simulink model "tracking_model"  (R2017a)
(part 4 of 14)

8076211353316)-(x_9.^2.*cos(x_4).*sin(x_3).^4.*sin(x_4).^3.*2.19560928610309e-18)./(cos(x_3).^4.*9.05902758e-4+sin(x_3).^4.*9.05902758e-4+cos(x_3).^2.*sin(x_3).^2.*1.811805516e-3)-(x_9.^2.*cos(x_5).*sin(x_3).^4.*sin(x_5).^3.*2.19560928610309e-18)./(cos(x_3).^4.*9.05902758e-4+sin(x_3).^4.*9.05902758e-4+cos(x_3).^2.*sin(x_3).^2.*1.811805516e-3)+(x_9.^2.*cos(x_6).*sin(x_3).^4.*sin(x_6).^3.*4.39121857220618e-18)./(cos(x_3).^4.*9.05902758e-4+sin(x_3).^4.*9.05902758e-4+cos(x_3).^2.*sin(x_3).^2.*1.811805516e-3)+(x_7.*x_9.*cos(x_4).*sin(x_3).^3.*sin(x_4).*4.361535375749998e-7)./(cos(x_3).^2.*6.49519052838329e-1+sin(x_3).^2.*6.49519052838329e-1)-(x_7.*x_9.*cos(x_5).*sin(x_3).^3.*sin(x_5).*2.180767687874999e-7)./(cos(x_3).^2.*6.49519052838329e-1+sin(x_3).^2.*6.49519052838329e-1)+(x_8.*x_9.*cos(x_5).*sin(x_3).^3.*sin(x_5).*3.777200434904005e-7)./(cos(x_3).^2.*6.49519052838329e-1+sin(x_3).^2.*6.49519052838329e-1)-(x_7.*x_9.*cos(x_6).*sin(x_3).^3.*sin(x_6).*2.180767687874999e-7)./(cos(x_3).^2.*6.49519052838329e-1+sin(x_3).^2.*6.49519052838329e-1)-(x_8.*x_9.*cos(x_6).*sin(x_3).^3.*sin(x_6).*3.777200434904005e-7)./(cos(x_3).^2.*6.49519052838329e-1+sin(x_3).^2.*6.49519052838329e-1)-(x_9.^2.*sin(x_4.*2.0).*cos(x_3).^2.*sin(x_3).^2.*sin(x_4).^2.*1.837631161344131e-20)./(cos(x_3).^4.*3.79080679921875e-6+sin(x_3).^4.*3.79080679921875e-6+cos(x_3).^4.*cos(x_4).^2.*6.757062187003037e-11+cos(x_3).^4.*cos(x_5).^2.*6.757062187003037e-11+cos(x_3).^4.*cos(x_6).^2.*6.757062187003037e-11+cos(x_3).^2.*sin(x_3).^2.*7.5816135984375e-6+cos(x_4).^2.*sin(x_3).^4.*6.757062187003037e-11+cos(x_5).^2.*sin(x_3).^4.*6.757062187003037e-11+cos(x_6).^2.*sin(x_3).^4.*6.757062187003037e-11+cos(x_3).^2.*cos(x_4).^2.*sin(x_3).^2.*1.351412437400607e-10+cos(x_3).^2.*cos(x_5).^2.*sin(x_3).^2.*1.351412437400607e-10+cos(x_3).^2.*cos(x_6).^2.*sin(x_3).^2.*1.351412437400607e-10)-(x_9.^2.*sin(x_4.*2.0).*cos(x_3).^2.*sin(x_3).^2.*sin(x_5).^2.*1.837631161344131e-20)./(cos(x_3).^4.*3.79080679921875e-6+sin(x_3).^4.*3.79080679921875e-6+cos(x_3).^4.*cos(x_4).^2.*6.757062187003037e-11+cos(x_3).^4.*cos(x_5).^2.*6.757062187003037e-11+cos(x_3).^4.*cos(x_6).^2.*6.757062187003037e-11+cos(x_3).^2.*sin(x_3).^2.*7.5816135984375e-6+cos(x_4).^2.*sin(x_3).^4.*6.757062187003037e-11+cos(x_5).^2.*sin(x_3).^4.*6.757062187003037e-11+cos(x_6).^2.*sin(x_3).^4.*6.757062187003037e-11+cos(x_3).^2.*cos(x_4).^2.*sin(x_3).^2.*1.351412437400607e-10+cos(x_3).^2.*cos(x_5).^2.*sin(x_3).^2.*1.351412437400607e-10+cos(x_3).^2.*cos(x_6).^2.*sin(x_3).^2.*1.351412437400607e-10)-(x_9.^2.*sin(x_5.*2.0).*cos(x_3).^2.*sin(x_3).^2.*sin(x_4).^2.*1.837631161344131e-20)./(cos(x_3).^4.*3.79080679921875e-6+sin(x_3).^4.*3.79080679921875e-6+cos(x_3).^4.*cos(x_4).^2.*6.757062187003037e-11+cos(x_3).^4.*cos(x_5).^2.*6.757062187003037e-11+cos(x_3).^4.*cos(x_6).^2.*6.757062187003037e-11+cos(x_3).^2.*sin(x_3).^2.*7.5816135984375e-6+cos(x_4).^2.*sin(x_3).^4.*6.757062187003037e-11+cos(x_5).^2.*sin(x_3).^4.*6.757062187003037e-11+cos(x_6).^2.*sin(x_3).^4.*6.757062187003037e-11+cos(x_3).^2.*cos(x_4).^2.*sin(x_3).^2.*1.351412437400607e-10+cos(x_3).^2.*cos(x_5).^2.*sin(x_3).^2.*1.351412437400607e-10+cos(x_3).^2.*cos(x_6).^2.*sin(x_3).^2.*1.351412437400607e-10)+(x_9.^2.*sin(x_4.*2.0).*cos(x_3).^2.*sin(x_3).^2.*sin(x_4).^4.*1.637688852754318e-25)./(cos(x_3).^4.*3.79080679921875e-6+sin(x_3).^4.*3.79080679921875e-6+cos(x_3).^4.*cos(x_4).^2.*6.757062187003037e-11+cos(x_3).^4.*cos(x_5).^2.*6.757062187003037e-11+cos(x_3).^4.*cos(x_6).^2.*6.757062187003037e-11+cos(x_3).^2.*sin(x_3).^2.*7.5816135984375e-6+cos(x_4).^2.*sin(x_3).^4.*6.757062187003037e-11+cos(x_5).^2.*sin(x_3).^4.*6.757062187003037e-11+cos(x_6).^2.*sin(x_3).^4.*6.757062187003037e-11+cos(x_3).^2.*cos(x_4).^2.*sin(x_3).^2.*1.351412437400607e-10+cos(x_3).^2.*cos(x_5).^2.*sin(x_3).^2.*1.351412437400607e-10+cos(x_3).^2.*cos(x_6).^2.*sin(x_3).^2.*1.351412437400607e-10)-(x_9.^2.*sin(x_4.*2.0).*cos(x_3).^2.*sin(x_3).^2.*sin(x_6).^2.*1.837631161344131e-20)./(cos(x_3).^4.*3.79080679921875e-6+sin(x_3).^4.*3.79080679921875e-6+cos(x_3).^4.*cos(x_4).^2.*6.757062187003037e-11+cos(x_3).^4.*cos(x_5).^2.*6.757062187003037e-11+cos(x_3).^4.*cos(x_6).^2.*6.757062187003037e-11+cos(x_3).^2.*sin(x_3).^2.*7.5816135984375e-6+cos(x_4).^2.*sin(x_3).^4.*6.757062187003037e-11+cos(x_5).^2.*sin(x_3).^4.*6.757062187003037e-11+cos(x_6).^2.*sin(x_3).^4.*6.757062187003037e-11+cos(x_3).^2.*cos(x_4).^2.*sin(x_3).^2.*1.351412437400607e-10+cos(x_3).^2.*cos(x_5).^2.*sin(x_3).^2.*1.351412437400607e-10+cos(x_3).^2.*cos(x_6).^2.*sin(x_3).^2.*1.351412437400607e-10)-(x_9.^2.*sin(x_5.*2.0).*cos(x_3).^2.*sin(x_3).^2.*sin(x_5).^2.*1.837631161344131e-20)./(cos(x_3).^4.*3.79080679921875e-6+sin(x_3).^4.*3.79080679921875e-6+cos(x_3).^4.*cos(x_4).^2.*6.757062187003037e-11+cos(x_3).^4.*cos(x_5).^2.*6.757062187003037e-11+cos(x_3).^4.*cos(x_6).^2.*6.757062187003037e-11+cos(x_3).^2.*sin(x_3).^2.*7.5816135984375e-6+cos(x_4).^2.*sin(x_3).^4.*6.757062187003037e-11+cos(x_5).^2.*sin(x_3).^4.*6.757062187003037e-11+cos(x_6).^2.*sin(x_3).^4.*6.757062187003037e-11+cos(x_3).^2.*cos(x_4).^2.*sin(x_3).^2.*1.351412437400607e-10+cos(x_3).^2.*cos(x_5).^2.*sin(x_3).^2.*1.351412437400607e-10+cos(x_3).^2.*cos(x_6).^2.*sin(x_3).^2.*1.351412437400607e-10)-(x_9.^2.*sin(x_6.*2.0).*cos(x_3).^2.*sin(x_3).^2.*sin(x_4).^2.*1.837631161344131e-20)./(cos(x_3).^4.*3.79080679921875e-6+sin(x_3).^4.*3.79080679921875e-6+cos(x_3).^4.*cos(x_4).^2.*6.757062187003037e-11+cos(x_3).^4.*cos(x_5).^2.*6.757062187003037e-11+cos(x_3).^4.*cos(x_6).^2.*6.757062187003037e-11+cos(x_3).^2.*sin(x_3).^2.*7.5816135984375e-6+cos(x_4).^2.*sin(x_3).^4.*6.757062187003037e-11+cos(x_5).^2.*sin(x_3).^4.*6.757062187003037e-11+cos(x_6).^2.*sin(x_3).^4.*6.757062187003037e-11+cos(x_3).^2.*cos(x_4).^2.*sin(x_3).^2.*1.351412437400607e-10+cos(x_3).^2.*cos(x_5).^2.*sin(x_3).^2.*1.351412437400607e-10+cos(x_3).^2.*cos(x_6).^2.*sin(x_3).^2.*1.351412437400607e-10)+(x_9.^2.*sin(x_4.*2.0).*cos(x_3).^2.*sin(x_3).^2.*sin(x_5).^4.*1.637688852754318e-25)./(cos(x_3).^4.*3.79080679921875e-6+sin(x_3).^4.*3.79080679921875e-6+cos(x_3).^4.*cos(x_4).^2.*6.757062187003037e-11+cos(x_3).^4.*cos(x_5).^2.*6.757062187003037e-11+cos(x_3).^4.*cos(x_6).^2.*6.757062187003037e-11+cos(x_3).^2.*sin(x_3).^2.*7.5816135984375e-6+cos(x_4).^2.*sin(x_3).^4.*6.757062187003037e-11+cos(x_5).^2.*sin(x_3).^4.*6.757062187003037e-11+cos(x_6).^2.*sin(x_3).^4.*6.757062187003037e-11+cos(x_3).^2.*cos(x_4).^2.*sin(x_3).^2.*1.351412437400607e-10+cos(x_3).^2.*cos(x_5).^2.*sin(x_3).^2.*1.351412437400607e-10+cos(x_3).^2.*cos(x_6).^2.*sin(x_3).^2.*1.351412437400607e-10)+(x_9.^2.*sin(x_5.*2.0).*cos(x_3).^2.*sin(x_3).^2.*sin(x_4).^4.*1.637688852754318e-25)./(cos(x_3).^4.*3.79080679921875e-6+sin(x_3).^4.*3.79080679921875e-6+cos(x_3).^4.*cos(x_4).^2.*6.757062187003037e-11+cos(x_3).^4.*cos(x_5).^2.*6.757062187003037e-11+cos(x_3).^4.*cos(x_6).^2.*6.757062187003037e-11+cos(x_3).^2.*sin(x_3).^2.*7.5816135984375e-6+cos(x_4).^2.*sin(x_3).^4.*6.757062187003037e-11+cos(x_5).^2.*sin(x_3).^4.*6.757062187003037e-11+cos(x_6).^2.*sin(x_3).^4.*6.757062187003037e-11+cos(x_3).^2.*cos(x_4).^2.*sin(x_3).^2.*1.351412437400607e-10+cos(x_3).^2.*cos(x_5).^2.*sin(x_3).^2.*1.351412437400607e-10+cos(x_3).^2.*cos(x_6).^2.*sin(x_3).^2.*1.351412437400607e-10)-(x_9.^2.*sin(x_5.*2.0).*cos(x_3).^2.*sin(x_3).^2.*sin(x_6).^2.*1.837631161344131e-20)./(cos(x_3).^4.*3.79080679921875e-6+sin(x_3).^4.*3.79080679921875e-6+cos(x_3).^4.*cos(x_4).^2.*6.757062187003037e-11+cos(x_3).^4.*cos(x_5).^2.*6.757062187003037e-11+cos(x_3).^4.*cos(x_6).^2.*6.757062187003037e-11+cos(x_3).^2.*sin(x_3).^2.*7.5816135984375e-6+cos(x_4).^2.*sin(x_3).^4.*6.757062187003037e-11+cos(x_5).^2.*sin(x_3).^4.*6.757062187003037e-11+cos(x_6).^2.*sin(x_3).^4.*6.757062187003037e-11+cos(x_3).^2.*cos(x_4).^2.*sin(x_3).^2.*1.351412437400607e-10+cos(x_3).^2.*cos(x_5).^2.*sin(x_3).^2.*1.351412437400607e-10+cos(x_3).^2.*cos(x_6).^2.*sin(x_3).^2.*1.351412437400607e-10)-(x_9.^2.*sin(x_6.*2.0).*cos(x_3).^2.*sin(x_3).^2.*sin(x_5).^2.*1.837631161344131e-20)./(cos(x_3).^4.*3.79080679921875e-6+sin(x_3).^4.*3.79080679921875e-6+cos(x_3).^4.*cos(x_4).^2.*6.757062187003037e-11+cos(x_3).^4.*cos(x_5).^2.*6.757062187003037e-11+cos(x_3).^4.*cos(x_6).^2.*6.757062187003037e-11+cos(x_3).^2.*sin(x_3).^2.*7.5816135984375e-6+cos(x_4).^2.*sin(x_3).^4.*6.757062187003037e-11+cos(x_5).^2.*sin(x_3).^4.*6.757062187003037e-11+cos(x_6).^2.*sin(x_3).^4.*6.757062187003037e-11+cos(x_3).^2.*cos(x_4).^2.*sin(x_3).^2.*1.351412437400607e-10+cos(x_3).^2.*cos(x_5).^2.*sin(x_3).^2.*1.351412437400607e-10+cos(x_3).^2.*cos(x_6).^2.*sin(x_3).^2.*1.351412437400607e-10)+(x_9.^2.*sin(x_4.*2.0).*cos(x_3).^2.*sin(x_3).^2.*sin(x_6).^4.*1.637688852754318e-25)./(cos(x_3).^4.*3.79080679921875e-6+sin(x_3).^4.*3.79080679921875e-6+cos(x_3).^4.*cos(x_4).^2.*6.757062187003037e-11+cos(x_3).^4.*cos(x_5).^2.*6.757062187003037e-11+cos(x_3).^4.*cos(x_6).^2.*6.757062187003037e-11+cos(x_3).^2.*sin(x_3).^2.*7.5816135984375e-6+cos(x_4).^2.*sin(x_3).^4.*6.757062187003037e-11+cos(x_5).^2.*sin(x_3).^4.*6.757062187003037e-11+cos(x_6).^2.*sin(x_3).^4.*6.757062187003037e-11+cos(x_3).^2.*cos(x_4).^2.*sin(x_3).^2.*1.351412437400607e-10+cos(x_3).^2.*cos(x_5).^2.*sin(x_3).^2.*1.351412437400607e-10+cos(x_3).^2.*cos(x_6).^2.*sin(x_3).^2.*1.351412437400607e-10)+(x_9.^2.*sin(x_4.*2.0).*cos(x_3).^4.*sin(x_4).^2.*sin(x_5).^2.*1.637688852754318e-25)./(cos(x_3).^4.*3.79080679921875e-6+sin(x_3).^4.*3.79080679921875e-6+cos(x_3).^4.*cos(x_4).^2.*6.757062187003037e-11+cos(x_3).^4.*cos(x_5).^2.*6.757062187003037e-11+cos(x_3).^4.*cos(x_6).^2.*6.757062187003037e-11+cos(x_3).^2.*sin(x_3).^2.*7.5816135984375e-6+cos(x_4).^2.*sin(x_3).^4.*6.757062187003037e-11+cos(x_5).^2.*sin(x_3).^4.*6.757062187003037e-11+cos(x_6).^2.*sin(x_3).^4.*6.757062187003037e-11+cos(x_3).^2.*cos(x_4).^2.*sin(x_3).^2.*1.351412437400607e-10+cos(x_3).^2.*cos(x_5).^2.*sin(x_3).^2.*1.351412437400607e-10+cos(x_3).^2.*cos(x_6).^2.*sin(x_3).^2.*1.351412437400607e-10)+(x_9.^2.*sin(x_5.*2.0).*cos(x_3).^2.*sin(x_3).^2.*sin(x_5).^4.*1.637688852754318e-25)./(cos(x_3).^4.*3.79080679921875e-6+sin(x_3).^4.*3.79080679921875e-6+cos(x_3).^4.*cos(x_4).^2.*6.757062187003037e-11+cos(x_3).^4.*cos(x_5).^2.*6.757062187003037e-11+cos(x_3).^4.*cos(x_6).^2.*6.757062187003037e-11+cos(x_3).^2.*sin(x_3).^2.*7.5816135984375e-6+cos(x_4).^2.*sin(x_3).^4.*6.757062187003037e-11+cos(x_5).^2.*sin(x_3).^4.*6.757062187003037e-11+cos(x_6).^2.*sin(x_3).^4.*6.757062187003037e-11+cos(x_3).^2.*cos(x_4).^2.*sin(x_3).^2.*1.351412437400607e-10+cos(x_3).^2.*cos(x_5).^2.*sin(x_3).^2.*1.351412437400607e-10+cos(x_3).^2.*cos(x_6).^2.*sin(x_3).^2.*1.351412437400607e-10)+(x_9.^2.*sin(x_6.*2.0).*cos(x_3).^2.*sin(x_3).^2.*sin(x_4).^4.*1.637688852754318e-25)./(cos(x_3).^4.*3.79080679921875e-6+sin(x_3).^4.*3.79080679921875e-6+cos(x_3).^4.*cos(x_4).^2.*6.757062187003037e-11+cos(x_3).^4.*cos(x_5).^2.*6.757062187003037e-11+cos(x_3).^4.*cos(x_6).^2.*6.757062187003037e-11+cos(x_3).^2.*sin(x_3).^2.*7.5816135984375e-6+cos(x_4).^2.*sin(x_3).^4.*6.757062187003037e-11+cos(x_5).^2.*sin(x_3).^4.*6.757062187003037e-11+cos(x_6).^2.*sin(x_3).^4.*6.757062187003037e-11+cos(x_3).^2.*cos(x_4).^2.*sin(x_3).^2.*1.351412437400607e-10+cos(x_3).^2.*cos(x_5).^2.*sin(x_3).^2.*1.351412437400607e-10+cos(x_3).^2.*cos(x_6).^2.*sin(x_3).^2.*1.351412437400607e-10)-(x_9.^2.*sin(x_6.*2.0).*cos(x_3).^2.*sin(x_3).^2.*sin(x_6).^2.*1.837631161344131e-20)./(cos(x_3).^4.*3.79080679921875e-6+sin(x_3).^4.*3.79080679921875e-6+cos(x_3).^4.*cos(x_4).^2.*6.757062187003037e-11+cos(x_3).^4.*cos(x_5).^2.*6.757062187003037e-11+cos(x_3).^4.*cos(x_6).^2.*6.757062187003037e-11+cos(x_3).^2.*sin(x_3).^2.*7.5816135984375e-6+cos(x_4).^2.*sin(x_3).^4.*6.757062187003037e-11+cos(x_5).^2.*sin(x_3).^4.*6.757062187003037e-11+cos(x_6).^2.*sin(x_3).^4.*6.757062187003037e-11+cos(x_3).^2.*cos(x_4).^2.*sin(x_3).^2.*1.351412437400607e-10+cos(x_3).^2.*cos(x_5).^2.*sin(x_3).^2.*1.351412437400607e-10+cos(x_3).^2.*cos(x_6).^2.*sin(x_3).^2.*1.351412437400607e-10)+(x_9.^2.*sin(x_4.*2.0).*cos(x_3).^4.*sin(x_4).^2.*sin(x_6).^2.*1.637688852754318e-25)./(cos(x_3).^4.*3.79080679921875e-6+sin(x_3).^4.*3.79080679921875e-6+cos(x_3).^4.*cos(x_4).^2.*6.757062187003037e-11+cos(x_3).^4.*cos(x_5).^2.*6.757062187003037e-11+cos(x_3).^4.*cos(x_6).^2.*6.757062187003037e-11+cos(x_3).^2.*sin(x_3).^2.*7.5816135984375e-6+cos(x_4).^2.*sin(x_3).^4.*6.757062187003037e-11+cos(x_5).^2.*sin(x_3).^4.*6.757062187003037e-11+cos(x_6).^2.*sin(x_3).^4.*6.757062187003037e-11+cos(x_3).^2.*cos(x_4).^2.*sin(x_3).^2.*1.351412437400607e-10+cos(x_3).^2.*cos(x_5).^2.*sin(x_3).^2.*1.351412437400607e-10+cos(x_3).^2.*cos(x_6).^2.*sin(x_3).^2.*1.351412437400607e-10)+(x_9.^2.*sin(x_5.*2.0).*cos(x_3).^2.*sin(x_3).^2.*sin(x_6).^4.*1.637688852754318e-25)./(cos(x_3).^4.*3.79080679921875e-6+sin(x_3).^4.*3.79080679921875e-6+cos(x_3).^4.*cos(x_4).^2.*6.757062187003037e-11+cos(x_3).^4.*cos(x_5).^2.*6.757062187003037e-11+cos(x_3).^4.*cos(x_6).^2.*6.757062187003037e-11+cos(x_3).^2.*sin(x_3).^2.*7.5816135984375e-6+cos(x_4).^2.*sin(x_3).^4.*6.757062187003037e-11+cos(x_5).^2.*sin(x_3).^4.*6.757062187003037e-11+cos(x_6).^2.*sin(x_3).^4.*6.757062187003037e-11+cos(x_3).^2.*cos(x_4).^2.*sin(x_3).^2.*1.351412437400607e-10+cos(x_3).^2.*cos(x_5).^2.*sin(x_3).^2.*1.351412437400607e-10+cos(x_3).^2.*cos(x_6).^2.*sin(x_3).^2.*1.351412437400607e-10)+(x_9.^2.*sin(x_5.*2.0).*cos(x_3).^4.*sin(x_4).^2.*sin(x_5).^2.*1.637688852754318e-25)./(cos(x_3).^4.*3.79080679921875e-6+sin(x_3).^4.*3.79080679921875e-6+cos(x_3).^4.*cos(x_4).^2.*6.757062187003037e-11+cos(x_3).^4.*cos(x_5).^2.*6.757062187003037e-11+cos(x_3).^4.*cos(x_6).^2.*6.757062187003037e-11+cos(x_3).^2.*sin(x_3).^2.*7.5816135984375e-6+cos(x_4).^2.*sin(x_3).^4.*6.757062187003037e-11+cos(x_5).^2.*sin(x_3).^4.*6.757062187003037e-11+cos(x_6).^2.*sin(x_3).^4.*6.757062187003037e-11+cos(x_3).^2.*cos(x_4).^2.*sin(x_3).^2.*1.351412437400607e-10+cos(x_3).^2.*cos(x_5).^2.*sin(x_3).^2.*1.351412437400607e-10+cos(x_3).^2.*cos(x_6).^2.*sin(x_3).^2.*1.351412437400607e-10)+(x_9.^2.*sin(x_6.*2.0).*cos(x_3).^2.*sin(x_3).^2.*sin(x_5).^4.*1.637688852754318e-25)./(cos(x_3).^4.*3.79080679921875e-6+sin(x_3).^4.*3.79080679921875e-6+cos(x_3).^4.*cos(x_4).^2.*6.757062187003037e-11+cos(x_3).^4.*cos(x_5).^2.*6.757062187003037e-11+cos(x_3).^4.*cos(x_6).^2.*6.757062187003037e-11+cos(x_3).^2.*sin(x_3).^2.*7.5816135984375e-6+cos(x_4).^2.*sin(x_3).^4.*6.757062187003037e-11+cos(x_5).^2.*sin(x_3).^4.*6.757062187003037e-11+cos(x_6).^2.*sin(x_3).^4.*6.757062187003037e-11+cos(x_3).^2.*cos(x_4).^2.*sin(x_3).^2.*1.351412437400607e-10+cos(x_3).^2.*cos(x_5).^2.*sin(x_3).^2.*1.351412437400607e-10+cos(x_3).^2.*cos(x_6).^2.*sin(x_3).^2.*1.351412437400607e-10)+(x_9.^2.*sin(x_4.*2.0).*cos(x_3).^4.*sin(x_5).^2.*sin(x_6).^2.*1.637688852754318e-25)./(cos(x_3).^4.*3.79080679921875e-6+sin(x_3).^4.*3.79080679921875e-6+cos(x_3).^4.*cos(x_4).^2.*6.757062187003037e-11+cos(x_3).^4.*cos(x_5).^2.*6.757062187003037e-11+cos(x_3).^4.*cos(x_6).^2.*6.757062187003037e-11+cos(x_3).^2.*sin(x_3).^2.*7.5816135984375e-6+cos(x_4).^2.*sin(x_3).^4.*6.757062187003037e-11+cos(x_5).^2.*sin(x_3).^4.*6.757062187003037e-11+cos(x_6).^2.*sin(x_3).^4.*6.757062187003037e-11+cos(x_3).^2.*cos(x_4).^2.*sin(x_3).^2.*1.351412437400607e-10+cos(x_3).^2.*cos(x_5).^2.*sin(x_3).^2.*1.351412437400607e-10+cos(x_3).^2.*cos(x_6).^2.*sin(x_3).^2.*1.351412437400607e-10)+(x_9.^2.*sin(x_5.*2.0).*cos(x_3).^4.*sin(x_4).^2.*sin(x_6).^2.*1.637688852754318e-25)./(cos(x_3).^4.*3.79080679921875e-6+sin(x_3).^4.*3.79080679921875e-6+cos(x_3).^4.*cos(x_4).^2.*6.757062187003037e-11+cos(x_3).^4.*cos(x_5).^2.*6.757062187003037e-11+cos(x_3).^4.*cos(x_6).^2.*6.757062187003037e-11+cos(x_3).^2.*sin(x_3).^2.*7.5816135984375e-6+cos(x_4).^2.*sin(x_3).^4.*6.757062187003037e-11+cos(x_5).^2.*sin(x_3).^4.*6.757062187003037e-11+cos(x_6).^2.*sin(x_3).^4.*6.757062187003037e-11+cos(x_3).^2.*cos(x_4).^2.*sin(x_3).^2.*1.351412437400607e-10+cos(x_3).^2.*cos(x_5).^2.*sin(x_3).^2.*1.351412437400607e-10+cos(x_3).^2.*cos(x_6).^2.*sin(x_3).^2.*1.351412437400607e-10)+(x_9.^2.*sin(x_6.*2.0).*cos(x_3).^2.*sin(x_3).^2.*sin(x_6).^4.*1.637688852754318e-25)./(cos(x_3).^4.*3.79080679921875e-6+sin(x_3).^4.*3.79080679921875e-6+cos(x_3).^4.*cos(x_4).^2.*6.757062187003037e-11+cos(x_3).^4.*cos(x_5).^2.*6.757062187003037e-11+cos(x_3).^4.*cos(x_6).^2.*6.757062187003037e-11+cos(x_3).^2.*sin(x_3).^2.*7.5816135984375e-6+cos(x_4).^2.*sin(x_3).^4.*6.757062187003037e-11+cos(x_5).^2.*sin(x_3).^4.*6.757062187003037e-11+cos(x_6).^2.*sin(x_3).^4.*6.757062187003037e-11+cos(x_3).^2.*cos(x_4).^2.*sin(x_3).^2.*1.351412437400607e-10+cos(x_3).^2.*cos(x_5).^2.*sin(x_3).^2.*1.351412437400607e-10+cos(x_3).^2.*cos(x_6).^2.*sin(x_3).^2.*1.351412437400607e-10)+(x_9.^2.*sin(x_6.*2.0).*cos(x_3).^4.*sin(x_4).^2.*sin(x_5).^2.*1.637688852754318e-25)./(cos(x_3).^4.*3.79080679921875e-6+sin(x_3).^4.*3.79080679921875e-6+cos(x_3).^4.*cos(x_4).^2.*6.757062187003037e-11+cos(x_3).^4.*cos(x_5).^2.*6.757062187003037e-11+cos(x_3).^4.*cos(x_6).^2.*6.757062187003037e-11+cos(x_3).^2.*sin(x_3).^2.*7.5816135984375e-6+cos(x_4).^2.*sin(x_3).^4.*6.757062187003037e-11+cos(x_5).^2.*sin(x_3).^4.*6.757062187003037e-11+cos(x_6).^2.*sin(x_3).^4.*6.757062187003037e-11+cos(x_3).^2.*cos(x_4).^2.*sin(x_3).^2.*1.351412437400607e-10+cos(x_3).^2.*cos(x_5).^2.*sin(x_3).^2.*1.351412437400607e-10+cos(x_3).^2.*cos(x_6).^2.*sin(x_3).^2.*1.351412437400607e-10)+(x_9.^2.*sin(x_5.*2.0).*cos(x_3).^4.*sin(x_5).^2.*sin(x_6).^2.*1.637688852754318e-25)./(cos(x_3).^4.*3.79080679921875e-6+sin(x_3).^4.*3.79080679921875e-6+cos(x_3).^4.*cos(x_4).^2.*6.757062187003037e-11+cos(x_3).^4.*cos(x_5).^2.*6.757062187003037e-11+cos(x_3).^4.*cos(x_6).^2.*6.757062187003037e-11+cos(x_3).^2.*sin(x_3).^2.*7.5816135984375e-6+cos(x_4).^2.*sin(x_3).^4.*6.757062187003037e-11+cos(x_5).^2.*sin(x_3).^4.*6.757062187003037e-11+cos(x_6).^2.*sin(x_3).^4.*6.757062187003037e-11+cos(x_3).^2.*cos(x_4).^2.*sin(x_3).^2.*1.351412437400607e-10+cos(x_3).^2.*cos(x_5).^2.*sin(x_3).^2.*1.351412437400607e-10+cos(x_3).^2.*cos(x_6).^2.*sin(x_3).^2.*1.351412437400607e-10)+(x_9.^2.*sin(x_6.*2.0).*cos(x_3).^4.*sin(x_4).^2.*sin(x_6).^2.*1.637688852754318e-25)./(cos(x_3).^4.*3.79080679921875e-6+sin(x_3).^4.*3.79080679921875e-6+cos(x_3).^4.*cos(x_4).^2.*6.757062187003037e-11+cos(x_3).^4.*cos(x_5).^2.*6.757062187003037e-11+cos(x_3).^4.*cos(x_6).^2.*6.757062187003037e-11+cos(x_3).^2.*sin(x_3).^2.*7.5816135984375e-6+cos(x_4).^2.*sin(x_3).^4.*6.757062187003037e-11+cos(x_5).^2.*sin(x_3).^4.*6.757062187003037e-11+cos(x_6).^2.*sin(x_3).^4.*6.757062187003037e-11+cos(x_3).^2.*cos(x_4).^2.*sin(x_3).^2.*1.351412437400607e-10+cos(x_3).^2.*cos(x_5).^2.*sin(x_3).^2.*1.351412437400607e-10+cos(x_3).^2.*cos(x_6).^2.*sin(x_3).^2.*1.351412437400607e-10)+(x_9.^2.*sin(x_6.*2.0).*cos(x_3).^4.*sin(x_5).^2.*sin(x_6).^2.*1.637688852754318e-25)./(cos(x_3).^4.*3.79080679921875e-6+sin(x_3).^4.*3.79080679921875e-6+cos(x_3).^4.*cos(x_4).^2.*6.757062187003037e-11+cos(x_3).^4.*cos(x_5).^2.*6.757062187003037e-11+cos(x_3).^4.*cos(x_6).^2.*6.757062187003037e-11+cos(x_3).^2.*sin(x_3).^2.*7.5816135984375e-6+cos(x_4).^2.*sin(x_3).^4.*6.757062187003037e-11+cos(x_5).^2.*sin(x_3).^4.*6.757062187003037e-11+cos(x_6).^2.*sin(x_3).^4.*6.757062187003037e-11+cos(x_3).^2.*cos(x_4).^2.*sin(x_3).^2.*1.351412437400607e-10+cos(x_3).^2.*cos(x_5).^2.*sin(x_3).^2.*1.351412437400607e-10+cos(x_3).^2.*cos(x_6).^2.*sin(x_3).^2.*1.351412437400607e-10)-(x_9.^2.*cos(x_3).^2.*cos(x_4).*sin(x_3).^2.*sin(x_4).^3.*4.39121857220618e-18)./(cos(x_3).^4.*9.05902758e-4+sin(x_3).^4.*9.05902758e-4+cos(x_3).^2.*sin(x_3).^2.*1.811805516e-3)-(x_9.^2.*cos(x_3).^2.*cos(x_5).*sin(x_3).^2.*sin(x_5).^3.*4.39121857220618e-18)./(cos(x_3).^4.*9.05902758e-4+sin(x_3).^4.*9.05902758e-4+cos(x_3).^2.*sin(x_3).^2.*1.811805516e-3)+(x_9.^2.*cos(x_3).^2.*cos(x_6).*sin(x_3).^2.*sin(x_6).^3.*8.782437144412361e-18)./(cos(x_3).^4.*9.05902758e-4+sin(x_3).^4.*9.05902758e-4+cos(x_3).^2.*sin(x_3).^2.*1.811805516e-3)+(x_9.^2.*sin(x_4.*2.0).*sin(x_3).^4.*sin(x_4).^2.*sin(x_5).^2.*1.637688852754318e-25)./(cos(x_3).^4.*3.79080679921875e-6+sin(x_3).^4.*3.79080679921875e-6+cos(x_3).^4.*cos(x_4).^2.*6.757062187003037e-11+cos(x_3).^4.*cos(x_5).^2.*6.757062187003037e-11+cos(x_3).^4.*cos(x_6).^2.*6.757062187003037e-11+cos(x_3).^2.*sin(x_3).^2.*7.5816135984375e-6+cos(x_4).^2.*sin(x_3).^4.*6.757062187003037e-11+cos(x_5).^2.*sin(x_3).^4.*6.757062187003037e-11+cos(x_6).^2.*sin(x_3).^4.*6.757062187003037e-11+cos(x_3).^2.*cos(x_4).^2.*sin(x_3).^2.*1.351412437400607e-10+cos(x_3).^2.*cos(x_5).^2.*sin(x_3).^2.*1.351412437400607e-10+cos(x_3).^2.*cos(x_6).^2.*sin(x_3).^2.*1.351412437400607e-10)+(x_9.^2.*sin(x_4.*2.0).*sin(x_3).^4.*sin(x_4).^2.*sin(x_6).^2.*1.637688852754318e-25)./(cos(x_3).^4.*3.79080679921875e-6+sin(x_3).^4.*3.79080679921875e-6+cos(x_3).^4.*cos(x_4).^2.*6.757062187003037e-11+cos(x_3).^4.*cos(x_5).^2.*6.757062187003037e-11+cos(x_3).^4.*cos(x_6).^2.*6.757062187003037e-11+cos(x_3).^2.*sin(x_3).^2.*7.5816135984375e-6+cos(x_4).^2.*sin(x_3).^4.*6.757062187003037e-11+cos(x_5).^2.*sin(x_3).^4.*6.757062187003037e-11+cos(x_6).^2.*sin(x_3).^4.*6.757062187003037e-11+cos(x_3).^2.*cos(x_4).^2.*sin(x_3).^2.*1.351412437400607e-10+cos(x_3).^2.*cos(x_5).^2.*sin(x_3).^2.*1.351412437400607e-10+cos(x_3).^2.*cos(x_6).^2.*sin(x_3).^2.*1.351412437400607e-10)+(x_9.^2.*sin(x_5.*2.0).*sin(x_3).^4.*sin(x_4).^2.*sin(x_5).^2.*1.637688852754318e-25)./(cos(x_3).^4.*3.79080679921875e-6+sin(x_3).^4.*3.79080679921875e-6+cos(x_3).^4.*cos(x_4).^2.*6.757062187003037e-11+cos(x_3).^4.*cos(x_5).^2.*6.757062187003037e-11+cos(x_3).^4.*cos(x_6).^2.*6.757062187003037e-11+cos(x_3).^2.*sin(x_3).^2.*7.5816135984375e-6+cos(x_4).^2.*sin(x_3).^4.*6.757062187003037e-11+cos(x_5).^2.*sin(x_3).^4.*6.757062187003037e-11+cos(x_6).^2.*sin(x_3).^4.*6.757062187003037e-11+cos(x_3).^2.*cos(x_4).^2.*sin(x_3).^2.*1.351412437400607e-10+cos(x_3).^2.*cos(x_5).^2.*sin(x_3).^2.*1.351412437400607e-10+cos(x_3).^2.*cos(x_6).^2.*sin(x_3).^2.*1.351412437400607e-10)+(x_9.^2.*sin(x_4.*2.0).*sin(x_3).^4.*sin(x_5).^2.*sin(x_6).^2.*1.637688852754318e-25)./(cos(x_3).^4.*3.79080679921875e-6+sin(x_3).^4.*3.79080679921875e-6+cos(x_3).^4.*cos(x_4).^2.*6.757062187003037e-11+cos(x_3).^4.*cos(x_5).^2.*6.757062187003037e-11+cos(x_3).^4.*cos(x_6).^2.*6.757062187003037e-11+cos(x_3).^2.*sin(x_3).^2.*7.5816135984375e-6+cos(x_4).^2.*sin(x_3).^4.*6.757062187003037e-11+cos(x_5).^2.*sin(x_3).^4.*6.757062187003037e-11+cos(x_6).^2.*sin(x_3).^4.*6.757062187003037e-11+cos(x_3).^2.*cos(x_4).^2.*sin(x_3).^2.*1.351412437400607e-10+cos(x_3).^2.*cos(x_5).^2.*sin(x_3).^2.*1.351412437400607e-10+cos(x_3).^2.*cos(x_6).^2.*sin(x_3).^2.*1.351412437400607e-10)+(x_9.^2.*sin(x_5.*2.0).*sin(x_3).^4.*sin(x_4).^2.*sin(x_6).^2.*1.637688852754318e-25)./(cos(x_3).^4.*3.79080679921875e-6+sin(x_3).^4.*3.79080679921875e-6+cos(x_3).^4.*cos(x_4).^2.*6.757062187003037e-11+cos(x_3).^4.*cos(x_5).^2.*6.757062187003037e-11+cos(x_3).^4.*cos(x_6).^2.*6.757062187003037e-11+cos(x_3).^2.*sin(x_3).^2.*7.5816135984375e-6+cos(x_4).^2.*sin(x_3).^4.*6.757062187003037e-11+cos(x_5).^2.*sin(x_3).^4.*6.757062187003037e-11+cos(x_6).^2.*sin(x_3).^4.*6.757062187003037e-11+cos(x_3).^2.*cos(x_4).^2.*sin(x_3).^2.*1.351412437400607e-10+cos(x_3).^2.*cos(x_5).^2.*sin(x_3).^2.*1.351412437400607e-10+cos(x_3).^2.*cos(x_6).^2.*sin(x_3).^2.*1.351412437400607e-10)+(x_9.^2.*sin(x_6.*2.0).*sin(x_3).^4.*sin(x_4).^2.*sin(x_5).^2.*1.637688852754318e-25)./(cos(x_3).^4.*3.79080679921875e-6+sin(x_3).^4.*3.79080679921875e-6+cos(x_3).^4.*cos(x_4).^2.*6.757062187003037e-11+cos(x_3).^4.*cos(x_5).^2.*6.757062187003037e-11+cos(x_3).^4.*cos(x_6).^2.*6.757062187003037e-11+cos(x_3).^2.*sin(x_3).^2.*7.5816135984375e-6+cos(x_4).^2.*sin(x_3).^4.*6.757062187003037e-11+cos(x_5).^2.*sin(x_3).^4.*6.757062187003037e-11+cos(x_6).^2.*sin(x_3).^4.*6.757062187003037e-11+cos(x_3).^2.*cos(x_4).^2.*sin(x_3).^2.*1.351412437400607e-10+cos(x_3).^2.*cos(x_5).^2.*sin(x_3).^2.*1.351412437400607e-10+cos(x_3).^2.*cos(x_6).^2.*sin(x_3).^2.*1.351412437400607e-10)+(x_9.^2.*sin(x_5.*2.0).*sin(x_3).^4.*sin(x_5).^2.*sin(x_6).^2.*1.637688852754318e-25)./(cos(x_3).^4.*3.79080679921875e-6+sin(x_3).^4.*3.79080679921875e-6+cos(x_3).^4.*cos(x_4).^2.*6.757062187003037e-11+cos(x_3).^4.*cos(x_5).^2.*6.757062187003037e-11+cos(x_3).^4.*cos(x_6).^2.*6.757062187003037e-11+cos(x_3).^2.*sin(x_3).^2.*7.5816135984375e-6+cos(x_4).^2.*sin(x_3).^4.*6.757062187003037e-11+cos(x_5).^2.*sin(x_3).^4.*6.757062187003037e-11+cos(x_6).^2.*sin(x_3).^4.*6.757062187003037e-11+cos(x_3).^2.*cos(x_4).^2.*sin(x_3).^2.*1.351412437400607e-10+cos(x_3).^2.*cos(x_5).^2.*sin(x_3).^2.*1.351412437400607e-10+cos(x_3).^2.*cos(x_6).^2.*sin(x_3).^2.*1.351412437400607e-10)+(x_9.^2.*sin(x_6.*2.0).*sin(x_3).^4.*sin(x_4).^2.*sin(x_6).^2.*1.637688852754318e-25)./(cos(x_3).^4.*3.79080679921875e-6+sin(x_3).^4.*3.79080679921875e-6+cos(x_3).^4.*cos(x_4).^2.*6.757062187003037e-11+cos(x_3).^4.*cos(x_5).^2.*6.757062187003037e-11+cos(x_3).^4.*cos(x_6).^2.*6.757062187003037e-11+cos(x_3).^2.*sin(x_3).^2.*7.5816135984375e-6+cos(x_4).^2.*sin(x_3).^4.*6.757062187003037e-11+cos(x_5).^2.*sin(x_3).^4.*6.757062187003037e-11+cos(x_6).^2.*sin(x_3).^4.*6.757062187003037e-11+cos(x_3).^2.*cos(x_4).^2.*sin(x_3).^2.*1.351412437400607e-10+cos(x_3).^2.*cos(x_5).^2.*sin(x_3).^2.*1.351412437400607e-10+cos(x_3).^2.*cos(x_6).^2.*sin(x_3).^2.*1.351412437400607e-10)+(x_9.^2.*sin(x_6.*2.0).*sin(x_3).^4.*sin(x_5).^2.*sin(x_6).^2.*1.637688852754318e-25)./(cos(x_3).^4.*3.79080679921875e-6+sin(x_3).^4.*3.79080679921875e-6+cos(x_3).^4.*cos(x_4).^2.*6.757062187003037e-11+cos(x_3).^4.*cos(x_5).^2.*6.757062187003037e-11+cos(x_3).^4.*cos(x_6).^2.*6.757062187003037e-11+cos(x_3).^2.*sin(x_3).^2.*7.5816135984375e-6+cos(x_4).^2.*sin(x_3).^4.*6.757062187003037e-11+cos(x_5).^2.*sin(x_3).^4.*6.757062187003037e-11+cos(x_6).^2.*sin(x_3).^4.*6.757062187003037e-11+cos(x_3).^2.*cos(x_4).^2.*sin(x_3).^2.*1.351412437400607e-10+cos(x_3).^2.*cos(x_5).^2.*sin(x_3).^2.*1.351412437400607e-10+cos(x_3).^2.*cos(x_6).^2.*sin(x_3).^2.*1.351412437400607e-10)-(x_8.*x_9.*cos(x_3).^5.*cos(x_4).*sin(x_4).^3.*1.470104929075305e-19)./(cos(x_3).^4.*3.79080679921875e-6+sin(x_3).^4.*3.79080679921875e-6+cos(x_3).^4.*cos(x_4).^2.*6.757062187003037e-11+cos(x_3).^4.*cos(x_5).^2.*6.757062187003037e-11+cos(x_3).^4.*cos(x_6).^2.*6.757062187003037e-11+cos(x_3).^2.*sin(x_3).^2.*7.5816135984375e-6+cos(x_4).^2.*sin(x_3).^4.*6.757062187003037e-11+cos(x_5).^2.*sin(x_3).^4.*6.757062187003037e-11+cos(x_6).^2.*sin(x_3).^4.*6.757062187003037e-11+cos(x_3).^2.*cos(x_4).^2.*sin(x_3).^2.*1.351412437400607e-10+cos(x_3).^2.*cos(x_5).^2.*sin(x_3).^2.*1.351412437400607e-10+cos(x_3).^2.*cos(x_6).^2.*sin(x_3).^2.*1.351412437400607e-10)+(x_7.*x_9.*cos(x_3).^5.*cos(x_5).*sin(x_5).^3.*1.273148214807934e-19)./(cos(x_3).^4.*3.79080679921875e-6+sin(x_3).^4.*3.79080679921875e-6+cos(x_3).^4.*cos(x_4).^2.*6.757062187003037e-11+cos(x_3).^4.*cos(x_5).^2.*6.757062187003037e-11+cos(x_3).^4.*cos(x_6).^2.*6.757062187003037e-11+cos(x_3).^2.*sin(x_3).^2.*7.5816135984375e-6+cos(x_4).^2.*sin(x_3).^4.*6.757062187003037e-11+cos(x_5).^2.*sin(x_3).^4.*6.757062187003037e-11+cos(x_6).^2.*sin(x_3).^4.*6.757062187003037e-11+cos(x_3).^2.*cos(x_4).^2.*sin(x_3).^2.*1.351412437400607e-10+cos(x_3).^2.*cos(x_5).^2.*sin(x_3).^2.*1.351412437400607e-10+cos(x_3).^2.*cos(x_6).^2.*sin(x_3).^2.*1.351412437400607e-10)+(x_8.*x_9.*cos(x_3).^5.*cos(x_4).*sin(x_4).^5.*1.310151082203454e-24)./(cos(x_3).^4.*3.79080679921875e-6+sin(x_3).^4.*3.79080679921875e-6+cos(x_3).^4.*cos(x_4).^2.*6.757062187003037e-11+cos(x_3).^4.*cos(x_5).^2.*6.757062187003037e-11+cos(x_3).^4.*cos(x_6).^2.*6.757062187003037e-11+cos(x_3).^2.*sin(x_3).^2.*7.5816135984375e-6+cos(x_4).^2.*sin(x_3).^4.*6.757062187003037e-11+cos(x_5).^2.*sin(x_3).^4.*6.757062187003037e-11+cos(x_6).^2.*sin(x_3).^4.*6.757062187003037e-11+cos(x_3).^2.*cos(x_4).^2.*sin(x_3).^2.*1.351412437400607e-10+cos(x_3).^2.*cos(x_5).^2.*sin(x_3).^2.*1.351412437400607e-10+cos(x_3).^2.*cos(x_6).^2.*sin(x_3).^2.*1.351412437400607e-10)+(x_8.*x_9.*cos(x_3).^5.*cos(x_5).*sin(x_5).^3.*7.350524645376524e-20)./(cos(x_3).^4.*3.79080679921875e-6+sin(x_3).^4.*3.79080679921875e-6+cos(x_3).^4.*cos(x_4).^2.*6.757062187003037e-11+cos(x_3).^4.*cos(x_5).^2.*6.757062187003037e-11+cos(x_3).^4.*cos(x_6).^2.*6.757062187003037e-11+cos(x_3).^2.*sin(x_3).^2.*7.5816135984375e-6+cos(x_4).^2.*sin(x_3).^4.*6.757062187003037e-11+cos(x_5).^2.*sin(x_3).^4.*6.757062187003037e-11+cos(x_6).^2.*sin(x_3).^4.*6.757062187003037e-11+cos(x_3).^2.*cos(x_4).^2.*sin(x_3).^2.*1.351412437400607e-10+cos(x_3).^2.*cos(x_5).^2.*sin(x_3).^2.*1.351412437400607e-10+cos(x_3).^2.*cos(x_6).^2.*sin(x_3).^2.*1.351412437400607e-10)-(x_7.*x_9.*cos(x_3).^5.*cos(x_5).*sin(x_5).^5.*1.134624119983866e-24)./(cos(x_3).^4.*3.79080679921875e-6+sin(x_3).^4.*3.79080679921875e-6+cos(x_3).^4.*cos(x_4).^2.*6.757062187003037e-11+cos(x_3).^4.*cos(x_5).^2.*6.757062187003037e-11+cos(x_3).^4.*cos(x_6).^2.*6.757062187003037e-11+cos(x_3).^2.*sin(x_3).^2.*7.5816135984375e-6+cos(x_4).^2.*sin(x_3).^4.*6.757062187003037e-11+cos(x_5).^2.*sin(x_3).^4.*6.757062187003037e-11+cos(x_6).^2.*sin(x_3).^4.*6.757062187003037e-11+cos(x_3).^2.*cos(x_4).^2.*sin(x_3).^2.*1.351412437400607e-10+cos(x_3).^2.*cos(x_5).^2.*sin(x_3).^2.*1.351412437400607e-10+cos(x_3).^2.*cos(x_6).^2.*sin(x_3).^2.*1.351412437400607e-10)-(x_7.*x_9.*cos(x_3).^5.*cos(x_6).*sin(x_6).^3.*1.273148214807934e-19)./(cos(x_3).^4.*3.79080679921875e-6+sin(x_3).^4.*3.79080679921875e-6+cos(x_3).^4.*cos(x_4).^2.*6.757062187003037e-11+cos(x_3).^4.*cos(x_5).^2.*6.757062187003037e-11+cos(x_3).^4.*cos(x_6).^2.*6.757062187003037e-11+cos(x_3).^2.*sin(x_3).^2.*7.5816135984375e-6+cos(x_4).^2.*sin(x_3).^4.*6.757062187003037e-11+cos(x_5).^2.*sin(x_3).^4.*6.757062187003037e-11+cos(x_6).^2.*sin(x_3).^4.*6.757062187003037e-11+cos(x_3).^2.*cos(x_4).^2.*sin(x_3).^2.*1.351412437400607e-10+cos(x_3).^2.*cos(x_5).^2.*sin(x_3).^2.*1.351412437400607e-10+cos(x_3).^2.*cos(x_6).^2.*sin(x_3).^2.*1.351412437400607e-10)-(x_8.*x_9.*cos(x_3).^5.*cos(x_5).*sin(x_5).^5.*6.550755411017271e-25)./(cos(x_3).^4.*3.79080679921875e-6+sin(x_3).^4.*3.79080679921875e-6+cos(x_3).^4.*cos(x_4).^2.*6.757062187003037e-11+cos(x_3).^4.*cos(x_5).^2.*6.757062187003037e-11+cos(x_3).^4.*cos(x_6).^2.*6.757062187003037e-11+cos(x_3).^2.*sin(x_3).^2.*7.5816135984375e-6+cos(x_4).^2.*sin(x_3).^4.*6.757062187003037e-11+cos(x_5).^2.*sin(x_3).^4.*6.757062187003037e-11+cos(x_6).^2.*sin(x_3).^4.*6.757062187003037e-11+cos(x_3).^2.*cos(x_4).^2.*sin(x_3).^2.*1.351412437400607e-10+cos(x_3).^2.*cos(x_5).^2.*sin(x_3).^2.*1.351412437400607e-10+cos(x_3).^2.*cos(x_6).^2.*sin(x_3).^2.*1.351412437400607e-10)+(x_8.*x_9.*cos(x_3).^5.*cos(x_6).*sin(x_6).^3.*7.350524645376524e-20)./(cos(x_3).^4.*3.79080679921875e-6+sin(x_3).^4.*3.79080679921875e-6+cos(x_3).^4.*cos(x_4).^2.*6.757062187003037e-11+cos(x_3).^4.*cos(x_5).^2.*6.757062187003037e-11+cos(x_3).^4.*cos(x_6).^2.*6.757062187003037e-11+cos(x_3).^2.*sin(x_3).^2.*7.5816135984375e-6+cos(x_4).^2.*sin(x_3).^4.*6.757062187003037e-11+cos(x_5).^2.*sin(x_3).^4.*6.757062187003037e-11+cos(x_6).^2.*sin(x_3).^4.*6.757062187003037e-11+cos(x_3).^2.*cos(x_4).^2.*sin(x_3).^2.*1.351412437400607e-10+cos(x_3).^2.*cos(x_5).^2.*sin(x_3).^2.*1.351412437400607e-10+cos(x_3).^2.*cos(x_6).^2.*sin(x_3).^2.*1.351412437400607e-10)+(x_7.*x_9.*cos(x_3).^5.*cos(x_6).*sin(x_6).^5.*1.134624119983866e-24)./(cos(x_3).^4.*3.79080679921875e-6+sin(x_3).^4.*3.79080679921875e-6+cos(x_3).^4.*cos(x_4).^2.*6.757062187003037e-11+cos(x_3).^4.*cos(x_5).^2.*6.757062187003037e-11+cos(x_3).^4.*cos(x_6).^2.*6.757062187003037e-11+cos(x_3).^2.*sin(x_3).^2.*7.5816135984375e-6+cos(x_4).^2.*sin(x_3).^4.*6.757062187003037e-11+cos(x_5).^2.*sin(x_3).^4.*6.757062187003037e-11+cos(x_6).^2.*sin(x_3).^4.*6.757062187003037e-11+cos(x_3).^2.*cos(x_4).^2.*sin(x_3).^2.*1.351412437400607e-10+cos(x_3).^2.*cos(x_5).^2.*sin(x_3).^2.*1.351412437400607e-10+cos(x_3).^2.*cos(x_6).^2.*sin(x_3).^2.*1.351412437400607e-10)-(x_8.*x_9.*cos(x_3).^5.*cos(x_6).*sin(x_6).^5.*6.550755411017271e-25)./(cos(x_3).^4.*3.79080679921875e-6+sin(x_3).^4.*3.79080679921875e-6+cos(x_3).^4.*cos(x_4).^2.*6.757062187003037e-11+cos(x_3).^4.*cos(x_5).^2.*6.757062187003037e-11+cos(x_3).^4.*cos(x_6).^2.*6.757062187003037e-11+cos(x_3).^2.*sin(x_3).^2.*7.5816135984375e-6+cos(x_4).^2.*sin(x_3).^4.*6.757062187003037e-11+cos(x_5).^2.*sin(x_3).^4.*6.757062187003037e-11+cos(x_6).^2.*sin(x_3).^4.*6.757062187003037e-11+cos(x_3).^2.*cos(x_4).^2.*sin(x_3).^2.*1.351412437400607e-10+cos(x_3).^2.*cos(x_5).^2.*sin(x_3).^2.*1.351412437400607e-10+cos(x_3).^2.*cos(x_6).^2.*sin(x_3).^2.*1.351412437400607e-10)-(x_8.*x_9.*cos(x_3).^4.*cos(x_4).*sin(x_4).^3.*4.39121857220618e-18)./(cos(x_3).^4.*1.5163227196875e-5+sin(x_3).^4.*1.5163227196875e-5+cos(x_3).^4.*cos(x_4).^2.*2.702824874801215e-10+cos(x_3).^4.*cos(x_5).^2.*2.702824874801215e-10+cos(x_3).^4.*cos(x_6).^2.*2.702824874801215e-10+cos(x_3).^2.*sin(x_3).^2.*3.032645439375e-5+cos(x_4).^2.*sin(x_3).^4.*2.702824874801215e-10+cos(x_5).^2.*sin(x_3).^4.*2.702824874801215e-10+cos(x_6).^2.*sin(x_3).^4.*2.702824874801215e-10+cos(x_3).^2.*cos(x_4).^2.*sin(x_3).^2.*5.40564974960243e-10+cos(x_3).^2.*cos(x_5).^2.*sin(x_3).^2.*5.40564974960243e-10+cos(x_3).^2.*cos(x_6).^2.*sin(x_3).^2.*5.40564974960243e-10)+(x_7.*x_9.*cos(x_3).^4.*cos(x_5).*sin(x_5).^3.*3.802906837100583e-18)./(cos(x_3).^4.*1.5163227196875e-5+sin(x_3).^4.*1.5163227196875e-5+cos(x_3).^4.*cos(x_4).^2.*2.702824874801215e-10+cos(x_3).^4.*cos(x_5).^2.*2.702824874801215e-10+cos(x_3).^4.*cos(x_6).^2.*2.702824874801215e-10+cos(x_3).^2.*sin(x_3).^2.*3.032645439375e-5+cos(x_4).^2.*sin(x_3).^4.*2.702824874801215e-10+cos(x_5).^2.*sin(x_3).^4.*2.702824874801215e-10+cos(x_6).^2.*sin(x_3).^4.*2.702824874801215e-10+cos(x_3).^2.*cos(x_4).^2.*sin(x_3).^2.*5.40564974960243e-10+cos(x_3).^2.*cos(x_5).^2.*sin(x_3).^2.*5.40564974960243e-10+cos(x_3).^2.*cos(x_6).^2.*sin(x_3).^2.*5.40564974960243e-10)+(x_8.*x_9.*cos(x_3).^4.*cos(x_5).*sin(x_5).^3.*2.19560928610309e-18)./(cos(x_3).^4.*1.5163227196875e-5+sin(x_3).^4.*1.5163227196875e-5+cos(x_3).^4.*cos(x_4).^2.*2.702824874801215e-10+cos(x_3).^4.*cos(x_5).^2.*2.702824874801215e-10+cos(x_3).^4.*cos(x_6).^2.*2.702824874801215e-10+cos(x_3).^2.*sin(x_3).^2.*3.032645439375e-5+cos(x_4).^2.*sin(x_3).^4.*2.702824874801215e-10+cos(x_5).^2.*sin(x_3).^4.*2.702824874801215e-10+cos(x_6).^2.*sin(x_3).^4.*2.702824874801215e-10+cos(x_3).^2.*cos(x_4).^2.*sin(x_3).^2.*5.40564974960243e-10+cos(x_3).^2.*cos(x_5).^2.*sin(x_3).^2.*5.40564974960243e-10+cos(x_3).^2.*cos(x_6).^2.*sin(x_3).^2.*5.40564974960243e-10)-(x_7.*x_9.*cos(x_3).^4.*cos(x_6).*sin(x_6).^3.*3.802906837100583e-18)./(cos(x_3).^4.*1.5163227196875e-5+sin(x_3).^4.*1.5163227196875e-5+cos(x_3).^4.*cos(x_4).^2.*2.702824874801215e-10+cos(x_3).^4.*cos(x_5).^2.*2.702824874801215e-10+cos(x_3).^4.*cos(x_6).^2.*2.702824874801215e-10+cos(x_3).^2.*sin(x_3).^2.*3.032645439375e-5+cos(x_4).^2.*sin(x_3).^4.*2.702824874801215e-10+cos(x_5).^2.*sin(x_3).^4.*2.702824874801215e-10+cos(x_6).^2.*sin(x_3).^4.*2.702824874801215e-10+cos(x_3).^2.*cos(x_4).^2.*sin(x_3).^2.*5.40564974960243e-10+cos(x_3).^2.*cos(x_5).^2.*sin(x_3).^2.*5.40564974960243e-10+cos(x_3).^2.*cos(x_6).^2.*sin(x_3).^2.*5.40564974960243e-10)+(x_8.*x_9.*cos(x_3).^4.*cos(x_6).*sin(x_6).^3.*2.19560928610309e-18)./(cos(x_3).^4.*1.5163227196875e-5+sin(x_3).^4.*1.5163227196875e-5+cos(x_3).^4.*cos(x_4).^2.*2.702824874801215e-10+cos(x_3).^4.*cos(x_5).^2.*2.702824874801215e-10+cos(x_3).^4.*cos(x_6).^2.*2.702824874801215e-10+cos(x_3).^2.*sin(x_3).^2.*3.032645439375e-5+cos(x_4).^2.*sin(x_3).^4.*2.702824874801215e-10+cos(x_5).^2.*sin(x_3).^4.*2.702824874801215e-10+cos(x_6).^2.*sin(x_3).^4.*2.702824874801215e-10+cos(x_3).^2.*cos(x_4).^2.*sin(x_3).^2.*5.40564974960243e-10+cos(x_3).^2.*cos(x_5).^2.*sin(x_3).^2.*5.40564974960243e-10+cos(x_3).^2.*cos(x_6).^2.*sin(x_3).^2.*5.40564974960243e-10)+(x_7.*x_9.*cos(x_4).*sin(x_3).^5.*sin(x_4).^3.*1.470104929075305e-19)./(cos(x_3).^4.*3.79080679921875e-6+sin(x_3).^4.*3.79080679921875e-6+cos(x_3).^4.*cos(x_4).^2.*6.757062187003037e-11+cos(x_3).^4.*cos(x_5).^2.*6.757062187003037e-11+cos(x_3).^4.*cos(x_6).^2.*6.757062187003037e-11+cos(x_3).^2.*sin(x_3).^2.*7.5816135984375e-6+cos(x_4).^2.*sin(x_3).^4.*6.757062187003037e-11+cos(x_5).^2.*sin(x_3).^4.*6.757062187003037e-11+cos(x_6).^2.*sin(x_3).^4.*6.757062187003037e-11+cos(x_3).^2.*cos(x_4).^2.*sin(x_3).^2.*1.351412437400607e-10+cos(x_3).^2.*cos(x_5).^2.*sin(x_3).^2.*1.351412437400607e-10+cos(x_3).^2.*cos(x_6).^2.*sin(x_3).^2.*1.351412437400607e-10)-(x_7.*x_9.*cos(x_4).*sin(x_3).^5.*sin(x_4).^5.*1.310151082203454e-24)./(cos(x_3).^4.*3.79080679921875e-6+sin(x_3).^4.*3.79080679921875e-6+cos(x_3).^4.*cos(x_4).^2.*6.757062187003037e-11+cos(x_3).^4.*cos(x_5).^2.*6.757062187003037e-11+cos(x_3).^4.*cos(x_6).^2.*6.757062187003037e-11+cos(x_3).^2.*sin(x_3).^2.*7.5816135984375e-6+cos(x_4).^2.*sin(x_3).^4.*6.757062187003037e-11+cos(x_5).^2.*sin(x_3).^4.*6.757062187003037e-11+cos(x_6).^2.*sin(x_3).^4.*6.757062187003037e-11+cos(x_3).^2.*cos(x_4).^2.*sin(x_3).^2.*1.351412437400607e-10+cos(x_3).^2.*cos(x_5).^2.*sin(x_3).^2.*1.351412437400607e-10+cos(x_3).^2.*cos(x_6).^2.*sin(x_3).^2.*1.351412437400607e-10)-(x_7.*x_9.*cos(x_5).*sin(x_3).^5.*sin(x_5).^3.*7.350524645376524e-20)./(cos(x_3).^4.*3.79080679921875e-6+sin(x_3).^4.*3.79080679921875e-6+cos(x_3).^4.*cos(x_4).^2.*6.757062187003037e-11+cos(x_3).^4.*cos(x_5).^2.*6.757062187003037e-11+cos(x_3).^4.*cos(x_6).^2.*6.757062187003037e-11+cos(x_3).^2.*sin(x_3).^2.*7.5816135984375e-6+cos(x_4).^2.*sin(x_3).^4.*6.757062187003037e-11+cos(x_5).^2.*sin(x_3).^4.*6.757062187003037e-11+cos(x_6).^2.*sin(x_3).^4.*6.757062187003037e-11+cos(x_3).^2.*cos(x_4).^2.*sin(x_3).^2.*1.351412437400607e-10+cos(x_3).^2.*cos(x_5).^2.*sin(x_3).^2.*1.351412437400607e-10+cos(x_3).^2.*cos(x_6).^2.*sin(x_3).^2.*1.351412437400607e-10)+(x_8.*x_9.*cos(x_5).*sin(x_3).^5.*sin(x_5).^3.*1.273148214807934e-19)./(cos(x_3).^4.*3.79080679921875e-6+sin(x_3).^4.*3.79080679921875e-6+cos(x_3).^4.*cos(x_4).^2.*6.757062187003037e-11+cos(x_3).^4.*cos(x_5).^2.*6.757062187003037e-11+cos(x_3).^4.*cos(x_6).^2.*6.757062187003037e-11+cos(x_3).^2.*sin(x_3).^2.*7.5816135984375e-6+cos(x_4).^2.*sin(x_3).^4.*6.757062187003037e-11+cos(x_5).^2.*sin(x_3).^4.*6.757062187003037e-11+cos(x_6).^2.*sin(x_3).^4.*6.757062187003037e-11+cos(x_3).^2.*cos(x_4).^2.*sin(x_3).^2.*1.351412437400607e-10+cos(x_3).^2.*cos(x_5).^2.*sin(x_3).^2.*1.351412437400607e-10+cos(x_3).^2.*cos(x_6).^2.*sin(x_3).^2.*1.351412437400607e-10)+(x_7.*x_9.*cos(x_5).*sin(x_3).^5.*sin(x_5).^5.*6.550755411017271e-25)./(cos(x_3).^4.*3.79080679921875e-6+sin(x_3).^4.*3.79080679921875e-6+cos(x_3).^4.*cos(x_4).^2.*6.757062187003037e-11+cos(x_3).^4.*cos(x_5).^2.*6.757062187003037e-11+cos(x_3).^4.*cos(x_6).^2.*6.757062187003037e-11+cos(x_3).^2.*sin(x_3).^2.*7.5816135984375e-6+cos(x_4).^2.*sin(x_3).^4.*6.757062187003037e-11+cos(x_5).^2.*sin(x_3).^4.*6.757062187003037e-11+cos(x_6).^2.*sin(x_3).^4.*6.757062187003037e-11+cos(x_3).^2.*cos(x_4).^2.*sin(x_3).^2.*1.351412437400607e-10+cos(x_3).^2.*cos(x_5).^2.*sin(x_3).^2.*1.351412437400607e-10+cos(x_3).^2.*cos(x_6).^2.*sin(x_3).^2.*1.351412437400607e-10)-(x_7.*x_9.*cos(x_6).*sin(x_3).^5.*sin(x_6).^3.*7.350524645376524e-20)./(cos(x_3).^4.*3.79080679921875e-6+sin(x_3).^4.*3.79080679921875e-6+cos(x_3).^4.*cos(x_4).^2.*6.757062187003037e-11+cos(x_3).^4.*cos(x_5).^2.*6.757062187003037e-11+cos(x_3).^4.*cos(x_6).^2.*6.757062187003037e-11+cos(x_3).^2.*sin(x_3).^2.*7.5816135984375e-6+cos(x_4).^2.*sin(x_3).^4.*6.757062187003037e-11+cos(x_5).^2.*sin(x_3).^4.*6.757062187003037e-11+cos(x_6).^2.*sin(x_3).^4.*6.757062187003037e-11+cos(x_3).^2.*cos(x_4).^2.*sin(x_3).^2.*1.351412437400607e-10+cos(x_3).^2.*cos(x_5).^2.*sin(x_3).^2.*1.351412437400607e-10+cos(x_3).^2.*cos(x_6).^2.*sin(x_3).^2.*1.351412437400607e-10)-(x_8.*x_9.*cos(x_5).*sin(x_3).^5.*sin(x_5).^5.*1.134624119983866e-24)./(cos(x_3).^4.*3.79080679921875e-6+sin(x_3).^4.*3.79080679921875e-6+cos(x_3).^4.*cos(x_4).^2.*6.757062187003037e-11+cos(x_3).^4.*cos(x_5).^2.*6.757062187003037e-11+cos(x_3).^4.*cos(x_6).^2.*6.757062187003037e-11+cos(x_3).^2.*sin(x_3).^2.*7.5816135984375e-6+cos(x_4).^2.*sin(x_3).^4.*6.757062187003037e-11+cos(x_5).^2.*sin(x_3).^4.*6.757062187003037e-11+cos(x_6).^2.*sin(x_3).^4.*6.757062187003037e-11+cos(x_3).^2.*cos(x_4).^2.*sin(x_3).^2.*1.351412437400607e-10+cos(x_3).^2.*cos(x_5).^2.*sin(x_3).^2.*1.351412437400607e-10+cos(x_3).^2.*cos(x_6).^2.*sin(x_3).^2.*1.351412437400607e-10)-(x_8.*x_9.*cos(x_6).*sin(x_3).^5.*sin(x_6).^3.*1.273148214807934e-19)./(cos(x_3).^4.*3.79080679921875e-6+sin(x_3).^4.*3.79080679921875e-6+cos(x_3).^4.*cos(x_4).^2.*6.757062187003037e-11+cos(x_3).^4.*cos(x_5).^2.*6.757062187003037e-11+cos(x_3).^4.*cos(x_6).^2.*6.757062187003037e-11+cos(x_3).^2.*sin(x_3).^2.*7.5816135984375e-6+cos(x_4).^2.*sin(x_3).^4.*6.757062187003037e-11+cos(x_5).^2.*sin(x_3).^4.*6.757062187003037e-11+cos(x_6).^2.*sin(x_3).^4.*6.757062187003037e-11+cos(x_3).^2.*cos(x_4).^2.*sin(x_3).^2.*1.351412437400607e-10+cos(x_3).^2.*cos(x_5).^2.*sin(x_3).^2.*1.351412437400607e-10+cos(x_3).^2.*cos(x_6).^2.*sin(x_3).^2.*1.351412437400607e-10)+(x_7.*x_9.*cos(x_6).*sin(x_3).^5.*sin(x_6).^5.*6.550755411017271e-25)./(cos(x_3).^4.*3.79080679921875e-6+sin(x_3).^4.*3.79080679921875e-6+cos(x_3).^4.*cos(x_4).^2.*6.757062187003037e-11+cos(x_3).^4.*cos(x_5).^2.*6.757062187003037e-11+cos(x_3).^4.*cos(x_6).^2.*6.757062187003037e-11+cos(x_3).^2.*sin(x_3).^2.*7.5816135984375e-6+cos(x_4).^2.*sin(x_3).^4.*6.757062187003037e-11+cos(x_5).^2.*sin(x_3).^4.*6.757062187003037e-11+cos(x_6).^2.*sin(x_3).^4.*6.757062187003037e-11+cos(x_3).^2.*cos(x_4).^2.*sin(x_3).^2.*1.351412437400607e-10+cos(x_3).^2.*cos(x_5).^2.*sin(x_3).^2.*1.351412437400607e-10+cos(x_3).^2.*cos(x_6).^2.*sin(x_3).^2.*1.351412437400607e-10)+(x_8.*x_9.*cos(x_6).*sin(x_3).^5.*sin(x_6).^5.*1.134624119983866e-24)./(cos(x_3).^4.*3.79080679921875e-6+sin(x_3).^4.*3.79080679921875e-6+cos(x_3).^4.*cos(x_4).^2.*6.757062187003037e-11+cos(x_3).^4.*cos(x_5).^2.*6.757062187003037e-11+cos(x_3).^4.*cos(x_6).^2.*6.757062187003037e-11+cos(x_3).^2.*sin(x_3).^2.*7.5816135984375e-6+cos(x_4).^2.*sin(x_3).^4.*6.757062187003037e-11+cos(x_5).^2.*sin(x_3).^4.*6.757062187003037e-11+cos(x_6).^2.*sin(x_3).^4.*6.757062187003037e-11+cos(x_3).^2.*cos(x_4).^2.*sin(x_3).^2.*1.351412437400607e-10+cos(x_3).^2.*cos(x_5).^2.*sin(x_3).^2.*1.351412437400607e-10+cos(x_3).^2.*cos(x_6).^2.*sin(x_3).^2.*1.351412437400607e-10)-(x_7.*x_9.*cos(x_4).*sin(x_3).^4.*sin(x_4).^3.*4.39121857220618e-18)./(cos(x_3).^4.*1.5163227196875e-5+sin(x_3).^4.*1.5163227196875e-5+cos(x_3).^4.*cos(x_4).^2.*2.702824874801215e-10+cos(x_3).^4.*cos(x_5).^2.*2.702824874801215e-10+cos(x_3).^4.*cos(x_6).^2.*2.702824874801215e-10+cos(x_3).^2.*sin(x_3).^2.*3.032645439375e-5+cos(x_4).^2.*sin(x_3).^4.*2.702824874801215e-10+cos(x_5).^2.*sin(x_3).^4.*2.702824874801215e-10+cos(x_6).^2.*sin(x_3).^4.*2.702824874801215e-10+cos(x_3).^2.*cos(x_4).^2.*sin(x_3).^2.*5.40564974960243e-10+cos(x_3).^2.*cos(x_5).^2.*sin(x_3).^2.*5.40564974960243e-10+cos(x_3).^2.*cos(x_6).^2.*sin(x_3).^2.*5.40564974960243e-10)+(x_7.*x_9.*cos(x_5).*sin(x_3).^4.*sin(x_5).^3.*2.19560928610309e-18)./(cos(x_3).^4.*1.5163227196875e-5+sin(x_3).^4.*1.5163227196875e-5+cos(x_3).^4.*cos(x_4).^2.*2.702824874801215e-10+cos(x_3).^4.*cos(x_5).^2.*2.702824874801215e-10+cos(x_3).^4.*cos(x_6).^2.*2.702824874801215e-10+cos(x_3).^2.*sin(x_3).^2.*3.032645439375e-5+cos(x_4).^2.*sin(x_3).^4.*2.702824874801215e-10+cos(x_5).^2.*sin(x_3).^4.*2.702824874801215e-10+cos(x_6).^2.*sin(x_3).^4.*2.702824874801215e-10+cos(x_3).^2.*cos(x_4).^2.*sin(x_3).^2.*5.40564974960243e-10+cos(x_3).^2.*cos(x_5).^2.*sin(x_3).^2.*5.40564974960243e-10+cos(x_3).^2.*cos(x_6).^2.*sin(x_3).^2.*5.40564974960243e-10)-(x_8.*x_9.*cos(x_5).*sin(x_3).^4.*sin(x_5).^3.*3.802906837100583e-18)./(cos(x_3).^4.*1.5163227196875e-5+sin(x_3).^4.*1.5163227196875e-5+cos(x_3).^4.*cos(x_4).^2.*2.702824874801215e-10+cos(x_3).^4.*cos(x_5).^2.*2.702824874801215e-10+cos(x_3).^4.*cos(x_6).^2.*2.702824874801215e-10+cos(x_3).^2.*sin(x_3).^2.*3.032645439375e-5+cos(x_4).^2.*sin(x_3).^4.*2.702824874801215e-10+cos(x_5).^2.*sin(x_3).^4.*2.702824874801215e-10+cos(x_6).^2.*sin(x_3).^4.*2.702824874801215e-10+cos(x_3).^2.*cos(x_4).^2.*sin(x_3).^2.*5.40564974960243e-10+cos(x_3).^2.*cos(x_5).^2.*sin(x_3).^2.*5.40564974960243e-10+cos(x_3).^2.*cos(x_6).^2.*sin(x_3).^2.*5.40564974960243e-10)+(x_7.*x_9.*cos(x_6).*sin(x_3).^4.*sin(x_6).^3.*2.19560928610309e-18)./(cos(x_3).^4.*1.5163227196875e-5+sin(x_3).^4.*1.5163227196875e-5+cos(x_3).^4.*cos(x_4).^2.*2.702824874801215e-10+cos(x_3).^4.*cos(x_5).^2.*2.702824874801215e-10+cos(x_3).^4.*cos(x_6).^2.*2.702824874801215e-10+cos(x_3).^2.*sin(x_3).^2.*3.032645439375e-5+cos(x_4).^2.*sin(x_3).^4.*2.702824874801215e-10+cos(x_5).^2.*sin(x_3).^4.*2.702824874801215e-10+cos(x_6).^2.*sin(x_3).^4.*2.702824874801215e-10+cos(x_3).^2.*cos(x_4).^2.*sin(x_3).^2.*5.40564974960243e-10+cos(x_3).^2.*cos(x_5).^2.*sin(x_3).^2.*5.40564974960243e-10+cos(x_3).^2.*cos(x_6).^2.*sin(x_3).^2.*5.40564974960243e-10)+(x_8.*x_9.*cos(x_6).*sin(x_3).^4.*sin(x_6).^3.*3.802906837100583e-18)./(cos(x_3).^4.*1.5163227196875e-5+sin(x_3).^4.*1.5163227196875e-5+cos(x_3).^4.*cos(x_4).^2.*2.702824874801215e-10+cos(x_3).^4.*cos(x_5).^2.*2.702824874801215e-10+cos(x_3).^4.*cos(x_6).^2.*2.702824874801215e-10+cos(x_3).^2.*sin(x_3).^2.*3.032645439375e-5+cos(x_4).^2.*sin(x_3).^4.*2.702824874801215e-10+cos(x_5).^2.*sin(x_3).^4.*2.702824874801215e-10+cos(x_6).^2.*sin(x_3).^4.*2.702824874801215e-10+cos(x_3).^2.*cos(x_4).^2.*sin(x_3).^2.*5.40564974960243e-10+cos(x_3).^2.*cos(x_5).^2.*sin(x_3).^2.*5.40564974960243e-10+cos(x_3).^2.*cos(x_6).^2.*sin(x_3).^2.*5.40564974960243e-10)+(x_9.^2.*cos(x_3).*cos(x_4).*sin(x_3).^2.*sin(x_4).*7.358998824951566e-12)./(cos(x_3).^4.*3.623611032e-3+sin(x_3).^4.*3.623611032e-3+cos(x_3).^2.*sin(x_3).^2.*7.247222064e-3)+(x_9.^2.*cos(x_3).^2.*cos(x_4).*sin(x_3).*sin(x_4).*1.471799764990313e-11)./(cos(x_3).^4.*3.623611032e-3+sin(x_3).^4.*3.623611032e-3+cos(x_3).^2.*sin(x_3).^2.*7.247222064e-3)-(x_9.^2.*cos(x_3).*cos(x_5).*sin(x_3).^2.*sin(x_5).*1.471799764990313e-11)./(cos(x_3).^4.*3.623611032e-3+sin(x_3).^4.*3.623611032e-3+cos(x_3).^2.*sin(x_3).^2.*7.247222064e-3)-(x_9.^2.*cos(x_3).^2.*cos(x_5).*sin(x_3).*sin(x_5).*7.358998824951566e-12)./(cos(x_3).^4.*3.623611032e-3+sin(x_3).^4.*3.623611032e-3+cos(x_3).^2.*sin(x_3).^2.*7.247222064e-3)+(x_9.^2.*cos(x_3).*cos(x_6).*sin(x_3).^2.*sin(x_6).*7.358998824951566e-12)./(cos(x_3).^4.*3.623611032e-3+sin(x_3).^4.*3.623611032e-3+cos(x_3).^2.*sin(x_3).^2.*7.247222064e-3)-(x_9.^2.*cos(x_3).^2.*cos(x_6).*sin(x_3).*sin(x_6).*7.358998824951566e-12)./(cos(x_3).^4.*3.623611032e-3+sin(x_3).^4.*3.623611032e-3+cos(x_3).^2.*sin(x_3).^2.*7.247222064e-3)+(th_ref.*cos(x_3).^2.*sin(x_3).^2.*sin(x_4).^2.*sin(x_5).^2.*4.839874983143591e-16)./(cos(x_3).^4.*3.628125e-2+sin(x_3).^4.*3.628125e-2+cos(x_3).^2.*sin(x_3).^2.*7.25625e-2)+(th_ref.*cos(x_3).^2.*sin(x_3).^2.*sin(x_4).^2.*sin(x_6).^2.*4.839874983143591e-16)./(cos(x_3).^4.*3.628125e-2+sin(x_3).^4.*3.628125e-2+cos(x_3).^2.*sin(x_3).^2.*7.25625e-2)+(th_ref.*cos(x_3).^2.*sin(x_3).^2.*sin(x_5).^2.*sin(x_6).^2.*4.839874983143591e-16)./(cos(x_3).^4.*3.628125e-2+sin(x_3).^4.*3.628125e-2+cos(x_3).^2.*sin(x_3).^2.*7.25625e-2)+(thp_ref.*cos(x_3).^2.*sin(x_3).^2.*sin(x_4).^2.*sin(x_5).^2.*4.839874983143591e-16)./(cos(x_3).^4.*3.628125e-2+sin(x_3).^4.*3.628125e-2+cos(x_3).^2.*sin(x_3).^2.*7.25625e-2)+(thp_ref.*cos(x_3).^2.*sin(x_3).^2.*sin(x_4).^2.*sin(x_6).^2.*4.839874983143591e-16)./(cos(x_3).^4.*3.628125e-2+sin(x_3).^4.*3.628125e-2+cos(x_3).^2.*sin(x_3).^2.*7.25625e-2)+(thp_ref.*cos(x_3).^2.*sin(x_3).^2.*sin(x_5).^2.*sin(x_6).^2.*4.839874983143591e-16)./(cos(x_3).^4.*3.628125e-2+sin(x_3).^4.*3.628125e-2+cos(x_3).^2.*sin(x_3).^2.*7.25625e-2)+(thpp_ref.*cos(x_3).^2.*sin(x_3).^2.*sin(x_4).^2.*sin(x_5).^2.*1.209968745785898e-16)./(cos(x_3).^4.*3.628125e-2+sin(x_3).^4.*3.628125e-2+cos(x_3).^2.*sin(x_3).^2.*7.25625e-2)+(thpp_ref.*cos(x_3).^2.*sin(x_3).^2.*sin(x_4).^2.*sin(x_6).^2.*1.209968745785898e-16)./(cos(x_3).^4.*3.628125e-2+sin(x_3).^4.*3.628125e-2+cos(x_3).^2.*sin(x_3).^2.*7.25625e-2)+(thpp_ref.*cos(x_3).^2.*sin(x_3).^2.*sin(x_5).^2.*sin(x_6).^2.*1.209968745785898e-16)./(cos(x_3).^4.*3.628125e-2+sin(x_3).^4.*3.628125e-2+cos(x_3).^2.*sin(x_3).^2.*7.25625e-2)-(x_3.*cos(x_3).^2.*sin(x_3).^2.*sin(x_4).^2.*sin(x_5).^2.*4.839874983143591e-16)./(cos(x_3).^4.*3.628125e-2+sin(x_3).^4.*3.628125e-2+cos(x_3).^2.*sin(x_3).^2.*7.25625e-2)-(x_3.*cos(x_3).^2.*sin(x_3).^2.*sin(x_4).^2.*sin(x_6).^2.*4.839874983143591e-16)./(cos(x_3).^4.*3.628125e-2+sin(x_3).^4.*3.628125e-2+cos(x_3).^2.*sin(x_3).^2.*7.25625e-2)-(x_3.*cos(x_3).^2.*sin(x_3).^2.*sin(x_5).^2.*sin(x_6).^2.*4.839874983143591e-16)./(cos(x_3).^4.*3.628125e-2+sin(x_3).^4.*3.628125e-2+cos(x_3).^2.*sin(x_3).^2.*7.25625e-2)-(x_9.*cos(x_3).^2.*sin(x_3).^2.*sin(x_4).^2.*sin(x_5).^2.*4.839874983143591e-16)./(cos(x_3).^4.*3.628125e-2+sin(x_3).^4.*3.628125e-2+cos(x_3).^2.*sin(x_3).^2.*7.25625e-2)-(x_9.*cos(x_3).^2.*sin(x_3).^2.*sin(x_4).^2.*sin(x_6).^2.*4.839874983143591e-16)./(cos(x_3).^4.*3.628125e-2+sin(x_3).^4.*3.628125e-2+cos(x_3).^2.*sin(x_3).^2.*7.25625e-2)-(x_9.*cos(x_3).^2.*sin(x_3).^2.*sin(x_5).^2.*sin(x_6).^2.*4.839874983143591e-16)./(cos(x_3).^4.*3.628125e-2+sin(x_3).^4.*3.628125e-2+cos(x_3).^2.*sin(x_3).^2.*7.25625e-2)-(x_9.^2.*sin(x_4.*2.0).*cos(x_3).*sin(x_3).^2.*sin(x_4).^2.*2.744511607628863e-19)./(cos(x_3).^4.*1.5163227196875e-5+sin(x_3).^4.*1.5163227196875e-5+cos(x_3).^4.*cos(x_4).^2.*2.702824874801215e-10+cos(x_3).^4.*cos(x_5).^2.*2.702824874801215e-10+cos(x_3).^4.*cos(x_6).^2.*2.702824874801215e-10+cos(x_3).^2.*sin(x_3).^2.*3.032645439375e-5+cos(x_4).^2.*sin(x_3).^4.*2.702824874801215e-10+cos(x_5).^2.*sin(x_3).^4.*2.702824874801215e-10+cos(x_6).^2.*sin(x_3).^4.*2.702824874801215e-10+cos(x_3).^2.*cos(x_4).^2.*sin(x_3).^2.*5.40564974960243e-10+cos(x_3).^2.*cos(x_5).^2.*sin(x_3).^2.*5.40564974960243e-10+cos(x_3).^2.*cos(x_6).^2.*sin(x_3).^2.*5.40564974960243e-10)+(x_9.^2.*sin(x_4.*2.0).*cos(x_3).^2.*sin(x_3).*sin(x_4).^2.*2.744511607628863e-19)./(cos(x_3).^4.*1.5163227196875e-5+sin(x_3).^4.*1.5163227196875e-5+cos(x_3).^4.*cos(x_4).^2.*2.702824874801215e-10+cos(x_3).^4.*cos(x_5).^2.*2.702824874801215e-10+cos(x_3).^4.*cos(x_6).^2.*2.702824874801215e-10+cos(x_3).^2.*sin(x_3).^2.*3.032645439375e-5+cos(x_4).^2.*sin(x_3).^4.*2.702824874801215e-10+cos(x_5).^2.*sin(x_3).^4.*2.702824874801215e-10+cos(x_6).^2.*sin(x_3).^4.*2.702824874801215e-10+cos(x_3).^2.*cos(x_4).^2.*sin(x_3).^2.*5.40564974960243e-10+cos(x_3).^2.*cos(x_5).^2.*sin(x_3).^2.*5.40564974960243e-10+cos(x_3).^2.*cos(x_6).^2.*sin(x_3).^2.*5.40564974960243e-10)-(x_9.^2.*sin(x_4.*2.0).*cos(x_3).*sin(x_3).^2.*sin(x_5).^2.*2.744511607628863e-19)./(cos(x_3).^4.*1.5163227196875e-5+sin(x_3).^4.*1.5163227196875e-5+cos(x_3).^4.*cos(x_4).^2.*2.702824874801215e-10+cos(x_3).^4.*cos(x_5).^2.*2.702824874801215e-10+cos(x_3).^4.*cos(x_6).^2.*2.702824874801215e-10+cos(x_3).^2.*sin(x_3).^2.*3.032645439375e-5+cos(x_4).^2.*sin(x_3).^4.*2.702824874801215e-10+cos(x_5).^2.*sin(x_3).^4.*2.702824874801215e-10+cos(x_6).^2.*sin(x_3).^4.*2.702824874801215e-10+cos(x_3).^2.*cos(x_4).^2.*sin(x_3).^2.*5.40564974960243e-10+cos(x_3).^2.*cos(x_5).^2.*sin(x_3).^2.*5.40564974960243e-10+cos(x_3).^2.*cos(x_6).^2.*sin(x_3).^2.*5.40564974960243e-10)+(x_9.^2.*sin(x_4.*2.0).*cos(x_3).^2.*sin(x_3).*sin(x_5).^2.*2.744511607628863e-19)./(cos(x_3).^4.*1.5163227196875e-5+sin(x_3).^4.*1.5163227196875e-5+cos(x_3).^4.*cos(x_4).^2.*2.702824874801215e-10+cos(x_3).^4.*cos(x_5).^2.*2.702824874801215e-10+cos(x_3).^4.*cos(x_6).^2.*2.702824874801215e-10+cos(x_3).^2.*sin(x_3).^2.*3.032645439375e-5+cos(x_4).^2.*sin(x_3).^4.*2.702824874801215e-10+cos(x_5).^2.*sin(x_3).^4.*2.702824874801215e-10+cos(x_6).^2.*sin(x_3).^4.*2.702824874801215e-10+cos(x_3).^2.*cos(x_4).^2.*sin(x_3).^2.*5.40564974960243e-10+cos(x_3).^2.*cos(x_5).^2.*sin(x_3).^2.*5.40564974960243e-10+cos(x_3).^2.*cos(x_6).^2.*sin(x_3).^2.*5.40564974960243e-10)-(x_9.^2.*sin(x_5.*2.0).*cos(x_3).*sin(x_3).^2.*sin(x_4).^2.*2.744511607628863e-19)./(cos(x_3).^4.*1.5163227196875e-5+sin(x_3).^4.*1.5163227196875e-5+cos(x_3).^4.*cos(x_4).^2.*2.702824874801215e-10+cos(x_3).^4.*cos(x_5).^2.*2.702824874801215e-10+cos(x_3).^4.*cos(x_6).^2.*2.702824874801215e-10+cos(x_3).^2.*sin(x_3).^2.*3.032645439375e-5+cos(x_4).^2.*sin(x_3).^4.*2.702824874801215e-10+cos(x_5).^2.*sin(x_3).^4.*2.702824874801215e-10+cos(x_6).^2.*sin(x_3).^4.*2.702824874801215e-10+cos(x_3).^2.*cos(x_4).^2.*sin(x_3).^2.*5.40564974960243e-10+cos(x_3).^2.*cos(x_5).^2.*sin(x_3).^2.*5.40564974960243e-10+cos(x_3).^2.*cos(x_6).^2.*sin(x_3).^2.*5.40564974960243e-10)+(x_9.^2.*sin(x_5.*2.0).*cos(x_3).^2.*sin(x_3).*sin(x_4).^2.*2.744511607628863e-19)./(cos(x_3).^4.*1.5163227196875e-5+sin(x_3).^4.*1.5163227196875e-5+cos(x_3).^4.*cos(x_4).^2.*2.702824874801215e-10+cos(x_3).^4.*cos(x_5).^2.*2.702824874801215e-10+cos(x_3).^4.*cos(x_6).^2.*2.702824874801215e-10+cos(x_3).^2.*sin(x_3).^2.*3.032645439375e-5+cos(x_4).^2.*sin(x_3).^4.*2.702824874801215e-10+cos(x_5).^2.*sin(x_3).^4.*2.702824874801215e-10+cos(x_6).^2.*sin(x_3).^4.*2.702824874801215e-10+cos(x_3).^2.*cos(x_4).^2.*sin(x_3).^2.*5.40564974960243e-10+cos(x_3).^2.*cos(x_5).^2.*sin(x_3).^2.*5.40564974960243e-10+cos(x_3).^2.*cos(x_6).^2.*sin(x_3).^2.*5.40564974960243e-10)-(x_9.^2.*sin(x_4.*2.0).*cos(x_3).*sin(x_3).^2.*sin(x_6).^2.*2.744511607628863e-19)./(cos(x_3).^4.*1.5163227196875e-5+sin(x_3).^4.*1.5163227196875e-5+cos(x_3).^4.*cos(x_4).^2.*2.702824874801215e-10+cos(x_3).^4.*cos(x_5).^2.*2.702824874801215e-10+cos(x_3).^4.*cos(x_6).^2.*2.702824874801215e-10+cos(x_3).^2.*sin(x_3).^2.*3.032645439375e-5+cos(x_4).^2.*sin(x_3).^4.*2.702824874801215e-10+cos(x_5).^2.*sin(x_3).^4.*2.702824874801215e-10+cos(x_6).^2.*sin(x_3).^4.*2.702824874801215e-10+cos(x_3).^2.*cos(x_4).^2.*sin(x_3).^2.*5.40564974960243e-10+cos(x_3).^2.*cos(x_5).^2.*sin(x_3).^2.*5.40564974960243e-10+cos(x_3).^2.*cos(x_6).^2.*sin(x_3).^2.*5.40564974960243e-10)+(x_9.^2.*sin(x_4.*2.0).*cos(x_3).^2.*sin(x_3).*sin(x_6).^2.*2.744511607628863e-19)./(cos(x_3).^4.*1.5163227196875e-5+sin(x_3).^4.*1.5163227196875e-5+cos(x_3).^4.*cos(x_4).^2.*2.702824874801215e-10+cos(x_3).^4.*cos(x_5).^2.*2.702824874801215e-10+cos(x_3).^4.*cos(x_6).^2.*2.702824874801215e-10+cos(x_3).^2.*sin(x_3).^2.*3.032645439375e-5+cos(x_4).^2.*sin(x_3).^4.*2.702824874801215e-10+cos(x_5).^2.*sin(x_3).^4.*2.702824874801215e-10+cos(x_6).^2.*sin(x_3).^4.*2.702824874801215e-10+cos(x_3).^2.*cos(x_4).^2.*sin(x_3).^2.*5.40564974960243e-10+cos(x_3).^2.*cos(x_5).^2.*sin(x_3).^2.*5.40564974960243e-10+cos(x_3).^2.*cos(x_6).^2.*sin(x_3).^2.*5.40564974960243e-10)-(x_9.^2.*sin(x_5.*2.0).*cos(x_3).*sin(x_3).^2.*sin(x_5).^2.*2.744511607628863e-19)./(cos(x_3).^4.*1.5163227196875e-5+sin(x_3).^4.*1.5163227196875e-5+cos(x_3).^4.*cos(x_4).^2.*2.702824874801215e-10+cos(x_3).^4.*cos(x_5).^2.*2.702824874801215e-10+cos(x_3).^4.*cos(x_6).^2.*2.702824874801215e-10+cos(x_3).^2.*sin(x_3).^2.*3.032645439375e-5+cos(x_4).^2.*sin(x_3).^4.*2.702824874801215e-10+cos(x_5).^2.*sin(x_3).^4.*2.702824874801215e-10+cos(x_6).^2.*sin(x_3).^4.*2.702824874801215e-10+cos(x_3).^2.*cos(x_4).^2.*sin(x_3).^2.*5.40564974960243e-10+cos(x_3).^2.*cos(x_5).^2.*sin(x_3).^2.*5.40564974960243e-10+cos(x_3).^2.*cos(x_6).^2.*sin(x_3).^2.*5.40564974960243e-10)+(x_9.^2.*sin(x_5.*2.0).*cos(x_3).^2.*sin(x_3).*sin(x_5).^2.*2.744511607628863e-19)./(cos(x_3).^4.*1.5163227196875e-5+sin(x_3).^4.*1.5163227196875e-5+cos(x_3).^4.*cos(x_4).^2.*2.702824874801215e-10+cos(x_3).^4.*cos(x_5).^2.*2.702824874801215e-10+cos(x_3).^4.*cos(x_6).^2.*2.702824874801215e-10+cos(x_3).^2.*sin(x_3).^2.*3.032645439375e-5+cos(x_4).^2.*sin(x_3).^4.*2.702824874801215e-10+cos(x_5).^2.*sin(x_3).^4.*2.702824874801215e-10+cos(x_6).^2.*sin(x_3).^4.*2.702824874801215e-10+cos(x_3).^2.*cos(x_4).^2.*sin(x_3).^2.*5.40564974960243e-10+cos(x_3).^2.*cos(x_5).^2.*sin(x_3).^2.*5.40564974960243e-10+cos(x_3).^2.*cos(x_6).^2.*sin(x_3).^2.*5.40564974960243e-10)-(x_9.^2.*sin(x_6.*2.0).*cos(x_3).*sin(x_3).^2.*sin(x_4).^2.*2.744511607628863e-19)./(cos(x_3).^4.*1.5163227196875e-5+sin(x_3).^4.*1.5163227196875e-5+cos(x_3).^4.*cos(x_4).^2.*2.702824874801215e-10+cos(x_3).^4.*cos(x_5).^2.*2.702824874801215e-10+cos(x_3).^4.*cos(x_6).^2.*2.702824874801215e-10+cos(x_3).^2.*sin(x_3).^2.*3.032645439375e-5+cos(x_4).^2.*sin(x_3).^4.*2.702824874801215e-10+cos(x_5).^2.*sin(x_3).^4.*2.702824874801215e-10+cos(x_6).^2.*sin(x_3).^4.*2.702824874801215e-10+cos(x_3).^2.*cos(x_4).^2.*sin(x_3).^2.*5.40564974960243e-10+cos(x_3).^2.*cos(x_5).^2.*sin(x_3).^2.*5.40564974960243e-10+cos(x_3).^2.*cos(x_6).^2.*sin(x_3).^2.*5.40564974960243e-10)+(x_9.^2.*sin(x_6.*2.0).*cos(x_3).^2.*sin(x_3).*sin(x_4).^2.*2.744511607628863e-19)./(cos(x_3).^4.*1.5163227196875e-5+sin(x_3).^4.*1.5163227196875e-5+cos(x_3).^4.*cos(x_4).^2.*2.702824874801215e-10+cos(x_3).^4.*cos(x_5).^2.*2.702824874801215e-10+cos(x_3).^4.*cos(x_6).^2.*2.702824874801215e-10+cos(x_3).^2.*sin(x_3).^2.*3.032645439375e-5+cos(x_4).^2.*sin(x_3).^4.*2.702824874801215e-10+cos(x_5).^2.*sin(x_3).^4.*2.702824874801215e-10+cos(x_6).^2.*sin(x_3).^4.*2.702824874801215e-10+cos(x_3).^2.*cos(x_4).^2.*sin(x_3).^2.*5.40564974960243e-10+cos(x_3).^2.*cos(x_5).^2.*sin(x_3).^2.*5.40564974960243e-10+cos(x_3).^2.*cos(x_6).^2.*sin(x_3).^2.*5.40564974960243e-10)-(x_9.^2.*sin(x_5.*2.0).*cos(x_3).*sin(x_3).^2.*sin(x_6).^2.*2.744511607628863e-19)./(cos(x_3).^4.*1.5163227196875e-5+sin(x_3).^4.*1.5163227196875e-5+cos(x_3).^4.*cos(x_4).^2.*2.702824874801215e-10+cos(x_3).^4.*cos(x_5).^2.*2.702824874801215e-10+cos(x_3).^4.*cos(x_6).^2.*2.702824874801215e-10+cos(x_3).^2.*sin(x_3).^2.*3.032645439375e-5+cos(x_4).^2.*sin(x_3).^4.*2.702824874801215e-10+cos(x_5).^2.*sin(x_3).^4.*2.702824874801215e-10+cos(x_6).^2.*sin(x_3).^4.*2.702824874801215e-10+cos(x_3).^2.*cos(x_4).^2.*sin(x_3).^2.*5.40564974960243e-10+cos(x_3).^2.*cos(x_5).^2.*sin(x_3).^2.*5.40564974960243e-10+cos(x_3).^2.*cos(x_6).^2.*sin(x_3).^2.*5.40564974960243e-10)+(x_9.^2.*sin(x_5.*2.0).*cos(x_3).^2.*sin(x_3).*sin(x_6).^2.*2.744511607628863e-19)./(cos(x_3).^4.*1.5163227196875e-5+sin(x_3).^4.*1.5163227196875e-5+cos(x_3).^4.*cos(x_4).^2.*2.702824874801215e-10+cos(x_3).^4.*cos(x_5).^2.*2.702824874801215e-10+cos(x_3).^4.*cos(x_6).^2.*2.702824874801215e-10+cos(x_3).^2.*sin(x_3).^2.*3.032645439375e-5+cos(x_4).^2.*sin(x_3).^4.*2.702824874801215e-10+cos(x_5).^2.*sin(x_3).^4.*2.702824874801215e-10+cos(x_6).^2.*sin(x_3).^4.*2.702824874801215e-10+cos(x_3).^2.*cos(x_4).^2.*sin(x_3).^2.*5.40564974960243e-10+cos(x_3).^2.*cos(x_5).^2.*sin(x_3).^2.*5.40564974960243e-10+cos(x_3).^2.*cos(x_6).^2.*sin(x_3).^2.*5.40564974960243e-10)-(x_9.^2.*sin(x_6.*2.0).*cos(x_3).*sin(x_3).^2.*sin(x_5).^2.*2.744511607628863e-19)./(cos(x_3).^4.*1.5163227196875e-5+sin(x_3).^4.*1.5163227196875e-5+cos(x_3).^4.*cos(x_4).^2.*2.702824874801215e-10+cos(x_3).^4.*cos(x_5).^2.*2.702824874801215e-10+cos(x_3).^4.*cos(x_6).^2.*2.702824874801215e-10+cos(x_3).^2.*sin(x_3).^2.*3.032645439375e-5+cos(x_4).^2.*sin(x_3).^4.*2.702824874801215e-10+cos(x_5).^2.*sin(x_3).^4.*2.702824874801215e-10+cos(x_6).^2.*sin(x_3).^4.*2.702824874801215e-10+cos(x_3).^2.*cos(x_4).^2.*sin(x_3).^2.*5.40564974960243e-10+cos(x_3).^2.*cos(x_5).^2.*sin(x_3).^2.*5.40564974960243e-10+cos(x_3).^2.*cos(x_6).^2.*sin(x_3).^2.*5.40564974960243e-10)+(x_9.^2.*sin(x_6.*2.0).*cos(x_3).^2.*sin(x_3).*sin(x_5).^2.*2.744511607628863e-19)./(cos(x_3).^4.*1.5163227196875e-5+sin(x_3).^4.*1.5163227196875e-5+cos(x_3).^4.*cos(x_4).^2.*2.702824874801215e-10+cos(x_3).^4.*cos(x_5).^2.*2.702824874801215e-10+cos(x_3).^4.*cos(x_6).^2.*2.702824874801215e-10+cos(x_3).^2.*sin(x_3).^2.*3.032645439375e-5+cos(x_4).^2.*sin(x_3).^4.*2.702824874801215e-10+cos(x_5).^2.*sin(x_3).^4.*2.702824874801215e-10+cos(x_6).^2.*sin(x_3).^4.*2.702824874801215e-10+cos(x_3).^2.*cos(x_4).^2.*sin(x_3).^2.*5.40564974960243e-10+cos(x_3).^2.*cos(x_5).^2.*sin(x_3).^2.*5.40564974960243e-10+cos(x_3).^2.*cos(x_6).^2.*sin(x_3).^2.*5.40564974960243e-10)-(x_9.^2.*sin(x_6.*2.0).*cos(x_3).*sin(x_3).^2.*sin(x_6).^2.*2.744511607628863e-19)./(cos(x_3).^4.*1.5163227196875e-5+sin(x_3).^4.*1.5163227196875e-5+cos(x_3).^4.*cos(x_4).^2.*2.702824874801215e-10+cos(x_3).^4.*cos(x_5).^2.*2.702824874801215e-10+cos(x_3).^4.*cos(x_6).^2.*2.702824874801215e-10+cos(x_3).^2.*sin(x_3).^2.*3.032645439375e-5+cos(x_4).^2.*sin(x_3).^4.*2.702824874801215e-10+cos(x_5).^2.*sin(x_3).^4.*2.702824874801215e-10+cos(x_6).^2.*sin(x_3).^4.*2.702824874801215e-10+cos(x_3).^2.*cos(x_4).^2.*sin(x_3).^2.*5.40564974960243e-10+cos(x_3).^2.*cos(x_5).^2.*sin(x_3).^2.*5.40564974960243e-10+cos(x_3).^2.*cos(x_6).^2.*sin(x_3).^2.*5.40564974960243e-10)+(x_9.^2.*sin(x_6.*2.0).*cos(x_3).^2.*sin(x_3).*sin(x_6).^2.*2.744511607628863e-19)./(cos(x_3).^4.*1.5163227196875e-5+sin(x_3).^4.*1.5163227196875e-5+cos(x_3).^4.*cos(x_4).^2.*2.702824874801215e-10+cos(x_3).^4.*cos(x_5).^2.*2.702824874801215e-10+cos(x_3).^4.*cos(x_6).^2.*2.702824874801215e-10+cos(x_3).^2.*sin(x_3).^2.*3.032645439375e-5+cos(x_4).^2.*sin(x_3).^4.*2.702824874801215e-10+cos(x_5).^2.*sin(x_3).^4.*2.702824874801215e-10+cos(x_6).^2.*sin(x_3).^4.*2.702824874801215e-10+cos(x_3).^2.*cos(x_4).^2.*sin(x_3).^2.*5.40564974960243e-10+cos(x_3).^2.*cos(x_5).^2.*sin(x_3).^2.*5.40564974960243e-10+cos(x_3).^2.*cos(x_6).^2.*sin(x_3).^2.*5.40564974960243e-10)+(x_9.^2.*cos(x_3).^2.*cos(x_4).*sin(x_3).^2.*sin(x_4).*2.46366703632003e-13)./(cos(x_3).^4.*9.05902758e-4+sin(x_3).^4.*9.05902758e-4+cos(x_3).^2.*sin(x_3).^2.*1.811805516e-3)+(x_9.^2.*cos(x_3).^2.*cos(x_5).*sin(x_3).^2.*sin(x_5).*2.46366703632003e-13)./(cos(x_3).^4.*9.05902758e-4+sin(x_3).^4.*9.05902758e-4+cos(x_3).^2.*sin(x_3).^2.*1.811805516e-3)-(x_9.^2.*cos(x_3).^2.*cos(x_6).*sin(x_3).^2.*sin(x_6).*4.92733407264006e-13)./(cos(x_3).^4.*9.05902758e-4+sin(x_3).^4.*9.05902758e-4+cos(x_3).^2.*sin(x_3).^2.*1.811805516e-3)-(x_9.^2.*cos(x_3).^4.*cos(x_4).*sin(x_4).*sin(x_5).^2.*2.19560928610309e-18)./(cos(x_3).^4.*9.05902758e-4+sin(x_3).^4.*9.05902758e-4+cos(x_3).^2.*sin(x_3).^2.*1.811805516e-3)-(x_9.^2.*cos(x_3).^4.*cos(x_4).*sin(x_4).*sin(x_6).^2.*2.19560928610309e-18)./(cos(x_3).^4.*9.05902758e-4+sin(x_3).^4.*9.05902758e-4+cos(x_3).^2.*sin(x_3).^2.*1.811805516e-3)-(x_9.^2.*cos(x_3).^4.*cos(x_5).*sin(x_4).^2.*sin(x_5).*2.19560928610309e-18)./(cos(x_3).^4.*9.05902758e-4+sin(x_3).^4.*9.05902758e-4+cos(x_3).^2.*sin(x_3).^2.*1.811805516e-3)-(x_9.^2.*cos(x_3).^4.*cos(x_5).*sin(x_5).*sin(x_6).^2.*2.19560928610309e-18)./(cos(x_3).^4.*9.05902758e-4+sin(x_3).^4.*9.05902758e-4+cos(x_3).^2.*sin(x_3).^2.*1.811805516e-3)+(x_9.^2.*cos(x_3).^4.*cos(x_6).*sin(x_4).^2.*sin(x_6).*4.39121857220618e-18)./(cos(x_3).^4.*9.05902758e-4+sin(x_3).^4.*9.05902758e-4+cos(x_3).^2.*sin(x_3).^2.*1.811805516e-3)+(x_9.^2.*cos(x_3).^4.*cos(x_6).*sin(x_5).^2.*sin(x_6).*4.39121857220618e-18)./(cos(x_3).^4.*9.05902758e-4+sin(x_3).^4.*9.05902758e-4+cos(x_3).^2.*sin(x_3).^2.*1.811805516e-3)-(x_9.^2.*cos(x_4).*sin(x_3).^4.*sin(x_4).*sin(x_5).^2.*2.19560928610309e-18)./(cos(x_3).^4.*9.05902758e-4+sin(x_3).^4.*9.05902758e-4+cos(x_3).^2.*sin(x_3).^2.*1.811805516e-3)-(x_9.^2.*cos(x_4).*sin(x_3).^4.*sin(x_4).*sin(x_6).^2.*2.19560928610309e-18)./(cos(x_3).^4.*9.05902758e-4+sin(x_3).^4.*9.05902758e-4+cos(x_3).^2.*sin(x_3).^2.*1.811805516e-3)-(x_9.^2.*cos(x_5).*sin(x_3).^4.*sin(x_4).^2.*sin(x_5).*2.19560928610309e-18)./(cos(x_3).^4.*9.05902758e-4+sin(x_3).^4.*9.05902758e-4+cos(x_3).^2.*sin(x_3).^2.*1.811805516e-3)-(x_9.^2.*cos(x_5).*sin(x_3).^4.*sin(x_5).*sin(x_6).^2.*2.19560928610309e-18)./(cos(x_3).^4.*9.05902758e-4+sin(x_3).^4.*9.05902758e-4+cos(x_3).^2.*sin(x_3).^2.*1.811805516e-3)+(x_9.^2.*cos(x_6).*sin(x_3).^4.*sin(x_4).^2.*sin(x_6).*4.39121857220618e-18)./(cos(x_3).^4.*9.05902758e-4+sin(x_3).^4.*9.05902758e-4+cos(x_3).^2.*sin(x_3).^2.*1.811805516e-3)+(x_9.^2.*cos(x_6).*sin(x_3).^4.*sin(x_5).^2.*sin(x_6).*4.39121857220618e-18)./(cos(x_3).^4.*9.05902758e-4+sin(x_3).^4.*9.05902758e-4+cos(x_3).^2.*sin(x_3).^2.*1.811805516e-3)+(x_8.*x_9.*cos(x_3).^5.*cos(x_4).*sin(x_4).*4.123968090108961e-15)./(cos(x_3).^4.*3.79080679921875e-6+sin(x_3).^4.*3.79080679921875e-6+cos(x_3).^4.*cos(x_4).^2.*6.757062187003037e-11+cos(x_3).^4.*cos(x_5).^2.*6.757062187003037e-11+cos(x_3).^4.*cos(x_6).^2.*6.757062187003037e-11+cos(x_3).^2.*sin(x_3).^2.*7.5816135984375e-6+cos(x_4).^2.*sin(x_3).^4.*6.757062187003037e-11+cos(x_5).^2.*sin(x_3).^4.*6.757062187003037e-11+cos(x_6).^2.*sin(x_3).^4.*6.757062187003037e-11+cos(x_3).^2.*cos(x_4).^2.*sin(x_3).^2.*1.351412437400607e-10+cos(x_3).^2.*cos(x_5).^2.*sin(x_3).^2.*1.351412437400607e-10+cos(x_3).^2.*cos(x_6).^2.*sin(x_3).^2.*1.351412437400607e-10)-(x_7.*x_9.*cos(x_3).^5.*cos(x_5).*sin(x_5).*3.571461130430754e-15)./(cos(x_3).^4.*3.79080679921875e-6+sin(x_3).^4.*3.79080679921875e-6+cos(x_3).^4.*cos(x_4).^2.*6.757062187003037e-11+cos(x_3).^4.*cos(x_5).^2.*6.757062187003037e-11+cos(x_3).^4.*cos(x_6).^2.*6.757062187003037e-11+cos(x_3).^2.*sin(x_3).^2.*7.5816135984375e-6+cos(x_4).^2.*sin(x_3).^4.*6.757062187003037e-11+cos(x_5).^2.*sin(x_3).^4.*6.757062187003037e-11+cos(x_6).^2.*sin(x_3).^4.*6.757062187003037e-11+cos(x_3).^2.*cos(x_4).^2.*sin(x_3).^2.*1.351412437400607e-10+cos(x_3).^2.*cos(x_5).^2.*sin(x_3).^2.*1.351412437400607e-10+cos(x_3).^2.*cos(x_6).^2.*sin(x_3).^2.*1.351412437400607e-10)-(x_8.*x_9.*cos(x_3).^5.*cos(x_5).*sin(x_5).*2.061984045054481e-15)./(cos(x_3).^4.*3.79080679921875e-6+sin(x_3).^4.*3.79080679921875e-6+cos(x_3).^4.*cos(x_4).^2.*6.757062187003037e-11+cos(x_3).^4.*cos(x_5).^2.*6.757062187003037e-11+cos(x_3).^4.*cos(x_6).^2.*6.757062187003037e-11+cos(x_3).^2.*sin(x_3).^2.*7.5816135984375e-6+cos(x_4).^2.*sin(x_3).^4.*6.757062187003037e-11+cos(x_5).^2.*sin(x_3).^4.*6.757062187003037e-11+cos(x_6).^2.*sin(x_3).^4.*6.757062187003037e-11+cos(x_3).^2.*cos(x_4).^2.*sin(x_3).^2.*1.351412437400607e-10+cos(x_3).^2.*cos(x_5).^2.*sin(x_3).^2.*1.351412437400607e-10+cos(x_3).^2.*cos(x_6).^2.*sin(x_3).^2.*1.351412437400607e-10)+(x_7.*x_9.*cos(x_3).^5.*cos(x_6).*sin(x_6).*3.571461130430754e-15)./(cos(x_3).^4.*3.79080679921875e-6+sin(x_3).^4.*3.79080679921875e-6+cos(x_3).^4.*cos(x_4).^2.*6.757062187003037e-11+cos(x_3).^4.*cos(x_5).^2.*6.757062187003037e-11+cos(x_3).^4.*cos(x_6).^2.*6.757062187003037e-11+cos(x_3).^2.*sin(x_3).^2.*7.5816135984375e-6+cos(x_4).^2.*sin(x_3).^4.*6.757062187003037e-11+cos(x_5).^2.*sin(x_3).^4.*6.757062187003037e-11+cos(x_6).^2.*sin(x_3).^4.*6.757062187003037e-11+cos(x_3).^2.*cos(x_4).^2.*sin(x_3).^2.*1.351412437400607e-10+cos(x_3).^2.*cos(x_5).^2.*sin(x_3).^2.*1.351412437400607e-10+cos(x_3).^2.*cos(x_6).^2.*sin(x_3).^2.*1.351412437400607e-10)-(x_8.*x_9.*cos(x_3).^5.*cos(x_6).*sin(x_6).*2.061984045054481e-15)./(cos(x_3).^4.*3.79080679921875e-6+sin(x_3).^4.*3.79080679921875e-6+cos(x_3).^4.*cos(x_4).^2.*6.757062187003037e-11+cos(x_3).^4.*cos(x_5).^2.*6.757062187003037e-11+cos(x_3).^4.*cos(x_6).^2.*6.757062187003037e-11+cos(x_3).^2.*sin(x_3).^2.*7.5816135984375e-6+cos(x_4).^2.*sin(x_3).^4.*6.757062187003037e-11+cos(x_5).^2.*sin(x_3).^4.*6.757062187003037e-11+cos(x_6).^2.*sin(x_3).^4.*6.757062187003037e-11+cos(x_3).^2.*cos(x_4).^2.*sin(x_3).^2.*1.351412437400607e-10+cos(x_3).^2.*cos(x_5).^2.*sin(x_3).^2.*1.351412437400607e-10+cos(x_3).^2.*cos(x_6).^2.*sin(x_3).^2.*1.351412437400607e-10)+(x_8.*x_9.*cos(x_3).^4.*cos(x_4).*sin(x_4).*2.46366703632003e-13)./(cos(x_3).^4.*1.5163227196875e-5+sin(x_3).^4.*1.5163227196875e-5+cos(x_3).^4.*cos(x_4).^2.*2.702824874801215e-10+cos(x_3).^4.*cos(x_5).^2.*2.702824874801215e-10+cos(x_3).^4.*cos(x_6).^2.*2.702824874801215e-10+cos(x_3).^2.*sin(x_3).^2.*3.032645439375e-5+cos(x_4).^2.*sin(x_3).^4.*2.702824874801215e-10+cos(x_5).^2.*sin(x_3).^4.*2.702824874801215e-10+cos(x_6).^2.*sin(x_3).^4.*2.702824874801215e-10+cos(x_3).^2.*cos(x_4).^2.*sin(x_3).^2.*5.40564974960243e-10+cos(x_3).^2.*cos(x_5).^2.*sin(x_3).^2.*5.40564974960243e-10+cos(x_3).^2.*cos(x_6).^2.*sin(x_3).^2.*5.40564974960243e-10)-(x_7.*x_9.*cos(x_3).^4.*cos(x_5).*sin(x_5).*2.133598239919465e-13)./(cos(x_3).^4.*1.5163227196875e-5+sin(x_3).^4.*1.5163227196875e-5+cos(x_3).^4.*cos(x_4).^2.*2.702824874801215e-10+cos(x_3).^4.*cos(x_5).^2.*2.702824874801215e-10+cos(x_3).^4.*cos(x_6).^2.*2.702824874801215e-10+cos(x_3).^2.*sin(x_3).^2.*3.032645439375e-5+cos(x_4).^2.*sin(x_3).^4.*2.702824874801215e-10+cos(x_5).^2.*sin(x_3).^4.*2.702824874801215e-10+cos(x_6).^2.*sin(x_3).^4.*2.702824874801215e-10+cos(x_3).^2.*cos(x_4).^2.*sin(x_3).^2.*5.40564974960243e-10+cos(x_3).^2.*cos(x_5).^2.*sin(x_3).^2.*5.40564974960243e-10+cos(x_3).^2.*cos(x_6).^2.*sin(x_3).^2.*5.40564974960243e-10)-(x_8.*x_9.*cos(x_3).^4.*cos(x_5).*sin(x_5).*1.231833518160015e-13)./(cos(x_3).^4.*1.5163227196875e-5+sin(x_3).^4.*1.5163227196875e-5+cos(x_3).^4.*cos(x_4).^2.*2.702824874801215e-10+cos(x_3).^4.*cos(x_5).^2.*2.702824874801215e-10+cos(x_3).^4.*cos(x_6).^2.*2.702824874801215e-10+cos(x_3).^2.*sin(x_3).^2.*3.032645439375e-5+cos(x_4).^2.*sin(x_3).^4.*2.702824874801215e-10+cos(x_5).^2.*sin(x_3).^4.*2.702824874801215e-10+cos(x_6).^2.*sin(x_3).^4.*2.702824874801215e-10+cos(x_3).^2.*cos(x_4).^2.*sin(x_3).^2.*5.40564974960243e-10+cos(x_3).^2.*cos(x_5).^2.*sin(x_3).^2.*5.40564974960243e-10+cos(x_3).^2.*cos(x_6).^2.*sin(x_3).^2.*5.40564974960243e-10)+(x_7.*x_9.*cos(x_3).^4.*cos(x_6).*sin(x_6).*2.133598239919465e-13)./(cos(x_3).^4.*1.5163227196875e-5+sin(x_3).^4.*1.5163227196875e-5+cos(x_3).^4.*cos(x_4).^2.*2.702824874801215e-10+cos(x_3).^4.*cos(x_5).^2.*2.702824874801215e-10+cos(x_3).^4.*cos(x_6).^2.*2.702824874801215e-10+cos(x_3).^2.*sin(x_3).^2.*3.032645439375e-5+cos(x_4).^2.*sin(x_3).^4.*2.702824874801215e-10+cos(x_5).^2.*sin(x_3).^4.*2.702824874801215e-10+cos(x_6).^2.*sin(x_3).^4.*2.702824874801215e-10+cos(x_3).^2.*cos(x_4).^2.*sin(x_3).^2.*5.40564974960243e-10+cos(x_3).^2.*cos(x_5).^2.*sin(x_3).^2.*5.40564974960243e-10+cos(x_3).^2.*cos(x_6).^2.*sin(x_3).^2.*5.40564974960243e-10)-(x_8.*x_9.*cos(x_3).^4.*cos(x_6).*sin(x_6).*1.231833518160015e-13)./(cos(x_3).^4.*1.5163227196875e-5+sin(x_3).^4.*1.5163227196875e-5+cos(x_3).^4.*cos(x_4).^2.*2.702824874801215e-10+cos(x_3).^4.*cos(x_5).^2.*2.702824874801215e-10+cos(x_3).^4.*cos(x_6).^2.*2.702824874801215e-10+cos(x_3).^2.*sin(x_3).^2.*3.032645439375e-5+cos(x_4).^2.*sin(x_3).^4.*2.702824874801215e-10+cos(x_5).^2.*sin(x_3).^4.*2.702824874801215e-10+cos(x_6).^2.*sin(x_3).^4.*2.702824874801215e-10+cos(x_3).^2.*cos(x_4).^2.*sin(x_3).^2.*5.40564974960243e-10+cos(x_3).^2.*cos(x_5).^2.*sin(x_3).^2.*5.40564974960243e-10+cos(x_3).^2.*cos(x_6).^2.*sin(x_3).^2.*5.40564974960243e-10)+(x_9.^2.*cos(x_3).^2.*sin(x_3).^2.*sin(x_4).^2.*sin(x_5).^2.*7.601921214217226e-61)./(cos(x_3).^4.*3.79080679921875e-6+sin(x_3).^4.*3.79080679921875e-6+cos(x_3).^4.*cos(x_4).^2.*6.757062187003037e-11+cos(x_3).^4.*cos(x_5).^2.*6.757062187003037e-11+cos(x_3).^4.*cos(x_6).^2.*6.757062187003037e-11+cos(x_3).^2.*sin(x_3).^2.*7.5816135984375e-6+cos(x_4).^2.*sin(x_3).^4.*6.757062187003037e-11+cos(x_5).^2.*sin(x_3).^4.*6.757062187003037e-11+cos(x_6).^2.*sin(x_3).^4.*6.757062187003037e-11+cos(x_3).^2.*cos(x_4).^2.*sin(x_3).^2.*1.351412437400607e-10+cos(x_3).^2.*cos(x_5).^2.*sin(x_3).^2.*1.351412437400607e-10+cos(x_3).^2.*cos(x_6).^2.*sin(x_3).^2.*1.351412437400607e-10)+(x_9.^2.*cos(x_3).^2.*sin(x_3).^2.*sin(x_4).^2.*sin(x_6).^2.*7.601921214217226e-61)./(cos(x_3).^4.*3.79080679921875e-6+sin(x_3).^4.*3.79080679921875e-6+cos(x_3).^4.*cos(x_4).^2.*6.757062187003037e-11+cos(x_3).^4.*cos(x_5).^2.*6.757062187003037e-11+cos(x_3).^4.*cos(x_6).^2.*6.757062187003037e-11+cos(x_3).^2.*sin(x_3).^2.*7.5816135984375e-6+cos(x_4).^2.*sin(x_3).^4.*6.757062187003037e-11+cos(x_5).^2.*sin(x_3).^4.*6.757062187003037e-11+cos(x_6).^2.*sin(x_3).^4.*6.757062187003037e-11+cos(x_3).^2.*cos(x_4).^2.*sin(x_3).^2.*1.351412437400607e-10+cos(x_3).^2.*cos(x_5).^2.*sin(x_3).^2.*1.351412437400607e-10+cos(x_3).^2.*cos(x_6).^2.*sin(x_3).^2.*1.351412437400607e-10)+(x_9.^2.*cos(x_3).^2.*sin(x_3).^2.*sin(x_5).^2.*sin(x_6).^2.*7.601921214217226e-61)./(cos(x_3).^4.*3.79080679921875e-6+sin(x_3).^4.*3.79080679921875e-6+cos(x_3).^4.*cos(x_4).^2.*6.757062187003037e-11+cos(x_3).^4.*cos(x_5).^2.*6.757062187003037e-11+cos(x_3).^4.*cos(x_6).^2.*6.757062187003037e-11+cos(x_3).^2.*sin(x_3).^2.*7.5816135984375e-6+cos(x_4).^2.*sin(x_3).^4.*6.757062187003037e-11+cos(x_5).^2.*sin(x_3).^4.*6.757062187003037e-11+cos(x_6).^2.*sin(x_3).^4.*6.757062187003037e-11+cos(x_3).^2.*cos(x_4).^2.*sin(x_3).^2.*1.351412437400607e-10+cos(x_3).^2.*cos(x_5).^2.*sin(x_3).^2.*1.351412437400607e-10+cos(x_3).^2.*cos(x_6).^2.*sin(x_3).^2.*1.351412437400607e-10)-(x_8.*x_9.*cos(x_3).^3.*cos(x_4).*sin(x_4).*4.361535375749998e-7)./(cos(x_3).^2.*6.49519052838329e-1+sin(x_3).^2.*6.49519052838329e-1)+(x_7.*x_9.*cos(x_3).^3.*cos(x_5).*sin(x_5).*3.777200434904005e-7)./(cos(x_3).^2.*6.49519052838329e-1+sin(x_3).^2.*6.49519052838329e-1)+(x_8.*x_9.*cos(x_3).^3.*cos(x_5).*sin(x_5).*2.180767687874999e-7)./(cos(x_3).^2.*6.49519052838329e-1+sin(x_3).^2.*6.49519052838329e-1)-(x_7.*x_9.*cos(x_3).^3.*cos(x_6).*sin(x_6).*3.777200434904005e-7)./(cos(x_3).^2.*6.49519052838329e-1+sin(x_3).^2.*6.49519052838329e-1)+(x_8.*x_9.*cos(x_3).^3.*cos(x_6).*sin(x_6).*2.180767687874999e-7)./(cos(x_3).^2.*6.49519052838329e-1+sin(x_3).^2.*6.49519052838329e-1)-(x_7.*x_9.*cos(x_4).*sin(x_3).^5.*sin(x_4).*4.123968090108961e-15)./(cos(x_3).^4.*3.79080679921875e-6+sin(x_3).^4.*3.79080679921875e-6+cos(x_3).^4.*cos(x_4).^2.*6.757062187003037e-11+cos(x_3).^4.*cos(x_5).^2.*6.757062187003037e-11+cos(x_3).^4.*cos(x_6).^2.*6.757062187003037e-11+cos(x_3).^2.*sin(x_3).^2.*7.5816135984375e-6+cos(x_4).^2.*sin(x_3).^4.*6.757062187003037e-11+cos(x_5).^2.*sin(x_3).^4.*6.757062187003037e-11+cos(x_6).^2.*sin(x_3).^4.*6.757062187003037e-11+cos(x_3).^2.*cos(x_4).^2.*sin(x_3).^2.*1.351412437400607e-10+cos(x_3).^2.*cos(x_5).^2.*sin(x_3).^2.*1.351412437400607e-10+cos(x_3).^2.*cos(x_6).^2.*sin(x_3).^2.*1.351412437400607e-10)+(x_7.*x_9.*cos(x_5).*sin(x_3).^5.*sin(x_5).*2.061984045054481e-15)./(cos(x_3).^4.*3.79080679921875e-6+sin(x_3).^4.*3.79080679921875e-6+cos(x_3).^4.*cos(x_4).^2.*6.757062187003037e-11+cos(x_3).^4.*cos(x_5).^2.*6.757062187003037e-11+cos(x_3).^4.*cos(x_6).^2.*6.757062187003037e-11+cos(x_3).^2.*sin(x_3).^2.*7.5816135984375e-6+cos(x_4).^2.*sin(x_3).^4.*6.757062187003037e-11+cos(x_5).^2.*sin(x_3).^4.*6.757062187003037e-11+cos(x_6).^2.*sin(x_3).^4.*6.757062187003037e-11+cos(x_3).^2.*cos(x_4).^2.*sin(x_3).^2.*1.351412437400607e-10+cos(x_3).^2.*cos(x_5).^2.*sin(x_3).^2.*1.351412437400607e-10+cos(x_3).^2.*cos(x_6).^2.*sin(x_3).^2.*1.351412437400607e-10)-(x_8.*x_9.*cos(x_5).*sin(x_3).^5.*sin(x_5).*3.571461130430754e-15)./(cos(x_3).^4.*3.79080679921875e-6+sin(x_3).^4.*3.79080679921875e-6+cos(x_3).^4.*cos(x_4).^2.*6.757062187003037e-11+cos(x_3).^4.*cos(x_5).^2.*6.757062187003037e-11+cos(x_3).^4.*cos(x_6).^2.*6.757062187003037e-11+cos(x_3).^2.*sin(x_3).^2.*7.5816135984375e-6+cos(x_4).^2.*sin(x_3).^4.*6.757062187003037e-11+cos(x_5).^2.*sin(x_3).^4.*6.757062187003037e-11+cos(x_6).^2.*sin(x_3).^4.*6.757062187003037e-11+cos(x_3).^2.*cos(x_4).^2.*sin(x_3).^2.*1.351412437400607e-10+cos(x_3).^2.*cos(x_5).^2.*sin(x_3).^2.*1.351412437400607e-10+cos(x_3).^2.*cos(x_6).^2.*sin(x_3).^2.*1.351412437400607e-10)+(x_7.*x_9.*cos(x_6).*sin(x_3).^5.*sin(x_6).*2.061984045054481e-15)./(cos(x_3).^4.*3.79080679921875e-6+sin(x_3).^4.*3.79080679921875e-6+cos(x_3).^4.*cos(x_4).^2.*6.757062187003037e-11+cos(x_3).^4.*cos(x_5).^2.*6.757062187003037e-11+cos(x_3).^4.*cos(x_6).^2.*6.757062187003037e-11+cos(x_3).^2.*sin(x_3).^2.*7.5816135984375e-6+cos(x_4).^2.*sin(x_3).^4.*6.757062187003037e-11+cos(x_5).^2.*sin(x_3).^4.*6.757062187003037e-11+cos(x_6).^2.*sin(x_3).^4.*6.757062187003037e-11+cos(x_3).^2.*cos(x_4).^2.*sin(x_3).^2.*1.351412437400607e-10+cos(x_3).^2.*cos(x_5).^2.*sin(x_3).^2.*1.351412437400607e-10+cos(x_3).^2.*cos(x_6).^2.*sin(x_3).^2.*1.351412437400607e-10)+(x_8.*x_9.*cos(x_6).*sin(x_3).^5.*sin(x_6).*3.571461130430754e-15)./(cos(x_3).^4.*3.79080679921875e-6+sin(x_3).^4.*3.79080679921875e-6+cos(x_3).^4.*cos(x_4).^2.*6.757062187003037e-11+cos(x_3).^4.*cos(x_5).^2.*6.757062187003037e-11+cos(x_3).^4.*cos(x_6).^2.*6.757062187003037e-11+cos(x_3).^2.*sin(x_3).^2.*7.5816135984375e-6+cos(x_4).^2.*sin(x_3).^4.*6.757062187003037e-11+cos(x_5).^2.*sin(x_3).^4.*6.757062187003037e-11+cos(x_6).^2.*sin(x_3).^4.*6.757062187003037e-11+cos(x_3).^2.*cos(x_4).^2.*sin(x_3).^2.*1.351412437400607e-10+cos(x_3).^2.*cos(x_5).^2.*sin(x_3).^2.*1.351412437400607e-10+cos(x_3).^2.*cos(x_6).^2.*sin(x_3).^2.*1.351412437400607e-10)+(x_7.*x_9.*cos(x_4).*sin(x_3).^4.*sin(x_4).*2.46366703632003e-13)./(cos(x_3).^4.*1.5163227196875e-5+sin(x_3).^4.*1.5163227196875e-5+cos(x_3).^4.*cos(x_4).^2.*2.702824874801215e-10+cos(x_3).^4.*cos(x_5).^2.*2.702824874801215e-10+cos(x_3).^4.*cos(x_6).^2.*2.702824874801215e-10+cos(x_3).^2.*sin(x_3).^2.*3.032645439375e-5+cos(x_4).^2.*sin(x_3).^4.*2.702824874801215e-10+cos(x_5).^2.*sin(x_3).^4.*2.702824874801215e-10+cos(x_6).^2.*sin(x_3).^4.*2.702824874801215e-10+cos(x_3).^2.*cos(x_4).^2.*sin(x_3).^2.*5.40564974960243e-10+cos(x_3).^2.*cos(x_5).^2.*sin(x_3).^2.*5.40564974960243e-10+cos(x_3).^2.*cos(x_6).^2.*sin(x_3).^2.*5.40564974960243e-10)-(x_7.*x_9.*cos(x_5).*sin(x_3).^4.*sin(x_5).*1.231833518160015e-13)./(cos(x_3).^4.*1.5163227196875e-5+sin(x_3).^4.*1.5163227196875e-5+cos(x_3).^4.*cos(x_4).^2.*2.702824874801215e-10+cos(x_3).^4.*cos(x_5).^2.*2.702824874801215e-10+cos(x_3).^4.*cos(x_6).^2.*2.702824874801215e-10+cos(x_3).^2.*sin(x_3).^2.*3.032645439375e-5+cos(x_4).^2.*sin(x_3).^4.*2.702824874801215e-10+cos(x_5).^2.*sin(x_3).^4.*2.702824874801215e-10+cos(x_6).^2.*sin(x_3).^4.*2.702824874801215e-10+cos(x_3).^2.*cos(x_4).^2.*sin(x_3).^2.*5.40564974960243e-10+cos(x_3).^2.*cos(x_5).^2.*sin(x_3).^2.*5.40564974960243e-10+cos(x_3).^2.*cos(x_6).^2.*sin(x_3).^2.*5.40564974960243e-10)+(x_8.*x_9.*cos(x_5).*sin(x_3).^4.*sin(x_5).*2.133598239919465e-13)./(cos(x_3).^4.*1.5163227196875e-5+sin(x_3).^4.*1.5163227196875e-5+cos(x_3).^4.*cos(x_4).^2.*2.702824874801215e-10+cos(x_3).^4.*cos(x_5).^2.*2.702824874801215e-10+cos(x_3).^4.*cos(x_6).^2.*2.702824874801215e-10+cos(x_3).^2.*sin(x_3).^2.*3.032645439375e-5+cos(x_4).^2.*sin(x_3).^4.*2.702824874801215e-10+cos(x_5).^2.*sin(x_3).^4.*2.702824874801215e-10+cos(x_6).^2.*sin(x_3).^4.*2.702824874801215e-10+cos(x_3).^2.*cos(x_4).^2.*sin(x_3).^2.*5.40564974960243e-10+cos(x_3).^2.*cos(x_5).^2.*sin(x_3).^2.*5.40564974960243e-10+cos(x_3).^2.*cos(x_6).^2.*sin(x_3).^2.*5.40564974960243e-10)-(x_7.*x_9.*cos(x_6).*sin(x_3).^4.*sin(x_6).*1.231833518160015e-13)./(cos(x_3).^4.*1.5163227196875e-5+sin(x_3).^4.*1.5163227196875e-5+cos(x_3).^4.*cos(x_4).^2.*2.702824874801215e-10+cos(x_3).^4.*cos(x_5).^2.*2.702824874801215e-10+cos(x_3).^4.*cos(x_6).^2.*2.702824874801215e-10+cos(x_3).^2.*sin(x_3).^2.*3.032645439375e-5+cos(x_4).^2.*sin(x_3).^4.*2.702824874801215e-10+cos(x_5).^2.*sin(x_3).^4.*2.702824874801215e-10+cos(x_6).^2.*sin(x_3).^4.*2.702824874801215e-10+cos(x_3).^2.*cos(x_4).^2.*sin(x_3).^2.*5.40564974960243e-10+cos(x_3).^2.*cos(x_5).^2.*sin(x_3).^2.*5.40564974960243e-10+cos(x_3).^2.*cos(x_6).^2.*sin(x_3).^2.*5.40564974960243e-10)-(x_8.*x_9.*cos(x_6).*sin(x_3).^4.*sin(x_6).*2.133598239919465e-13)./(cos(x_3).^4.*1.5163227196875e-5+sin(x_3).^4.*1.5163227196875e-5+cos(x_3).^4.*cos(x_4).^2.*2.702824874801215e-10+cos(x_3).^4.*cos(x_5).^2.*2.702824874801215e-10+cos(x_3).^4.*cos(x_6).^2.*2.702824874801215e-10+cos(x_3).^2.*sin(x_3).^2.*3.032645439375e-5+cos(x_4).^2.*sin(x_3).^4.*2.702824874801215e-10+cos(x_5).^2.*sin(x_3).^4.*2.702824874801215e-10+cos(x_6).^2.*sin(x_3).^4.*2.702824874801215e-10+cos(x_3).^2.*cos(x_4).^2.*sin(x_3).^2.*5.40564974960243e-10+cos(x_3).^2.*cos(x_5).^2.*sin(x_3).^2.*5.40564974960243e-10+cos(x_3).^2.*cos(x_6).^2.*sin(x_3).^2.*5.40564974960243e-10)-(x_9.^2.*cos(x_3).^2.*cos(x_4).*sin(x_3).^2.*sin(x_4).*sin(x_5).^2.*4.39121857220618e-18)./(cos(x_3).^4.*9.05902758e-4+sin(x_3).^4.*9.05902758e-4+cos(x_3).^2.*sin(x_3).^2.*1.811805516e-3)-(x_9.^2.*cos(x_3).^2.*cos(x_4).*sin(x_3).^2.*sin(x_4).*sin(x_6).^2.*4.39121857220618e-18)./(cos(x_3).^4.*9.05902758e-4+sin(x_3).^4.*9.05902758e-4+cos(x_3).^2.*sin(x_3).^2.*1.811805516e-3)-(x_9.^2.*cos(x_3).^2.*cos(x_5).*sin(x_3).^2.*sin(x_4).^2.*sin(x_5).*4.39121857220618e-18)./(cos(x_3).^4.*9.05902758e-4+sin(x_3).^4.*9.05902758e-4+cos(x_3).^2.*sin(x_3).^2.*1.811805516e-3)-(x_9.^2.*cos(x_3).^2.*cos(x_5).*sin(x_3).^2.*sin(x_5).*sin(x_6).^2.*4.39121857220618e-18)./(cos(x_3).^4.*9.05902758e-4+sin(x_3).^4.*9.05902758e-4+cos(x_3).^2.*sin(x_3).^2.*1.811805516e-3)+(x_9.^2.*cos(x_3).^2.*cos(x_6).*sin(x_3).^2.*sin(x_4).^2.*sin(x_6).*8.782437144412361e-18)./(cos(x_3).^4.*9.05902758e-4+sin(x_3).^4.*9.05902758e-4+cos(x_3).^2.*sin(x_3).^2.*1.811805516e-3)+(x_9.^2.*cos(x_3).^2.*cos(x_6).*sin(x_3).^2.*sin(x_5).^2.*sin(x_6).*8.782437144412361e-18)./(cos(x_3).^4.*9.05902758e-4+sin(x_3).^4.*9.05902758e-4+cos(x_3).^2.*sin(x_3).^2.*1.811805516e-3)-(x_7.*x_9.*cos(x_3).^2.*cos(x_4).*sin(x_3).^3.*sin(x_4).*8.247936180217923e-15)./(cos(x_3).^4.*3.79080679921875e-6+sin(x_3).^4.*3.79080679921875e-6+cos(x_3).^4.*cos(x_4).^2.*6.757062187003037e-11+cos(x_3).^4.*cos(x_5).^2.*6.757062187003037e-11+cos(x_3).^4.*cos(x_6).^2.*6.757062187003037e-11+cos(x_3).^2.*sin(x_3).^2.*7.5816135984375e-6+cos(x_4).^2.*sin(x_3).^4.*6.757062187003037e-11+cos(x_5).^2.*sin(x_3).^4.*6.757062187003037e-11+cos(x_6).^2.*sin(x_3).^4.*6.757062187003037e-11+cos(x_3).^2.*cos(x_4).^2.*sin(x_3).^2.*1.351412437400607e-10+cos(x_3).^2.*cos(x_5).^2.*sin(x_3).^2.*1.351412437400607e-10+cos(x_3).^2.*cos(x_6).^2.*sin(x_3).^2.*1.351412437400607e-10)+(x_8.*x_9.*cos(x_3).^3.*cos(x_4).*sin(x_3).^2.*sin(x_4).*8.247936180217923e-15)./(cos(x_3).^4.*3.79080679921875e-6+sin(x_3).^4.*3.79080679921875e-6+cos(x_3).^4.*cos(x_4).^2.*6.757062187003037e-11+cos(x_3).^4.*cos(x_5).^2.*6.757062187003037e-11+cos(x_3).^4.*cos(x_6).^2.*6.757062187003037e-11+cos(x_3).^2.*sin(x_3).^2.*7.5816135984375e-6+cos(x_4).^2.*sin(x_3).^4.*6.757062187003037e-11+cos(x_5).^2.*sin(x_3).^4.*6.757062187003037e-11+cos(x_6).^2.*sin(x_3).^4.*6.757062187003037e-11+cos(x_3).^2.*cos(x_4).^2.*sin(x_3).^2.*1.351412437400607e-10+cos(x_3).^2.*cos(x_5).^2.*sin(x_3).^2.*1.351412437400607e-10+cos(x_3).^2.*cos(x_6).^2.*sin(x_3).^2.*1.351412437400607e-10)+(x_7.*x_9.*cos(x_3).^2.*cos(x_5).*sin(x_3).^3.*sin(x_5).*4.123968090108961e-15)./(cos(x_3).^4.*3.79080679921875e-6+sin(x_3).^4.*3.79080679921875e-6+cos(x_3).^4.*cos(x_4).^2.*6.757062187003037e-11+cos(x_3).^4.*cos(x_5).^2.*6.757062187003037e-11+cos(x_3).^4.*cos(x_6).^2.*6.757062187003037e-11+cos(x_3).^2.*sin(x_3).^2.*7.5816135984375e-6+cos(x_4).^2.*sin(x_3).^4.*6.757062187003037e-11+cos(x_5).^2.*sin(x_3).^4.*6.757062187003037e-11+cos(x_6).^2.*sin(x_3).^4.*6.757062187003037e-11+cos(x_3).^2.*cos(x_4).^2.*sin(x_3).^2.*1.351412437400607e-10+cos(x_3).^2.*cos(x_5).^2.*sin(x_3).^2.*1.351412437400607e-10+cos(x_3).^2.*cos(x_6).^2.*sin(x_3).^2.*1.351412437400607e-10)-(x_7.*x_9.*cos(x_3).^3.*cos(x_5).*sin(x_3).^2.*sin(x_5).*7.142922260861507e-15)./(cos(x_3).^4.*3.79080679921875e-6+sin(x_3).^4.*3.79080679921875e-6+cos(x_3).^4.*cos(x_4).^2.*6.757062187003037e-11+cos(x_3).^4.*cos(x_5).^2.*6.757062187003037e-11+cos(x_3).^4.*cos(x_6).^2.*6.757062187003037e-11+cos(x_3).^2.*sin(x_3).^2.*7.5816135984375e-6+cos(x_4).^2.*sin(x_3).^4.*6.757062187003037e-11+cos(x_5).^2.*sin(x_3).^4.*6.757062187003037e-11+cos(x_6).^2.*sin(x_3).^4.*6.757062187003037e-11+cos(x_3).^2.*cos(x_4).^2.*sin(x_3).^2.*1.351412437400607e-10+cos(x_3).^2.*cos(x_5).^2.*sin(x_3).^2.*1.351412437400607e-10+cos(x_3).^2.*cos(x_6).^2.*sin(x_3).^2.*1.351412437400607e-10)+(x_7.*x_9.*cos(x_3).^4.*cos(x_4).*sin(x_3).*sin(x_4).^3.*1.470104929075305e-19)./(cos(x_3).^4.*3.79080679921875e-6+sin(x_3).^4.*3.79080679921875e-6+cos(x_3).^4.*cos(x_4).^2.*6.757062187003037e-11+cos(x_3).^4.*cos(x_5).^2.*6.757062187003037e-11+cos(x_3).^4.*cos(x_6).^2.*6.757062187003037e-11+cos(x_3).^2.*sin(x_3).^2.*7.5816135984375e-6+cos(x_4).^2.*sin(x_3).^4.*6.757062187003037e-11+cos(x_5).^2.*sin(x_3).^4.*6.757062187003037e-11+cos(x_6).^2.*sin(x_3).^4.*6.757062187003037e-11+cos(x_3).^2.*cos(x_4).^2.*sin(x_3).^2.*1.351412437400607e-10+cos(x_3).^2.*cos(x_5).^2.*sin(x_3).^2.*1.351412437400607e-10+cos(x_3).^2.*cos(x_6).^2.*sin(x_3).^2.*1.351412437400607e-10)-(x_8.*x_9.*cos(x_3).*cos(x_4).*sin(x_3).^4.*sin(x_4).^3.*1.470104929075305e-19)./(cos(x_3).^4.*3.79080679921875e-6+sin(x_3).^4.*3.79080679921875e-6+cos(x_3).^4.*cos(x_4).^2.*6.757062187003037e-11+cos(x_3).^4.*cos(x_5).^2.*6.757062187003037e-11+cos(x_3).^4.*cos(x_6).^2.*6.757062187003037e-11+cos(x_3).^2.*sin(x_3).^2.*7.5816135984375e-6+cos(x_4).^2.*sin(x_3).^4.*6.757062187003037e-11+cos(x_5).^2.*sin(x_3).^4.*6.757062187003037e-11+cos(x_6).^2.*sin(x_3).^4.*6.757062187003037e-11+cos(x_3).^2.*cos(x_4).^2.*sin(x_3).^2.*1.351412437400607e-10+cos(x_3).^2.*cos(x_5).^2.*sin(x_3).^2.*1.351412437400607e-10+cos(x_3).^2.*cos(x_6).^2.*sin(x_3).^2.*1.351412437400607e-10)-(x_8.*x_9.*cos(x_3).^2.*cos(x_5).*sin(x_3).^3.*sin(x_5).*7.142922260861507e-15)./(cos(x_3).^4.*3.79080679921875e-6+sin(x_3).^4.*3.79080679921875e-6+cos(x_3).^4.*cos(x_4).^2.*6.757062187003037e-11+cos(x_3).^4.*cos(x_5).^2.*6.757062187003037e-11+cos(x_3).^4.*cos(x_6).^2.*6.757062187003037e-11+cos(x_3).^2.*sin(x_3).^2.*7.5816135984375e-6+cos(x_4).^2.*sin(x_3).^4.*6.757062187003037e-11+cos(x_5).^2.*sin(x_3).^4.*6.757062187003037e-11+cos(x_6).^2.*sin(x_3).^4.*6.757062187003037e-11+cos(x_3).^2.*cos(x_4).^2.*sin(x_3).^2.*1.351412437400607e-10+cos(x_3).^2.*cos(x_5).^2.*sin(x_3).^2.*1.351412437400607e-10+cos(x_3).^2.*cos(x_6).^2.*sin(x_3).^2.*1.351412437400607e-10)-(x_8.*x_9.*cos(x_3).^3.*cos(x_5).*sin(x_3).^2.*sin(x_5).*4.123968090108961e-15)./(cos(x_3).^4.*3.79080679921875e-6+sin(x_3).^4.*3.79080679921875e-6+cos(x_3).^4.*cos(x_4).^2.*6.757062187003037e-11+cos(x_3).^4.*cos(x_5).^2.*6.757062187003037e-11+cos(x_3).^4.*cos(x_6).^2.*6.757062187003037e-11+cos(x_3).^2.*sin(x_3).^2.*7.5816135984375e-6+cos(x_4).^2.*sin(x_3).^4.*6.757062187003037e-11+cos(x_5).^2.*sin(x_3).^4.*6.757062187003037e-11+cos(x_6).^2.*sin(x_3).^4.*6.757062187003037e-11+cos(x_3).^2.*cos(x_4).^2.*sin(x_3).^2.*1.351412437400607e-10+cos(x_3).^2.*cos(x_5).^2.*sin(x_3).^2.*1.351412437400607e-10+cos(x_3).^2.*cos(x_6).^2.*sin(x_3).^2.*1.351412437400607e-10)+(x_7.*x_9.*cos(x_3).*cos(x_5).*sin(x_3).^4.*sin(x_5).^3.*1.273148214807934e-19)./(cos(x_3).^4.*3.79080679921875e-6+sin(x_3).^4.*3.79080679921875e-6+cos(x_3).^4.*cos(x_4).^2.*6.757062187003037e-11+cos(x_3).^4.*cos(x_5).^2.*6.757062187003037e-11+cos(x_3).^4.*cos(x_6).^2.*6.757062187003037e-11+cos(x_3).^2.*sin(x_3).^2.*7.5816135984375e-6+cos(x_4).^2.*sin(x_3).^4.*6.757062187003037e-11+cos(x_5).^2.*sin(x_3).^4.*6.757062187003037e-11+cos(x_6).^2.*sin(x_3).^4.*6.757062187003037e-11+cos(x_3).^2.*cos(x_4).^2.*sin(x_3).^2.*1.351412437400607e-10+cos(x_3).^2.*cos(x_5).^2.*sin(x_3).^2.*1.351412437400607e-10+cos(x_3).^2.*cos(x_6).^2.*sin(x_3).^2.*1.351412437400607e-10)+(x_7.*x_9.*cos(x_3).^2.*cos(x_6).*sin(x_3).^3.*sin(x_6).*4.123968090108961e-15)./(cos(x_3).^4.*3.79080679921875e-6+sin(x_3).^4.*3.79080679921875e-6+cos(x_3).^4.*cos(x_4).^2.*6.757062187003037e-11+cos(x_3).^4.*cos(x_5).^2.*6.757062187003037e-11+cos(x_3).^4.*cos(x_6).^2.*6.757062187003037e-11+cos(x_3).^2.*sin(x_3).^2.*7.5816135984375e-6+cos(x_4).^2.*sin(x_3).^4.*6.757062187003037e-11+cos(x_5).^2.*sin(x_3).^4.*6.757062187003037e-11+cos(x_6).^2.*sin(x_3).^4.*6.757062187003037e-11+cos(x_3).^2.*cos(x_4).^2.*sin(x_3).^2.*1.351412437400607e-10+cos(x_3).^2.*cos(x_5).^2.*sin(x_3).^2.*1.351412437400607e-10+cos(x_3).^2.*cos(x_6).^2.*sin(x_3).^2.*1.351412437400607e-10)+(x_7.*x_9.*cos(x_3).^3.*cos(x_6).*sin(x_3).^2.*sin(x_6).*7.142922260861507e-15)./(cos(x_3).^4.*3.79080679921875e-6+sin(x_3).^4.*3.79080679921875e-6+cos(x_3).^4.*cos(x_4).^2.*6.757062187003037e-11+cos(x_3).^4.*cos(x_5).^2.*6.757062187003037e-11+cos(x_3).^4.*cos(x_6).^2.*6.757062187003037e-11+cos(x_3).^2.*sin(x_3).^2.*7.5816135984375e-6+cos(x_4).^2.*sin(x_3).^4.*6.757062187003037e-11+cos(x_5).^2.*sin(x_3).^4.*6.757062187003037e-11+cos(x_6).^2.*sin(x_3).^4.*6.757062187003037e-11+cos(x_3).^2.*cos(x_4).^2.*sin(x_3).^2.*1.351412437400607e-10+cos(x_3).^2.*cos(x_5).^2.*sin(x_3).^2.*1.351412437400607e-10+cos(x_3).^2.*cos(x_6).^2.*sin(x_3).^2.*1.351412437400607e-10)-(x_7.*x_9.*cos(x_3).^4.*cos(x_4).*sin(x_3).*sin(x_4).^5.*1.310151082203454e-24)./(cos(x_3).^4.*3.79080679921875e-6+sin(x_3).^4.*3.79080679921875e-6+cos(x_3).^4.*cos(x_4).^2.*6.757062187003037e-11+cos(x_3).^4.*cos(x_5).^2.*6.757062187003037e-11+cos(x_3).^4.*cos(x_6).^2.*6.757062187003037e-11+cos(x_3).^2.*sin(x_3).^2.*7.5816135984375e-6+cos(x_4).^2.*sin(x_3).^4.*6.757062187003037e-11+cos(x_5).^2.*sin(x_3).^4.*6.757062187003037e-11+cos(x_6).^2.*sin(x_3).^4.*6.757062187003037e-11+cos(x_3).^2.*cos(x_4).^2.*sin(x_3).^2.*1.351412437400607e-10+cos(x_3).^2.*cos(x_5).^2.*sin(x_3).^2.*1.351412437400607e-10+cos(x_3).^2.*cos(x_6).^2.*sin(x_3).^2.*1.351412437400607e-10)-(x_7.*x_9.*cos(x_3).^4.*cos(x_5).*sin(x_3).*sin(x_5).^3.*7.350524645376524e-20)./(cos(x_3).^4.*3.79080679921875e-6+sin(x_3).^4.*3.79080679921875e-6+cos(x_3).^4.*cos(x_4).^2.*6.757062187003037e-11+cos(x_3).^4.*cos(x_5).^2.*6.757062187003037e-11+cos(x_3).^4.*cos(x_6).^2.*6.757062187003037e-11+cos(x_3).^2.*sin(x_3).^2.*7.5816135984375e-6+cos(x_4).^2.*sin(x_3).^4.*6.757062187003037e-11+cos(x_5).^2.*sin(x_3).^4.*6.757062187003037e-11+cos(x_6).^2.*sin(x_3).^4.*6.757062187003037e-11+cos(x_3).^2.*cos(x_4).^2.*sin(x_3).^2.*1.351412437400607e-10+cos(x_3).^2.*cos(x_5).^2.*sin(x_3).^2.*1.351412437400607e-10+cos(x_3).^2.*cos(x_6).^2.*sin(x_3).^2.*1.351412437400607e-10)+(x_7.*x_9.*cos(x_3).^5.*cos(x_5).*sin(x_4).^2.*sin(x_5).*1.273148214807934e-19)./(cos(x_3).^4.*3.79080679921875e-6+sin(x_3).^4.*3.79080679921875e-6+cos(x_3).^4.*cos(x_4).^2.*6.757062187003037e-11+cos(x_3).^4.*cos(x_5).^2.*6.757062187003037e-11+cos(x_3).^4.*cos(x_6).^2.*6.757062187003037e-11+cos(x_3).^2.*sin(x_3).^2.*7.5816135984375e-6+cos(x_4).^2.*sin(x_3).^4.*6.757062187003037e-11+cos(x_5).^2.*sin(x_3).^4.*6.757062187003037e-11+cos(x_6).^2.*sin(x_3).^4.*6.757062187003037e-11+cos(x_3).^2.*cos(x_4).^2.*sin(x_3).^2.*1.351412437400607e-10+cos(x_3).^2.*cos(x_5).^2.*sin(x_3).^2.*1.351412437400607e-10+cos(x_3).^2.*cos(x_6).^2.*sin(x_3).^2.*1.351412437400607e-10)+(x_8.*x_9.*cos(x_3).*cos(x_4).*sin(x_3).^4.*sin(x_4).^5.*1.310151082203454e-24)./(cos(x_3).^4.*3.79080679921875e-6+sin(x_3).^4.*3.79080679921875e-6+cos(x_3).^4.*cos(x_4).^2.*6.757062187003037e-11+cos(x_3).^4.*cos(x_5).^2.*6.757062187003037e-11+cos(x_3).^4.*cos(x_6).^2.*6.757062187003037e-11+cos(x_3).^2.*sin(x_3).^2.*7.5816135984375e-6+cos(x_4).^2.*sin(x_3).^4.*6.757062187003037e-11+cos(x_5).^2.*sin(x_3).^4.*6.757062187003037e-11+cos(x_6).^2.*sin(x_3).^4.*6.757062187003037e-11+cos(x_3).^2.*cos(x_4).^2.*sin(x_3).^2.*1.351412437400607e-10+cos(x_3).^2.*cos(x_5).^2.*sin(x_3).^2.*1.351412437400607e-10+cos(x_3).^2.*cos(x_6).^2.*sin(x_3).^2.*1.351412437400607e-10)+(x_8.*x_9.*cos(x_3).*cos(x_5).*sin(x_3).^4.*sin(x_5).^3.*7.350524645376524e-20)./(cos(x_3).^4.*3.79080679921875e-6+sin(x_3).^4.*3.79080679921875e-6+cos(x_3).^4.*cos(x_4).^2.*6.757062187003037e-11+cos(x_3).^4.*cos(x_5).^2.*6.757062187003037e-11+cos(x_3).^4.*cos(x_6).^2.*6.757062187003037e-11+cos(x_3).^2.*sin(x_3).^2.*7.5816135984375e-6+cos(x_4).^2.*sin(x_3).^4.*6.757062187003037e-11+cos(x_5).^2.*sin(x_3).^4.*6.757062187003037e-11+cos(x_6).^2.*sin(x_3).^4.*6.757062187003037e-11+cos(x_3).^2.*cos(x_4).^2.*sin(x_3).^2.*1.351412437400607e-10+cos(x_3).^2.*cos(x_5).^2.*sin(x_3).^2.*1.351412437400607e-10+cos(x_3).^2.*cos(x_6).^2.*sin(x_3).^2.*1.351412437400607e-10)+(x_8.*x_9.*cos(x_3).^2.*cos(x_6).*sin(x_3).^3.*sin(x_6).*7.142922260861507e-15)./(cos(x_3).^4.*3.79080679921875e-6+sin(x_3).^4.*3.79080679921875e-6+cos(x_3).^4.*cos(x_4).^2.*6.757062187003037e-11+cos(x_3).^4.*cos(x_5).^2.*6.757062187003037e-11+cos(x_3).^4.*cos(x_6).^2.*6.757062187003037e-11+cos(x_3).^2.*sin(x_3).^2.*7.5816135984375e-6+cos(x_4).^2.*sin(x_3).^4.*6.757062187003037e-11+cos(x_5).^2.*sin(x_3).^4.*6.757062187003037e-11+cos(x_6).^2.*sin(x_3).^4.*6.757062187003037e-11+cos(x_3).^2.*cos(x_4).^2.*sin(x_3).^2.*1.351412437400607e-10+cos(x_3).^2.*cos(x_5).^2.*sin(x_3).^2.*1.351412437400607e-10+cos(x_3).^2.*cos(x_6).^2.*sin(x_3).^2.*1.351412437400607e-10)-(x_8.*x_9.*cos(x_3).^3.*cos(x_6).*sin(x_3).^2.*sin(x_6).*4.123968090108961e-15)./(cos(x_3).^4.*3.79080679921875e-6+sin(x_3).^4.*3.79080679921875e-6+cos(x_3).^4.*cos(x_4).^2.*6.757062187003037e-11+cos(x_3).^4.*cos(x_5).^2.*6.757062187003037e-11+cos(x_3).^4.*cos(x_6).^2.*6.757062187003037e-11+cos(x_3).^2.*sin(x_3).^2.*7.5816135984375e-6+cos(x_4).^2.*sin(x_3).^4.*6.757062187003037e-11+cos(x_5).^2.*sin(x_3).^4.*6.757062187003037e-11+cos(x_6).^2.*sin(x_3).^4.*6.757062187003037e-11+cos(x_3).^2.*cos(x_4).^2.*sin(x_3).^2.*1.351412437400607e-10+cos(x_3).^2.*cos(x_5).^2.*sin(x_3).^2.*1.351412437400607e-10+cos(x_3).^2.*cos(x_6).^2.*sin(x_3).^2.*1.351412437400607e-10)+(x_8.*x_9.*cos(x_3).^4.*cos(x_5).*sin(x_3).*sin(x_5).^3.*1.273148214807934e-19)./(cos(x_3).^4.*3.79080679921875e-6+sin(x_3).^4.*3.79080679921875e-6+cos(x_3).^4.*cos(x_4).^2.*6.757062187003037e-11+cos(x_3).^4.*cos(x_5).^2.*6.757062187003037e-11+cos(x_3).^4.*cos(x_6).^2.*6.757062187003037e-11+cos(x_3).^2.*sin(x_3).^2.*7.5816135984375e-6+cos(x_4).^2.*sin(x_3).^4.*6.757062187003037e-11+cos(x_5).^2.*sin(x_3).^4.*6.757062187003037e-11+cos(x_6).^2.*sin(x_3).^4.*6.757062187003037e-11+cos(x_3).^2.*cos(x_4).^2.*sin(x_3).^2.*1.351412437400607e-10+cos(x_3).^2.*cos(x_5).^2.*sin(x_3).^2.*1.351412437400607e-10+cos(x_3).^2.*cos(x_6).^2.*sin(x_3).^2.*1.351412437400607e-10)-(x_8.*x_9.*cos(x_3).^5.*cos(x_4).*sin(x_4).*sin(x_5).^2.*1.470104929075305e-19)./(cos(x_3).^4.*3.79080679921875e-6+sin(x_3).^4.*3.79080679921875e-6+cos(x_3).^4.*cos(x_4).^2.*6.757062187003037e-11+cos(x_3).^4.*cos(x_5).^2.*6.757062187003037e-11+cos(x_3).^4.*cos(x_6).^2.*6.757062187003037e-11+cos(x_3).^2.*sin(x_3).^2.*7.5816135984375e-6+cos(x_4).^2.*sin(x_3).^4.*6.757062187003037e-11+cos(x_5).^2.*sin(x_3).^4.*6.757062187003037e-11+cos(x_6).^2.*sin(x_3).^4.*6.757062187003037e-11+cos(x_3).^2.*cos(x_4).^2.*sin(x_3).^2.*1.351412437400607e-10+cos(x_3).^2.*cos(x_5).^2.*sin(x_3).^2.*1.351412437400607e-10+cos(x_3).^2.*cos(x_6).^2.*sin(x_3).^2.*1.351412437400607e-10)-(x_7.*x_9.*cos(x_3).*cos(x_5).*sin(x_3).^4.*sin(x_5).^5.*1.134624119983866e-24)./(cos(x_3).^4.*3.79080679921875e-6+sin(x_3).^4.*3.79080679921875e-6+cos(x_3).^4.*cos(x_4).^2.*6.757062187003037e-11+cos(x_3).^4.*cos(x_5).^2.*6.757062187003037e-11+cos(x_3).^4.*cos(x_6).^2.*6.757062187003037e-11+cos(x_3).^2.*sin(x_3).^2.*7.5816135984375e-6+cos(x_4).^2.*sin(x_3).^4.*6.757062187003037e-11+cos(x_5).^2.*sin(x_3).^4.*6.757062187003037e-11+cos(x_6).^2.*sin(x_3).^4.*6.757062187003037e-11+cos(x_3).^2.*cos(x_4).^2.*sin(x_3).^2.*1.351412437400607e-10+cos(x_3).^2.*cos(x_5).^2.*sin(x_3).^2.*1.351412437400607e-10+cos(x_3).^2.*cos(x_6).^2.*sin(x_3).^2.*1.351412437400607e-10)-(x_7.*x_9.*cos(x_3).*cos(x_6).*sin(x_3).^4.*sin(x_6).^3.*1.273148214807934e-19)./(cos(x_3).^4.*3.79080679921875e-6+sin(x_3).^4.*3.79080679921875e-6+cos(x_3).^4.*cos(x_4).^2.*6.757062187003037e-11+cos(x_3).^4.*cos(x_5).^2.*6.757062187003037e-11+cos(x_3).^4.*cos(x_6).^2.*6.757062187003037e-11+cos(x_3).^2.*sin(x_3).^2.*7.5816135984375e-6+cos(x_4).^2.*sin(x_3).^4.*6.757062187003037e-11+cos(x_5).^2.*sin(x_3).^4.*6.757062187003037e-11+cos(x_6).^2.*sin(x_3).^4.*6.757062187003037e-11+cos(x_3).^2.*cos(x_4).^2.*sin(x_3).^2.*1.351412437400607e-10+cos(x_3).^2.*cos(x_5).^2.*sin(x_3).^2.*1.351412437400607e-10+cos(x_3).^2.*cos(x_6).^2.*sin(x_3).^2.*1.351412437400607e-10)+(x_7.*x_9.*cos(x_3).^4.*cos(x_5).*sin(x_3).*sin(x_5).^5.*6.550755411017271e-25)./(cos(x_3).^4.*3.79080679921875e-6+sin(x_3).^4.*3.79080679921875e-6+cos(x_3).^4.*cos(x_4).^2.*6.757062187003037e-11+cos(x_3).^4.*cos(x_5).^2.*6.757062187003037e-11+cos(x_3).^4.*cos(x_6).^2.*6.757062187003037e-11+cos(x_3).^2.*sin(x_3).^2.*7.5816135984375e-6+cos(x_4).^2.*sin(x_3).^4.*6.757062187003037e-11+cos(x_5).^2.*sin(x_3).^4.*6.757062187003037e-11+cos(x_6).^2.*sin(x_3).^4.*6.757062187003037e-11+cos(x_3).^2.*cos(x_4).^2.*sin(x_3).^2.*1.351412437400607e-10+cos(x_3).^2.*cos(x_5).^2.*sin(x_3).^2.*1.351412437400607e-10+cos(x_3).^2.*cos(x_6).^2.*sin(x_3).^2.*1.351412437400607e-10)-(x_7.*x_9.*cos(x_3).^4.*cos(x_6).*sin(x_3).*sin(x_6).^3.*7.350524645376524e-20)./(cos(x_3).^4.*3.79080679921875e-6+sin(x_3).^4.*3.79080679921875e-6+cos(x_3).^4.*cos(x_4).^2.*6.757062187003037e-11+cos(x_3).^4.*cos(x_5).^2.*6.757062187003037e-11+cos(x_3).^4.*cos(x_6).^2.*6.757062187003037e-11+cos(x_3).^2.*sin(x_3).^2.*7.5816135984375e-6+cos(x_4).^2.*sin(x_3).^4.*6.757062187003037e-11+cos(x_5).^2.*sin(x_3).^4.*6.757062187003037e-11+cos(x_6).^2.*sin(x_3).^4.*6.757062187003037e-11+cos(x_3).^2.*cos(x_4).^2.*sin(x_3).^2.*1.351412437400607e-10+cos(x_3).^2.*cos(x_5).^2.*sin(x_3).^2.*1.351412437400607e-10+cos(x_3).^2.*cos(x_6).^2.*sin(x_3).^2.*1.351412437400607e-10)-(x_8.*x_9.*cos(x_3).^5.*cos(x_4).*sin(x_4).*sin(x_6).^2.*1.470104929075305e-19)./(cos(x_3).^4.*3.79080679921875e-6+sin(x_3).^4.*3.79080679921875e-6+cos(x_3).^4.*cos(x_4).^2.*6.757062187003037e-11+cos(x_3).^4.*cos(x_5).^2.*6.757062187003037e-11+cos(x_3).^4.*cos(x_6).^2.*6.757062187003037e-11+cos(x_3).^2.*sin(x_3).^2.*7.5816135984375e-6+cos(x_4).^2.*sin(x_3).^4.*6.757062187003037e-11+cos(x_5).^2.*sin(x_3).^4.*6.757062187003037e-11+cos(x_6).^2.*sin(x_3).^4.*6.757062187003037e-11+cos(x_3).^2.*cos(x_4).^2.*sin(x_3).^2.*1.351412437400607e-10+cos(x_3).^2.*cos(x_5).^2.*sin(x_3).^2.*1.351412437400607e-10+cos(x_3).^2.*cos(x_6).^2.*sin(x_3).^2.*1.351412437400607e-10)+(x_8.*x_9.*cos(x_3).^5.*cos(x_5).*sin(x_4).^2.*sin(x_5).*7.350524645376524e-20)./(cos(x_3).^4.*3.79080679921875e-6+sin(x_3).^4.*3.79080679921875e-6+cos(x_3).^4.*cos(x_4).^2.*6.757062187003037e-11+cos(x_3).^4.*cos(x_5).^2.*6.757062187003037e-11+cos(x_3).^4.*cos(x_6).^2.*6.757062187003037e-11+cos(x_3).^2.*sin(x_3).^2.*7.5816135984375e-6+cos(x_4).^2.*sin(x_3).^4.*6.757062187003037e-11+cos(x_5).^2.*sin(x_3).^4.*6.757062187003037e-11+cos(x_6).^2.*sin(x_3).^4.*6.757062187003037e-11+cos(x_3).^2.*cos(x_4).^2.*sin(x_3).^2.*1.351412437400607e-10+cos(x_3).^2.*cos(x_5).^2.*sin(x_3).^2.*1.351412437400607e-10+cos(x_3).^2.*cos(x_6).^2.*sin(x_3).^2.*1.351412437400607e-10)+(x_7.*x_9.*cos(x_3).^5.*cos(x_5).*sin(x_5).*sin(x_6).^2.*1.273148214807934e-19)./(cos(x_3).^4.*3.79080679921875e-6+sin(x_3).^4.*3.79080679921875e-6+cos(x_3).^4.*cos(x_4).^2.*6.757062187003037e-11+cos(x_3).^4.*cos(x_5).^2.*6.757062187003037e-11+cos(x_3).^4.*cos(x_6).^2.*6.757062187003037e-11+cos(x_3).^2.*sin(x_3).^2.*7.5816135984375e-6+cos(x_4).^2.*sin(x_3).^4.*6.757062187003037e-11+cos(x_5).^2.*sin(x_3).^4.*6.757062187003037e-11+cos(x_6).^2.*sin(x_3).^4.*6.757062187003037e-11+cos(x_3).^2.*cos(x_4).^2.*sin(x_3).^2.*1.351412437400607e-10+cos(x_3).^2.*cos(x_5).^2.*sin(x_3).^2.*1.351412437400607e-10+cos(x_3).^2.*cos(x_6).^2.*sin(x_3).^2.*1.351412437400607e-10)-(x_7.*x_9.*cos(x_3).^5.*cos(x_5).*sin(x_4).^4.*sin(x_5).*1.134624119983866e-24)./(cos(x_3).^4.*3.79080679921875e-6+sin(x_3).^4.*3.79080679921875e-6+cos(x_3).^4.*cos(x_4).^2.*6.757062187003037e-11+cos(x_3).^4.*cos(x_5).^2.*6.757062187003037e-11+cos(x_3).^4.*cos(x_6).^2.*6.757062187003037e-11+cos(x_3).^2.*sin(x_3).^2.*7.5816135984375e-6+cos(x_4).^2.*sin(x_3).^4.*6.757062187003037e-11+cos(x_5).^2.*sin(x_3).^4.*6.757062187003037e-11+cos(x_6).^2.*sin(x_3).^4.*6.757062187003037e-11+cos(x_3).^2.*cos(x_4).^2.*sin(x_3).^2.*1.351412437400607e-10+cos(x_3).^2.*cos(x_5).^2.*sin(x_3).^2.*1.351412437400607e-10+cos(x_3).^2.*cos(x_6).^2.*sin(x_3).^2.*1.351412437400607e-10)-(x_7.*x_9.*cos(x_3).^5.*cos(x_6).*sin(x_4).^2.*sin(x_6).*1.273148214807934e-19)./(cos(x_3).^4.*3.79080679921875e-6+sin(x_3).^4.*3.79080679921875e-6+cos(x_3).^4.*cos(x_4).^2.*6.757062187003037e-11+cos(x_3).^4.*cos(x_5).^2.*6.757062187003037e-11+cos(x_3).^4.*cos(x_6).^2.*6.757062187003037e-11+cos(x_3).^2.*sin(x_3).^2.*7.5816135984375e-6+cos(x_4).^2.*sin(x_3).^4.*6.757062187003037e-11+cos(x_5).^2.*sin(x_3).^4.*6.757062187003037e-11+cos(x_6).^2.*sin(x_3).^4.*6.757062187003037e-11+cos(x_3).^2.*cos(x_4).^2.*sin(x_3).^2.*1.351412437400607e-10+cos(x_3).^2.*cos(x_5).^2.*sin(x_3).^2.*1.351412437400607e-10+cos(x_3).^2.*cos(x_6).^2.*sin(x_3).^2.*1.351412437400607e-10)-(x_8.*x_9.*cos(x_3).*cos(x_5).*sin(x_3).^4.*sin(x_5).^5.*6.550755411017271e-25)./(cos(x_3).^4.*3.79080679921875e-6+sin(x_3).^4.*3.79080679921875e-6+cos(x_3).^4.*cos(x_4).^2.*6.757062187003037e-11+cos(x_3).^4.*cos(x_5).^2.*6.757062187003037e-11+cos(x_3).^4.*cos(x_6).^2.*6.757062187003037e-11+cos(x_3).^2.*sin(x_3).^2.*7.5816135984375e-6+cos(x_4).^2.*sin(x_3).^4.*6.757062187003037e-11+cos(x_5).^2.*sin(x_3).^4.*6.757062187003037e-11+cos(x_6).^2.*sin(x_3).^4.*6.757062187003037e-11+cos(x_3).^2.*cos(x_4).^2.*sin(x_3).^2.*1.351412437400607e-10+cos(x_3).^2.*cos(x_5).^2.*sin(x_3).^2.*1.351412437400607e-10+cos(x_3).^2.*cos(x_6).^2.*sin(x_3).^2.*1.351412437400607e-10)+(x_8.*x_9.*cos(x_3).*cos(x_6).*sin(x_3).^4.*sin(x_6).^3.*7.350524645376524e-20)./(cos(x_3).^4.*3.79080679921875e-6+sin(x_3).^4.*3.79080679921875e-6+cos(x_3).^4.*cos(x_4).^2.*6.757062187003037e-11+cos(x_3).^4.*cos(x_5).^2.*6.757062187003037e-11+cos(x_3).^4.*cos(x_6).^2.*6.757062187003037e-11+cos(x_3).^2.*sin(x_3).^2.*7.5816135984375e-6+cos(x_4).^2.*sin(x_3).^4.*6.757062187003037e-11+cos(x_5).^2.*sin(x_3).^4.*6.757062187003037e-11+cos(x_6).^2.*sin(x_3).^4.*6.757062187003037e-11+cos(x_3).^2.*cos(x_4).^2.*sin(x_3).^2.*1.351412437400607e-10+cos(x_3).^2.*cos(x_5).^2.*sin(x_3).^2.*1.351412437400607e-10+cos(x_3).^2.*cos(x_6).^2.*sin(x_3).^2.*1.351412437400607e-10)-(x_8.*x_9.*cos(x_3).^4.*cos(x_5).*sin(x_3).*sin(x_5).^5.*1.134624119983866e-24)./(cos(x_3).^4.*3.79080679921875e-6+sin(x_3).^4.*3.79080679921875e-6+cos(x_3).^4.*cos(x_4).^2.*6.757062187003037e-11+cos(x_3).^4.*cos(x_5).^2.*6.757062187003037e-11+cos(x_3).^4.*cos(x_6).^2.*6.757062187003037e-11+cos(x_3).^2.*sin(x_3).^2.*7.5816135984375e-6+cos(x_4).^2.*sin(x_3).^4.*6.757062187003037e-11+cos(x_5).^2.*sin(x_3).^4.*6.757062187003037e-11+cos(x_6).^2.*sin(x_3).^4.*6.757062187003037e-11+cos(x_3).^2.*cos(x_4).^2.*sin(x_3).^2.*1.351412437400607e-10+cos(x_3).^2.*cos(x_5).^2.*sin(x_3).^2.*1.351412437400607e-10+cos(x_3).^2.*cos(x_6).^2.*sin(x_3).^2.*1.351412437400607e-10)-(x_8.*x_9.*cos(x_3).^4.*cos(x_6).*sin(x_3).*sin(x_6).^3.*1.273148214807934e-19)./(cos(x_3).^4.*3.79080679921875e-6+sin(x_3).^4.*3.79080679921875e-6+cos(x_3).^4.*cos(x_4).^2.*6.757062187003037e-11+cos(x_3).^4.*cos(x_5).^2.*6.757062187003037e-11+cos(x_3).^4.*cos(x_6).^2.*6.757062187003037e-11+cos(x_3).^2.*sin(x_3).^2.*7.5816135984375e-6+cos(x_4).^2.*sin(x_3).^4.*6.757062187003037e-11+cos(x_5).^2.*sin(x_3).^4.*6.757062187003037e-11+cos(x_6).^2.*sin(x_3).^4.*6.757062187003037e-11+cos(x_3).^2.*cos(x_4).^2.*sin(x_3).^2.*1.351412437400607e-10+cos(x_3).^2.*cos(x_5).^2.*sin(x_3).^2.*1.351412437400607e-10+cos(x_3).^2.*cos(x_6).^2.*sin(x_3).^2.*1.351412437400607e-10)+(x_8.*x_9.*cos(x_3).^5.*cos(x_4).*sin(x_4).*sin(x_5).^4.*1.310151082203454e-24)./(cos(x_3).^4.*3.79080679921875e-6+sin(x_3).^4.*3.79080679921875e-6+cos(x_3).^4.*cos(x_4).^2.*6.757062187003037e-11+cos(x_3).^4.*cos(x_5).^2.*6.757062187003037e-11+cos(x_3).^4.*cos(x_6).^2.*6.757062187003037e-11+cos(x_3).^2.*sin(x_3).^2.*7.5816135984375e-6+cos(x_4).^2.*sin(x_3).^4.*6.757062187003037e-11+cos(x_5).^2.*sin(x_3).^4.*6.757062187003037e-11+cos(x_6).^2.*sin(x_3).^4.*6.757062187003037e-11+cos(x_3).^2.*cos(x_4).^2.*sin(x_3).^2.*1.351412437400607e-10+cos(x_3).^2.*cos(x_5).^2.*sin(x_3).^2.*1.351412437400607e-10+cos(x_3).^2.*cos(x_6).^2.*sin(x_3).^2.*1.351412437400607e-10)+(x_7.*x_9.*cos(x_3).*cos(x_6).*sin(x_3).^4.*sin(x_6).^5.*1.134624119983866e-24)./(cos(x_3).^4.*3.79080679921875e-6+sin(x_3).^4.*3.79080679921875e-6+cos(x_3).^4.*cos(x_4).^2.*6.757062187003037e-11+cos(x_3).^4.*cos(x_5).^2.*6.757062187003037e-11+cos(x_3).^4.*cos(x_6).^2.*6.757062187003037e-11+cos(x_3).^2.*sin(x_3).^2.*7.5816135984375e-6+cos(x_4).^2.*sin(x_3).^4.*6.757062187003037e-11+cos(x_5).^2.*sin(x_3).^4.*6.757062187003037e-11+cos(x_6).^2.*sin(x_3).^4.*6.757062187003037e-11+cos(x_3).^2.*cos(x_4).^2.*sin(x_3).^2.*1.351412437400607e-10+cos(x_3).^2.*cos(x_5).^2.*sin(x_3).^2.*1.351412437400607e-10+cos(x_3).^2.*cos(x_6).^2.*sin(x_3).^2.*1.351412437400607e-10)+(x_7.*x_9.*cos(x_3).^4.*cos(x_6).*sin(x_3).*sin(x_6).^5.*6.550755411017271e-25)./(cos(x_3).^4.*3.79080679921875e-6+sin(x_3).^4.*3.79080679921875e-6+cos(x_3).^4.*cos(x_4).^2.*6.757062187003037e-11+cos(x_3).^4.*cos(x_5).^2.*6.757062187003037e-11+cos(x_3).^4.*cos(x_6).^2.*6.757062187003037e-11+cos(x_3).^2.*sin(x_3).^2.*7.5816135984375e-6+cos(x_4).^2.*sin(x_3).^4.*6.757062187003037e-11+cos(x_5).^2.*sin(x_3).^4.*6.757062187003037e-11+cos(x_6).^2.*sin(x_3).^4.*6.757062187003037e-11+cos(x_3).^2.*cos(x_4).^2.*sin(x_3).^2.*1.351412437400607e-10+cos(x_3).^2.*cos(x_5).^2.*sin(x_3).^2.*1.351412437400607e-10+cos(x_3).^2.*cos(x_6).^2.*sin(x_3).^2.*1.351412437400607e-10)-(x_7.*x_9.*cos(x_3).^5.*cos(x_6).*sin(x_5).^2.*sin(x_6).*1.273148214807934e-19)./(cos(x_3).^4.*3.79080679921875e-6+sin(x_3).^4.*3.79080679921875e-6+cos(x_3).^4.*cos(x_4).^2.*6.757062187003037e-11+cos(x_3).^4.*cos(x_5).^2.*6.757062187003037e-11+cos(x_3).^4.*cos(x_6).^2.*6.757062187003037e-11+cos(x_3).^2.*sin(x_3).^2.*7.5816135984375e-6+cos(x_4).^2.*sin(x_3).^4.*6.757062187003037e-11+cos(x_5).^2.*sin(x_3).^4.*6.757062187003037e-11+cos(x_6).^2.*sin(x_3).^4.*6.757062187003037e-11+cos(x_3).^2.*cos(x_4).^2.*sin(x_3).^2.*1.351412437400607e-10+cos(x_3).^2.*cos(x_5).^2.*sin(x_3).^2.*1.351412437400607e-10+cos(x_3).^2.*cos(x_6).^2.*sin(x_3).^2.*1.351412437400607e-10)+(x_8.*x_9.*cos(x_3).^5.*cos(x_4).*sin(x_4).*sin(x_6).^4.*1.310151082203454e-24)./(cos(x_3).^4.*3.79080679921875e-6+sin(x_3).^4.*3.79080679921875e-6+cos(x_3).^4.*cos(x_4).^2.*6.757062187003037e-11+cos(x_3).^4.*cos(x_5).^2.*6.757062187003037e-11+cos(x_3).^4.*cos(x_6).^2.*6.757062187003037e-11+cos(x_3).^2.*sin(x_3).^2.*7.5816135984375e-6+cos(x_4).^2.*sin(x_3).^4.*6.757062187003037e-11+cos(x_5).^2.*sin(x_3).^4.*6.757062187003037e-11+cos(x_6).^2.*sin(x_3).^4.*6.757062187003037e-11+cos(x_3).^2.*cos(x_4).^2.*sin(x_3).^2.*1.351412437400607e-10+cos(x_3).^2.*cos(x_5).^2.*sin(x_3).^2.*1.351412437400607e-10+cos(x_3).^2.*cos(x_6).^2.*sin(x_3).^2.*1.351412437400607e-10)+(x_8.*x_9.*cos(x_3).^5.*cos(x_5).*sin(x_5).*sin(x_6).^2.*7.350524645376524e-20)./(cos(x_3).^4.*3.79080679921875e-6+sin(x_3).^4.*3.79080679921875e-6+cos(x_3).^4.*cos(x_4).^2.*6.757062187003037e-11+cos(x_3).^4.*cos(x_5).^2.*6.757062187003037e-11+cos(x_3).^4.*cos(x_6).^2.*6.757062187003037e-11+cos(x_3).^2.*sin(x_3).^2.*7.5816135984375e-6+cos(x_4).^2.*sin(x_3).^4.*6.757062187003037e-11+cos(x_5).^2.*sin(x_3).^4.*6.757062187003037e-11+cos(x_6).^2.*sin(x_3).^4.*6.757062187003037e-11+cos(x_3).^2.*cos(x_4).^2.*sin(x_3).^2.*1.351412437400607e-10+cos(x_3).^2.*cos(x_5).^2.*sin(x_3).^2.*1.351412437400607e-10+cos(x_3).^2.*cos(x_6).^2.*sin(x_3).^2.*1.351412437400607e-10)-(x_8.*x_9.*cos(x_3).^5.*cos(x_5).*sin(x_4).^4.*sin(x_5).*6.550755411017271e-25)./(cos(x_3).^4.*3.79080679921875e-6+sin(x_3).^4.*3.79080679921875e-6+cos(x_3).^4.*cos(x_4).^2.*6.757062187003037e-11+cos(x_3).^4.*cos(x_5).^2.*6.757062187003037e-11+cos(x_3).^4.*cos(x_6).^2.*6.757062187003037e-11+cos(x_3).^2.*sin(x_3).^2.*7.5816135984375e-6+cos(x_4).^2.*sin(x_3).^4.*6.757062187003037e-11+cos(x_5).^2.*sin(x_3).^4.*6.757062187003037e-11+cos(x_6).^2.*sin(x_3).^4.*6.757062187003037e-11+cos(x_3).^2.*cos(x_4).^2.*sin(x_3).^2.*1.351412437400607e-10+cos(x_3).^2.*cos(x_5).^2.*sin(x_3).^2.*1.351412437400607e-10+cos(x_3).^2.*cos(x_6).^2.*sin(x_3).^2.*1.351412437400607e-10)+(x_8.*x_9.*cos(x_3).^5.*cos(x_6).*sin(x_4).^2.*sin(x_6).*7.350524645376524e-20)./(cos(x_3).^4.*3.79080679921875e-6+sin(x_3).^4.*3.79080679921875e-6+cos(x_3).^4.*cos(x_4).^2.*6.757062187003037e-11+cos(x_3).^4.*cos(x_5).^2.*6.757062187003037e-11+cos(x_3).^4.*cos(x_6).^2.*6.757062187003037e-11+cos(x_3).^2.*sin(x_3).^2.*7.5816135984375e-6+cos(x_4).^2.*sin(x_3).^4.*6.757062187003037e-11+cos(x_5).^2.*sin(x_3).^4.*6.757062187003037e-11+cos(x_6).^2.*sin(x_3).^4.*6.757062187003037e-11+cos(x_3).^2.*cos(x_4).^2.*sin(x_3).^2.*1.351412437400607e-10+cos(x_3).^2.*cos(x_5).^2.*sin(x_3).^2.*1.351412437400607e-10+cos(x_3).^2.*cos(x_6).^2.*sin(x_3).^2.*1.351412437400607e-10)-(x_7.*x_9.*cos(x_3).^5.*cos(x_5).*sin(x_5).*sin(x_6).^4.*1.134624119983866e-24)./(cos(x_3).^4.*3.79080679921875e-6+sin(x_3).^4.*3.79080679921875e-6+cos(x_3).^4.*cos(x_4).^2.*6.757062187003037e-11+cos(x_3).^4.*cos(x_5).^2.*6.757062187003037e-11+cos(x_3).^4.*cos(x_6).^2.*6.757062187003037e-11+cos(x_3).^2.*sin(x_3).^2.*7.5816135984375e-6+cos(x_4).^2.*sin(x_3).^4.*6.757062187003037e-11+cos(x_5).^2.*sin(x_3).^4.*6.757062187003037e-11+cos(x_6).^2.*sin(x_3).^4.*6.757062187003037e-11+cos(x_3).^2.*cos(x_4).^2.*sin(x_3).^2.*1.351412437400607e-10+cos(x_3).^2.*cos(x_5).^2.*sin(x_3).^2.*1.351412437400607e-10+cos(x_3).^2.*cos(x_6).^2.*sin(x_3).^2.*1.351412437400607e-10)+(x_7.*x_9.*cos(x_3).^5.*cos(x_6).*sin(x_4).^4.*sin(x_6).*1.134624119983866e-24)./(cos(x_3).^4.*3.79080679921875e-6+sin(x_3).^4.*3.79080679921875e-6+cos(x_3).^4.*cos(x_4).^2.*6.757062187003037e-11+cos(x_3).^4.*cos(x_5).^2.*6.757062187003037e-11+cos(x_3).^4.*cos(x_6).^2.*6.757062187003037e-11+cos(x_3).^2.*sin(x_3).^2.*7.5816135984375e-6+cos(x_4).^2.*sin(x_3).^4.*6.757062187003037e-11+cos(x_5).^2.*sin(x_3).^4.*6.757062187003037e-11+cos(x_6).^2.*sin(x_3).^4.*6.757062187003037e-11+cos(x_3).^2.*cos(x_4).^2.*sin(x_3).^2.*1.351412437400607e-10+cos(x_3).^2.*cos(x_5).^2.*sin(x_3).^2.*1.351412437400607e-10+cos(x_3).^2.*cos(x_6).^2.*sin(x_3).^2.*1.351412437400607e-10)-(x_8.*x_9.*cos(x_3).*cos(x_6).*sin(x_3).^4.*sin(x_6).^5.*6.550755411017271e-25)./(cos(x_3).^4.*3.79080679921875e-6+sin(x_3).^4.*3.79080679921875e-6+cos(x_3).^4.*cos(x_4).^2.*6.757062187003037e-11+cos(x_3).^4.*cos(x_5).^2.*6.757062187003037e-11+cos(x_3).^4.*cos(x_6).^2.*6.757062187003037e-11+cos(x_3).^2.*sin(x_3).^2.*7.5816135984375e-6+cos(x_4).^2.*sin(x_3).^4.*6.757062187003037e-11+cos(x_5).^2.*sin(x_3).^4.*6.757062187003037e-11+cos(x_6).^2.*sin(x_3).^4.*6.757062187003037e-11+cos(x_3).^2.*cos(x_4).^2.*sin(x_3).^2.*1.351412437400607e-10+cos(x_3).^2.*cos(x_5).^2.*sin(x_3).^2.*1.351412437400607e-10+cos(x_3).^2.*cos(x_6).^2.*sin(x_3).^2.*1.351412437400607e-10)+(x_8.*x_9.*cos(x_3).^4.*cos(x_6).*sin(x_3).*sin(x_6).^5.*1.134624119983866e-24)./(cos(x_3).^4.*3.79080679921875e-6+sin(x_3).^4.*3.79080679921875e-6+cos(x_3).^4.*cos(x_4).^2.*6.757062187003037e-11+cos(x_3).^4.*cos(x_5).^2.*6.757062187003037e-11+cos(x_3).^4.*cos(x_6).^2.*6.757062187003037e-11+cos(x_3).^2.*sin(x_3).^2.*7.5816135984375e-6+cos(x_4).^2.*sin(x_3).^4.*6.757062187003037e-11+cos(x_5).^2.*sin(x_3).^4.*6.757062187003037e-11+cos(x_6).^2.*sin(x_3).^4.*6.757062187003037e-11+cos(x_3).^2.*cos(x_4).^2.*sin(x_3).^2.*1.351412437400607e-10+cos(x_3).^2.*cos(x_5).^2.*sin(x_3).^2.*1.351412437400607e-10+cos(x_3).^2.*cos(x_6).^2.*sin(x_3).^2.*1.351412437400607e-10)+(x_8.*x_9.*cos(x_3).^5.*cos(x_6).*sin(x_5).^2.*sin(x_6).*7.350524645376524e-20)./(cos(x_3).^4.*3.79080679921875e-6+sin(x_3).^4.*3.79080679921875e-6+cos(x_3).^4.*cos(x_4).^2.*6.757062187003037e-11+cos(x_3).^4.*cos(x_5).^2.*6.757062187003037e-11+cos(x_3).^4.*cos(x_6).^2.*6.757062187003037e-11+cos(x_3).^2.*sin(x_3).^2.*7.5816135984375e-6+cos(x_4).^2.*sin(x_3).^4.*6.757062187003037e-11+cos(x_5).^2.*sin(x_3).^4.*6.757062187003037e-11+cos(x_6).^2.*sin(x_3).^4.*6.757062187003037e-11+cos(x_3).^2.*cos(x_4).^2.*sin(x_3).^2.*1.351412437400607e-10+cos(x_3).^2.*cos(x_5).^2.*sin(x_3).^2.*1.351412437400607e-10+cos(x_3).^2.*cos(x_6).^2.*sin(x_3).^2.*1.351412437400607e-10)+(x_7.*x_9.*cos(x_3).^5.*cos(x_6).*sin(x_5).^4.*sin(x_6).*1.134624119983866e-24)./(cos(x_3).^4.*3.79080679921875e-6+sin(x_3).^4.*3.79080679921875e-6+cos(x_3).^4.*cos(x_4).^2.*6.757062187003037e-11+cos(x_3).^4.*cos(x_5).^2.*6.757062187003037e-11+cos(x_3).^4.*cos(x_6).^2.*6.757062187003037e-11+cos(x_3).^2.*sin(x_3).^2.*7.5816135984375e-6+cos(x_4).^2.*sin(x_3).^4.*6.757062187003037e-11+cos(x_5).^2.*sin(x_3).^4.*6.757062187003037e-11+cos(x_6).^2.*sin(x_3).^4.*6.757062187003037e-11+cos(x_3).^2.*cos(x_4).^2.*sin(x_3).^2.*1.351412437400607e-10+cos(x_3).^2.*cos(x_5).^2.*sin(x_3).^2.*1.351412437400607e-10+cos(x_3).^2.*cos(x_6).^2.*sin(x_3).^2.*1.351412437400607e-10)-(x_8.*x_9.*cos(x_3).^5.*cos(x_5).*sin(x_5).*sin(x_6).^4.*6.550755411017271e-25)./(cos(x_3).^4.*3.79080679921875e-6+sin(x_3).^4.*3.79080679921875e-6+cos(x_3).^4.*cos(x_4).^2.*6.757062187003037e-11+cos(x_3).^4.*cos(x_5).^2.*6.757062187003037e-11+cos(x_3).^4.*cos(x_6).^2.*6.757062187003037e-11+cos(x_3).^2.*sin(x_3).^2.*7.5816135984375e-6+cos(x_4).^2.*sin(x_3).^4.*6.757062187003037e-11+cos(x_5).^2.*sin(x_3).^4.*6.757062187003037e-11+cos(x_6).^2.*sin(x_3).^4.*6.757062187003037e-11+cos(x_3).^2.*cos(x_4).^2.*sin(x_3).^2.*1.351412437400607e-10+cos(x_3).^2.*cos(x_5).^2.*sin(x_3).^2.*1.351412437400607e-10+cos(x_3).^2.*cos(x_6).^2.*sin(x_3).^2.*1.351412437400607e-10)-(x_8.*x_9.*cos(x_3).^5.*cos(x_6).*sin(x_4).^4.*sin(x_6).*6.550755411017271e-25)./(cos(x_3).^4.*3.79080679921875e-6+sin(x_3).^4.*3.79080679921875e-6+cos(x_3).^4.*cos(x_4).^2.*6.757062187003037e-11+cos(x_3).^4.*cos(x_5).^2.*6.757062187003037e-11+cos(x_3).^4.*cos(x_6).^2.*6.757062187003037e-11+cos(x_3).^2.*sin(x_3).^2.*7.5816135984375e-6+cos(x_4).^2.*sin(x_3).^4.*6.757062187003037e-11+cos(x_5).^2.*sin(x_3).^4.*6.757062187003037e-11+cos(x_6).^2.*sin(x_3).^4.*6.757062187003037e-11+cos(x_3).^2.*cos(x_4).^2.*sin(x_3).^2.*1.351412437400607e-10+cos(x_3).^2.*cos(x_5).^2.*sin(x_3).^2.*1.351412437400607e-10+cos(x_3).^2.*cos(x_6).^2.*sin(x_3).^2.*1.351412437400607e-10)-(x_8.*x_9.*cos(x_3).^5.*cos(x_6).*sin(x_5).^4.*sin(x_6).*6.550755411017271e-25)./(cos(x_3).^4.*3.79080679921875e-6+sin(x_3).^4.*3.79080679921875e-6+cos(x_3).^4.*cos(x_4).^2.*6.757062187003037e-11+cos(x_3).^4.*cos(x_5).^2.*6.757062187003037e-11+cos(x_3).^4.*cos(x_6).^2.*6.757062187003037e-11+cos(x_3).^2.*sin(x_3).^2.*7.5816135984375e-6+cos(x_4).^2.*sin(x_3).^4.*6.757062187003037e-11+cos(x_5).^2.*sin(x_3).^4.*6.757062187003037e-11+cos(x_6).^2.*sin(x_3).^4.*6.757062187003037e-11+cos(x_3).^2.*cos(x_4).^2.*sin(x_3).^2.*1.351412437400607e-10+cos(x_3).^2.*cos(x_5).^2.*sin(x_3).^2.*1.351412437400607e-10+cos(x_3).^2.*cos(x_6).^2.*sin(x_3).^2.*1.351412437400607e-10)+(x_7.*x_9.*cos(x_3).^2.*cos(x_4).*sin(x_3).^2.*sin(x_4).*2.46366703632003e-13)./(cos(x_3).^4.*1.5163227196875e-5+sin(x_3).^4.*1.5163227196875e-5+cos(x_3).^4.*cos(x_4).^2.*2.702824874801215e-10+cos(x_3).^4.*cos(x_5).^2.*2.702824874801215e-10+cos(x_3).^4.*cos(x_6).^2.*2.702824874801215e-10+cos(x_3).^2.*sin(x_3).^2.*3.032645439375e-5+cos(x_4).^2.*sin(x_3).^4.*2.702824874801215e-10+cos(x_5).^2.*sin(x_3).^4.*2.702824874801215e-10+cos(x_6).^2.*sin(x_3).^4.*2.702824874801215e-10+cos(x_3).^2.*cos(x_4).^2.*sin(x_3).^2.*5.40564974960243e-10+cos(x_3).^2.*cos(x_5).^2.*sin(x_3).^2.*5.40564974960243e-10+cos(x_3).^2.*cos(x_6).^2.*sin(x_3).^2.*5.40564974960243e-10)+(x_8.*x_9.*cos(x_3).^2.*cos(x_4).*sin(x_3).^2.*sin(x_4).*2.46366703632003e-13)./(cos(x_3).^4.*1.5163227196875e-5+sin(x_3).^4.*1.5163227196875e-5+cos(x_3).^4.*cos(x_4).^2.*2.702824874801215e-10+cos(x_3).^4.*cos(x_5).^2.*2.702824874801215e-10+cos(x_3).^4.*cos(x_6).^2.*2.702824874801215e-10+cos(x_3).^2.*sin(x_3).^2.*3.032645439375e-5+cos(x_4).^2.*sin(x_3).^4.*2.702824874801215e-10+cos(x_5).^2.*sin(x_3).^4.*2.702824874801215e-10+cos(x_6).^2.*sin(x_3).^4.*2.702824874801215e-10+cos(x_3).^2.*cos(x_4).^2.*sin(x_3).^2.*5.40564974960243e-10+cos(x_3).^2.*cos(x_5).^2.*sin(x_3).^2.*5.40564974960243e-10+cos(x_3).^2.*cos(x_6).^2.*sin(x_3).^2.*5.40564974960243e-10)+(x_7.*x_9.*cos(x_3).*cos(x_4).*sin(x_3).^3.*sin(x_4).^3.*4.39121857220618e-18)./(cos(x_3).^4.*1.5163227196875e-5+sin(x_3).^4.*1.5163227196875e-5+cos(x_3).^4.*cos(x_4).^2.*2.702824874801215e-10+cos(x_3).^4.*cos(x_5).^2.*2.702824874801215e-10+cos(x_3).^4.*cos(x_6).^2.*2.702824874801215e-10+cos(x_3).^2.*sin(x_3).^2.*3.032645439375e-5+cos(x_4).^2.*sin(x_3).^4.*2.702824874801215e-10+cos(x_5).^2.*sin(x_3).^4.*2.702824874801215e-10+cos(x_6).^2.*sin(x_3).^4.*2.702824874801215e-10+cos(x_3).^2.*cos(x_4).^2.*sin(x_3).^2.*5.40564974960243e-10+cos(x_3).^2.*cos(x_5).^2.*sin(x_3).^2.*5.40564974960243e-10+cos(x_3).^2.*cos(x_6).^2.*sin(x_3).^2.*5.40564974960243e-10)-(x_7.*x_9.*cos(x_3).^2.*cos(x_5).*sin(x_3).^2.*sin(x_5).*3.36543175807948e-13)./(cos(x_3).^4.*1.5163227196875e-5+sin(x_3).^4.*1.5163227196875e-5+cos(x_3).^4.*cos(x_4).^2.*2.702824874801215e-10+cos(x_3).^4.*cos(x_5).^2.*2.702824874801215e-10+cos(x_3).^4.*cos(x_6).^2.*2.702824874801215e-10+cos(x_3).^2.*sin(x_3).^2.*3.032645439375e-5+cos(x_4).^2.*sin(x_3).^4.*2.702824874801215e-10+cos(x_5).^2.*sin(x_3).^4.*2.702824874801215e-10+cos(x_6).^2.*sin(x_3).^4.*2.702824874801215e-10+cos(x_3).^2.*cos(x_4).^2.*sin(x_3).^2.*5.40564974960243e-10+cos(x_3).^2.*cos(x_5).^2.*sin(x_3).^2.*5.40564974960243e-10+cos(x_3).^2.*cos(x_6).^2.*sin(x_3).^2.*5.40564974960243e-10)+(x_7.*x_9.*cos(x_3).^3.*cos(x_4).*sin(x_3).*sin(x_4).^3.*4.39121857220618e-18)./(cos(x_3).^4.*1.5163227196875e-5+sin(x_3).^4.*1.5163227196875e-5+cos(x_3).^4.*cos(x_4).^2.*2.702824874801215e-10+cos(x_3).^4.*cos(x_5).^2.*2.702824874801215e-10+cos(x_3).^4.*cos(x_6).^2.*2.702824874801215e-10+cos(x_3).^2.*sin(x_3).^2.*3.032645439375e-5+cos(x_4).^2.*sin(x_3).^4.*2.702824874801215e-10+cos(x_5).^2.*sin(x_3).^4.*2.702824874801215e-10+cos(x_6).^2.*sin(x_3).^4.*2.702824874801215e-10+cos(x_3).^2.*cos(x_4).^2.*sin(x_3).^2.*5.40564974960243e-10+cos(x_3).^2.*cos(x_5).^2.*sin(x_3).^2.*5.40564974960243e-10+cos(x_3).^2.*cos(x_6).^2.*sin(x_3).^2.*5.40564974960243e-10)+(x_8.*x_9.*cos(x_3).*cos(x_4).*sin(x_3).^3.*sin(x_4).^3.*4.39121857220618e-18)./(cos(x_3).^4.*1.5163227196875e-5+sin(x_3).^4.*1.5163227196875e-5+cos(x_3).^4.*cos(x_4).^2.*2.702824874801215e-10+cos(x_3).^4.*cos(x_5).^2.*2.702824874801215e-10+cos(x_3).^4.*cos(x_6).^2.*2.702824874801215e-10+cos(x_3).^2.*sin(x_3).^2.*3.032645439375e-5+cos(x_4).^2.*sin(x_3).^4.*2.702824874801215e-10+cos(x_5).^2.*sin(x_3).^4.*2.702824874801215e-10+cos(x_6).^2.*sin(x_3).^4.*2.702824874801215e-10+cos(x_3).^2.*cos(x_4).^2.*sin(x_3).^2.*5.40564974960243e-10+cos(x_3).^2.*cos(x_5).^2.*sin(x_3).^2.*5.40564974960243e-10+cos(x_3).^2.*cos(x_6).^2.*sin(x_3).^2.*5.40564974960243e-10)+(x_8.*x_9.*cos(x_3).^2.*cos(x_5).*sin(x_3).^2.*sin(x_5).*9.017647217594503e-14)./(cos(x_3).^4.*1.5163227196875e-5+sin(x_3).^4.*1.5163227196875e-5+cos(x_3).^4.*cos(x_4).^2.*2.702824874801215e-10+cos(x_3).^4.*cos(x_5).^2.*2.702824874801215e-10+cos(x_3).^4.*cos(x_6).^2.*2.702824874801215e-10+cos(x_3).^2.*sin(x_3).^2.*3.032645439375e-5+cos(x_4).^2.*sin(x_3).^4.*2.702824874801215e-10+cos(x_5).^2.*sin(x_3).^4.*2.702824874801215e-10+cos(x_6).^2.*sin(x_3).^4.*2.702824874801215e-10+cos(x_3).^2.*cos(x_4).^2.*sin(x_3).^2.*5.40564974960243e-10+cos(x_3).^2.*cos(x_5).^2.*sin(x_3).^2.*5.40564974960243e-10+cos(x_3).^2.*cos(x_6).^2.*sin(x_3).^2.*5.40564974960243e-10)+(x_8.*x_9.*cos(x_3).^3.*cos(x_4).*sin(x_3).*sin(x_4).^3.*4.39121857220618e-18)./(cos(x_3).^4.*1.5163227196875e-5+sin(x_3).^4.*1.5163227196875e-5+cos(x_3).^4.*cos(x_4).^2.*2.702824874801215e-10+cos(x_3).^4.*cos(x_5).^2.*2.702824874801215e-10+cos(x_3).^4.*cos(x_6).^2.*2.702824874801215e-10+cos(x_3).^2.*sin(x_3).^2.*3.032645439375e-5+cos(x_4).^2.*sin(x_3).^4.*2.702824874801215e-10+cos(x_5).^2.*sin(x_3).^4.*2.702824874801215e-10+cos(x_6).^2.*sin(x_3).^4.*2.702824874801215e-10+cos(x_3).^2.*cos(x_4).^2.*sin(x_3).^2.*5.40564974960243e-10+cos(x_3).^2.*cos(x_5).^2.*sin(x_3).^2.*5.40564974960243e-10+cos(x_3).^2.*cos(x_6).^2.*sin(x_3).^2.*5.40564974960243e-10)-(x_7.*x_9.*cos(x_3).*cos(x_5).*sin(x_3).^3.*sin(x_5).^3.*5.998516123203674e-18)./(cos(x_3).^4.*1.5163227196875e-5+sin(x_3).^4.*1.5163227196875e-5+cos(x_3).^4.*cos(x_4).^2.*2.702824874801215e-10+cos(x_3).^4.*cos(x_5).^2.*2.702824874801215e-10+cos(x_3).^4.*cos(x_6).^2.*2.702824874801215e-10+cos(x_3).^2.*sin(x_3).^2.*3.032645439375e-5+cos(x_4).^2.*sin(x_3).^4.*2.702824874801215e-10+cos(x_5).^2.*sin(x_3).^4.*2.702824874801215e-10+cos(x_6).^2.*sin(x_3).^4.*2.702824874801215e-10+cos(x_3).^2.*cos(x_4).^2.*sin(x_3).^2.*5.40564974960243e-10+cos(x_3).^2.*cos(x_5).^2.*sin(x_3).^2.*5.40564974960243e-10+cos(x_3).^2.*cos(x_6).^2.*sin(x_3).^2.*5.40564974960243e-10)+(x_7.*x_9.*cos(x_3).^2.*cos(x_6).*sin(x_3).^2.*sin(x_6).*9.017647217594503e-14)./(cos(x_3).^4.*1.5163227196875e-5+sin(x_3).^4.*1.5163227196875e-5+cos(x_3).^4.*cos(x_4).^2.*2.702824874801215e-10+cos(x_3).^4.*cos(x_5).^2.*2.702824874801215e-10+cos(x_3).^4.*cos(x_6).^2.*2.702824874801215e-10+cos(x_3).^2.*sin(x_3).^2.*3.032645439375e-5+cos(x_4).^2.*sin(x_3).^4.*2.702824874801215e-10+cos(x_5).^2.*sin(x_3).^4.*2.702824874801215e-10+cos(x_6).^2.*sin(x_3).^4.*2.702824874801215e-10+cos(x_3).^2.*cos(x_4).^2.*sin(x_3).^2.*5.40564974960243e-10+cos(x_3).^2.*cos(x_5).^2.*sin(x_3).^2.*5.40564974960243e-10+cos(x_3).^2.*cos(x_6).^2.*sin(x_3).^2.*5.40564974960243e-10)-(x_7.*x_9.*cos(x_3).^3.*cos(x_5).*sin(x_3).*sin(x_5).^3.*5.998516123203674e-18)./(cos(x_3).^4.*1.5163227196875e-5+sin(x_3).^4.*1.5163227196875e-5+cos(x_3).^4.*cos(x_4).^2.*2.702824874801215e-10+cos(x_3).^4.*cos(x_5).^2.*2.702824874801215e-10+cos(x_3).^4.*cos(x_6).^2.*2.702824874801215e-10+cos(x_3).^2.*sin(x_3).^2.*3.032645439375e-5+cos(x_4).^2.*sin(x_3).^4.*2.702824874801215e-10+cos(x_5).^2.*sin(x_3).^4.*2.702824874801215e-10+cos(x_6).^2.*sin(x_3).^4.*2.702824874801215e-10+cos(x_3).^2.*cos(x_4).^2.*sin(x_3).^2.*5.40564974960243e-10+cos(x_3).^2.*cos(x_5).^2.*sin(x_3).^2.*5.40564974960243e-10+cos(x_3).^2.*cos(x_6).^2.*sin(x_3).^2.*5.40564974960243e-10)+(x_7.*x_9.*cos(x_3).^4.*cos(x_5).*sin(x_4).^2.*sin(x_5).*3.802906837100583e-18)./(cos(x_3).^4.*1.5163227196875e-5+sin(x_3).^4.*1.5163227196875e-5+cos(x_3).^4.*cos(x_4).^2.*2.702824874801215e-10+cos(x_3).^4.*cos(x_5).^2.*2.702824874801215e-10+cos(x_3).^4.*cos(x_6).^2.*2.702824874801215e-10+cos(x_3).^2.*sin(x_3).^2.*3.032645439375e-5+cos(x_4).^2.*sin(x_3).^4.*2.702824874801215e-10+cos(x_5).^2.*sin(x_3).^4.*2.702824874801215e-10+cos(x_6).^2.*sin(x_3).^4.*2.702824874801215e-10+cos(x_3).^2.*cos(x_4).^2.*sin(x_3).^2.*5.40564974960243e-10+cos(x_3).^2.*cos(x_5).^2.*sin(x_3).^2.*5.40564974960243e-10+cos(x_3).^2.*cos(x_6).^2.*sin(x_3).^2.*5.40564974960243e-10)+(x_8.*x_9.*cos(x_3).*cos(x_5).*sin(x_3).^3.*sin(x_5).^3.*1.607297550997493e-18)./(cos(x_3).^4.*1.5163227196875e-5+sin(x_3).^4.*1.5163227196875e-5+cos(x_3).^4.*cos(x_4).^2.*2.702824874801215e-10+cos(x_3).^4.*cos(x_5).^2.*2.702824874801215e-10+cos(x_3).^4.*cos(x_6).^2.*2.702824874801215e-10+cos(x_3).^2.*sin(x_3).^2.*3.032645439375e-5+cos(x_4).^2.*sin(x_3).^4.*2.702824874801215e-10+cos(x_5).^2.*sin(x_3).^4.*2.702824874801215e-10+cos(x_6).^2.*sin(x_3).^4.*2.702824874801215e-10+cos(x_3).^2.*cos(x_4).^2.*sin(x_3).^2.*5.40564974960243e-10+cos(x_3).^2.*cos(x_5).^2.*sin(x_3).^2.*5.40564974960243e-10+cos(x_3).^2.*cos(x_6).^2.*sin(x_3).^2.*5.40564974960243e-10)-(x_8.*x_9.*cos(x_3).^2.*cos(x_6).*sin(x_3).^2.*sin(x_6).*3.36543175807948e-13)./(cos(x_3).^4.*1.5163227196875e-5+sin(x_3).^4.*1.5163227196875e-5+cos(x_3).^4.*cos(x_4).^2.*2.702824874801215e-10+cos(x_3).^4.*cos(x_5).^2.*2.702824874801215e-10+cos(x_3).^4.*cos(x_6).^2.*2.702824874801215e-10+cos(x_3).^2.*sin(x_3).^2.*3.032645439375e-5+cos(x_4).^2.*sin(x_3).^4.*2.702824874801215e-10+cos(x_5).^2.*sin(x_3).^4.*2.702824874801215e-10+cos(x_6).^2.*sin(x_3).^4.*2.702824874801215e-10+cos(x_3).^2.*cos(x_4).^2.*sin(x_3).^2.*5.40564974960243e-10+cos(x_3).^2.*cos(x_5).^2.*sin(x_3).^2.*5.40564974960243e-10+cos(x_3).^2.*cos(x_6).^2.*sin(x_3).^2.*5.40564974960243e-10)+(x_8.*x_9.*cos(x_3).^3.*cos(x_5).*sin(x_3).*sin(x_5).^3.*1.607297550997493e-18)./(cos(x_3).^4.*1.5163227196875e-5+sin(x_3).^4.*1.5163227196875e-5+cos(x_3).^4.*cos(x_4).^2.*2.702824874801215e-10+cos(x_3).^4.*cos(x_5).^2.*2.702824874801215e-10+cos(x_3).^4.*cos(x_6).^2.*2.702824874801215e-10+cos(x_3).^2.*sin(x_3).^2.*3.032645439375e-5+cos(x_4).^2.*sin(x_3).^4.*2.702824874801215e-10+cos(x_5).^2.*sin(x_3).^4.*2.702824874801215e-10+cos(x_6).^2.*sin(x_3).^4.*2.702824874801215e-10+cos(x_3).^2.*cos(x_4).^2.*sin(x_3).^2.*5.40564974960243e-10+cos(x_3).^2.*cos(x_5).^2.*sin(x_3).^2.*5.40564974960243e-10+cos(x_3).^2.*cos(x_6).^2.*sin(x_3).^2.*5.40564974960243e-10)-(x_8.*x_9.*cos(x_3).^4.*cos(x_4).*sin(x_4).*sin(x_5).^2.*4.39121857220618e-18)./(cos(x_3).^4.*1.5163227196875e-5+sin(x_3).^4.*1.5163227196875e-5+cos(x_3).^4.*cos(x_4).^2.*2.702824874801215e-10+cos(x_3).^4.*cos(x_5).^2.*2.702824874801215e-10+cos(x_3).^4.*cos(x_6).^2.*2.702824874801215e-10+cos(x_3).^2.*sin(x_3).^2.*3.032645439375e-5+cos(x_4).^2.*sin(x_3).^4.*2.702824874801215e-10+cos(x_5).^2.*sin(x_3).^4.*2.702824874801215e-10+cos(x_6).^2.*sin(x_3).^4.*2.702824874801215e-10+cos(x_3).^2.*cos(x_4).^2.*sin(x_3).^2.*5.40564974960243e-10+cos(x_3).^2.*cos(x_5).^2.*sin(x_3).^2.*5.40564974960243e-10+cos(x_3).^2.*cos(x_6).^2.*sin(x_3).^2.*5.40564974960243e-10)+(x_7.*x_9.*cos(x_3).*cos(x_6).*sin(x_3).^3.*sin(x_6).^3.*1.607297550997493e-18)./(cos(x_3).^4.*1.5163227196875e-5+sin(x_3).^4.*1.5163227196875e-5+cos(x_3).^4.*cos(x_4).^2.*2.702824874801215e-10+cos(x_3).^4.*cos(x_5).^2.*2.702824874801215e-10+cos(x_3).^4.*cos(x_6).^2.*2.702824874801215e-10+cos(x_3).^2.*sin(x_3).^2.*3.032645439375e-5+cos(x_4).^2.*sin(x_3).^4.*2.702824874801215e-10+cos(x_5).^2.*sin(x_3).^4.*2.702824874801215e-10+cos(x_6).^2.*sin(x_3).^4.*2.702824874801215e-10+cos(x_3).^2.*cos(x_4).^2.*sin(x_3).^2.*5.40564974960243e-10+cos(x_3).^2.*cos(x_5).^2.*sin(x_3).^2.*5.40564974960243e-10+cos(x_3).^2.*cos(x_6).^2.*sin(x_3).^2.*5.40564974960243e-10)+(x_7.*x_9.*cos(x_3).^3.*cos(x_6).*sin(x_3).*sin(x_6).^3.*1.607297550997493e-18)./(cos(x_3).^4.*1.5163227196875e-5+sin(x_3).^4.*1.5163227196875e-5+cos(x_3).^4.*cos(x_4).^2.*2.702824874801215e-10+cos(x_3).^4.*cos(x_5).^2.*2.702824874801215e-10+cos(x_3).^4.*cos(x_6).^2.*2.702824874801215e-10+cos(x_3).^2.*sin(x_3).^2.*3.032645439375e-5+cos(x_4).^2.*sin(x_3).^4.*2.702824874801215e-10+cos(x_5).^2.*sin(x_3).^4.*2.702824874801215e-10+cos(x_6).^2.*sin(x_3).^4.*2.702824874801215e-10+cos(x_3).^2.*cos(x_4).^2.*sin(x_3).^2.*5.40564974960243e-10+cos(x_3).^2.*cos(x_5).^2.*sin(x_3).^2.*5.40564974960243e-10+cos(x_3).^2.*cos(x_6).^2.*sin(x_3).^2.*5.40564974960243e-10)-(x_8.*x_9.*cos(x_3).^4.*cos(x_4).*sin(x_4).*sin(x_6).^2.*4.39121857220618e-18)./(cos(x_3).^4.*1.5163227196875e-5+sin(x_3).^4.*1.5163227196875e-5+cos(x_3).^4.*cos(x_4).^2.*2.702824874801215e-10+cos(x_3).^4.*cos(x_5).^2.*2.702824874801215e-10+cos(x_3).^4.*cos(x_6).^2.*2.702824874801215e-10+cos(x_3).^2.*sin(x_3).^2.*3.032645439375e-5+cos(x_4).^2.*sin(x_3).^4.*2.702824874801215e-10+cos(x_5).^2.*sin(x_3).^4.*2.702824874801215e-10+cos(x_6).^2.*sin(x_3).^4.*2.702824874801215e-10+cos(x_3).^2.*cos(x_4).^2.*sin(x_3).^2.*5.40564974960243e-10+cos(x_3).^2.*cos(x_5).^2.*sin(x_3).^2.*5.40564974960243e-10+cos(x_3).^2.*cos(x_6).^2.*sin(x_3).^2.*5.40564974960243e-10)+(x_8.*x_9.*cos(x_3).^4.*cos(x_5).*sin(x_4).^2.*sin(x_5).*2.19560928610309e-18)./(cos(x_3).^4.*1.5163227196875e-5+sin(x_3).^4.*1.5163227196875e-5+cos(x_3).^4.*cos(x_4).^2.*2.702824874801215e-10+cos(x_3).^4.*cos(x_5).^2.*2.702824874801215e-10+cos(x_3).^4.*cos(x_6).^2.*2.702824874801215e-10+cos(x_3).^2.*sin(x_3).^2.*3.032645439375e-5+cos(x_4).^2.*sin(x_3).^4.*2.702824874801215e-10+cos(x_5).^2.*sin(x_3).^4.*2.702824874801215e-10+cos(x_6).^2.*sin(x_3).^4.*2.702824874801215e-10+cos(x_3).^2.*cos(x_4).^2.*sin(x_3).^2.*5.40564974960243e-10+cos(x_3).^2.*cos(x_5).^2.*sin(x_3).^2.*5.40564974960243e-10+cos(x_3).^2.*cos(x_6).^2.*sin(x_3).^2.*5.40564974960243e-10)+(x_7.*x_9.*cos(x_3).^4.*cos(x_5).*sin(x_5).*sin(x_6).^2.*3.802906837100583e-18)./(cos(x_3).^4.*1.5163227196875e-5+sin(x_3).^4.*1.5163227196875e-5+cos(x_3).^4.*cos(x_4).^2.*2.702824874801215e-10+cos(x_3).^4.*cos(x_5).^2.*2.702824874801215e-10+cos(x_3).^4.*cos(x_6).^2.*2.702824874801215e-10+cos(x_3).^2.*sin(x_3).^2.*3.032645439375e-5+cos(x_4).^2.*sin(x_3).^4.*2.702824874801215e-10+cos(x_5).^2.*sin(x_3).^4.*2.702824874801215e-10+cos(x_6).^2.*sin(x_3).^4.*2.702824874801215e-10+cos(x_3).^2.*cos(x_4).^2.*sin(x_3).^2.*5.40564974960243e-10+cos(x_3).^2.*cos(x_5).^2.*sin(x_3).^2.*5.40564974960243e-10+cos(x_3).^2.*cos(x_6).^2.*sin(x_3).^2.*5.40564974960243e-10)-(x_7.*x_9.*cos(x_3).^4.*cos(x_6).*sin(x_4).^2.*sin(x_6).*3.802906837100583e-18)./(cos(x_3).^4.*1.5163227196875e-5+sin(x_3).^4.*1.5163227196875e-5+cos(x_3).^4.*cos(x_4).^2.*2.702824874801215e-10+cos(x_3).^4.*cos(x_5).^2.*2.702824874801215e-10+cos(x_3).^4.*cos(x_6).^2.*2.702824874801215e-10+cos(x_3).^2.*sin(x_3).^2.*3.032645439375e-5+cos(x_4).^2.*sin(x_3).^4.*2.702824874801215e-10+cos(x_5).^2.*sin(x_3).^4.*2.702824874801215e-10+cos(x_6).^2.*sin(x_3).^4.*2.702824874801215e-10+cos(x_3).^2.*cos(x_4).^2.*sin(x_3).^2.*5.40564974960243e-10+cos(x_3).^2.*cos(x_5).^2.*sin(x_3).^2.*5.40564974960243e-10+cos(x_3).^2.*cos(x_6).^2.*sin(x_3).^2.*5.40564974960243e-10)-(x_8.*x_9.*cos(x_3).*cos(x_6).*sin(x_3).^3.*sin(x_6).^3.*5.998516123203674e-18)./(cos(x_3).^4.*1.5163227196875e-5+sin(x_3).^4.*1.5163227196875e-5+cos(x_3).^4.*cos(x_4).^2.*2.702824874801215e-10+cos(x_3).^4.*cos(x_5).^2.*2.702824874801215e-10+cos(x_3).^4.*cos(x_6).^2.*2.702824874801215e-10+cos(x_3).^2.*sin(x_3).^2.*3.032645439375e-5+cos(x_4).^2.*sin(x_3).^4.*2.702824874801215e-10+cos(x_5).^2.*sin(x_3).^4.*2.702824874801215e-10+cos(x_6).^2.*sin(x_3).^4.*2.702824874801215e-10+cos(x_3).^2.*cos(x_4).^2.*sin(x_3).^2.*5.40564974960243e-10+cos(x_3).^2.*cos(x_5).^2.*sin(x_3).^2.*5.40564974960243e-10+cos(x_3).^2.*cos(x_6).^2.*sin(x_3).^2.*5.40564974960243e-10)-(x_8.*x_9.*cos(x_3).^3.*cos(x_6).*sin(x_3).*sin(x_6).^3.*5.998516123203674e-18)./(cos(x_3).^4.*1.5163227196875e-5+sin(x_3).^4.*1.5163227196875e-5+cos(x_3).^4.*cos(x_4).^2.*2.702824874801215e-10+cos(x_3).^4.*cos(x_5).^2.*2.702824874801215e-10+cos(x_3).^4.*cos(x_6).^2.*2.702824874801215e-10+cos(x_3).^2.*sin(x_3).^2.*3.032645439375e-5+cos(x_4).^2.*sin(x_3).^4.*2.702824874801215e-10+cos(x_5).^2.*sin(x_3).^4.*2.702824874801215e-10+cos(x_6).^2.*sin(x_3).^4.*2.702824874801215e-10+cos(x_3).^2.*cos(x_4).^2.*sin(x_3).^2.*5.40564974960243e-10+cos(x_3).^2.*cos(x_5).^2.*sin(x_3).^2.*5.40564974960243e-10+cos(x_3).^2.*cos(x_6).^2.*sin(x_3).^2.*5.40564974960243e-10)-(x_7.*x_9.*cos(x_3).^4.*cos(x_6).*sin(x_5).^2.*sin(x_6).*3.802906837100583e-18)./(cos(x_3).^4.*1.5163227196875e-5+sin(x_3).^4.*1.5163227196875e-5+cos(x_3).^4.*cos(x_4).^2.*2.702824874801215e-10+cos(x_3).^4.*cos(x_5).^2.*2.702824874801215e-10+cos(x_3).^4.*cos(x_6).^2.*2.702824874801215e-10+cos(x_3).^2.*sin(x_3).^2.*3.032645439375e-5+cos(x_4).^2.*sin(x_3).^4.*2.702824874801215e-10+cos(x_5).^2.*sin(x_3).^4.*2.702824874801215e-10+cos(x_6).^2.*sin(x_3).^4.*2.702824874801215e-10+cos(x_3).^2.*cos(x_4).^2.*sin(x_3).^2.*5.40564974960243e-10+cos(x_3).^2.*cos(x_5).^2.*sin(x_3).^2.*5.40564974960243e-10+cos(x_3).^2.*cos(x_6).^2.*sin(x_3).^2.*5.40564974960243e-10)+(x_8.*x_9.*cos(x_3).^4.*cos(x_5).*sin(x_5).*sin(x_6).^2.*2.19560928610309e-18)./(cos(x_3).^4.*1.5163227196875e-5+sin(x_3).^4.*1.5163227196875e-5+cos(x_3).^4.*cos(x_4).^2.*2.702824874801215e-10+cos(x_3).^4.*cos(x_5).^2.*2.702824874801215e-10+cos(x_3).^4.*cos(x_6).^2.*2.702824874801215e-10+cos(x_3).^2.*sin(x_3).^2.*3.032645439375e-5+cos(x_4).^2.*sin(x_3).^4.*2.702824874801215e-10+cos(x_5).^2.*sin(x_3).^4.*2.702824874801215e-10+cos(x_6).^2.*sin(x_3).^4.*2.702824874801215e-10+cos(x_3).^2.*cos(x_4).^2.*sin(x_3).^2.*5.40564974960243e-10+cos(x_3).^2.*cos(x_5).^2.*sin(x_3).^2.*5.40564974960243e-10+cos(x_3).^2.*cos(x_6).^2.*sin(x_3).^2.*5.40564974960243e-10)+(x_8.*x_9.*cos(x_3).^4.*cos(x_6).*sin(x_4).^2.*sin(x_6).*2.19560928610309e-18)./(cos(x_3).^4.*1.5163227196875e-5+sin(x_3).^4.*1.5163227196875e-5+cos(x_3).^4.*cos(x_4).^2.*2.702824874801215e-10+cos(x_3).^4.*cos(x_5).^2.*2.702824874801215e-10+cos(x_3).^4.*cos(x_6).^2.*2.702824874801215e-10+cos(x_3).^2.*sin(x_3).^2.*3.032645439375e-5+cos(x_4).^2.*sin(x_3).^4.*2.702824874801215e-10+cos(x_5).^2.*sin(x_3).^4.*2.702824874801215e-10+cos(x_6).^2.*sin(x_3).^4.*2.702824874801215e-10+cos(x_3).^2.*cos(x_4).^2.*sin(x_3).^2.*5.40564974960243e-10+cos(x_3).^2.*cos(x_5).^2.*sin(x_3).^2.*5.40564974960243e-10+cos(x_3).^2.*cos(x_6).^2.*sin(x_3).^2.*5.40564974960243e-10)+(x_8.*x_9.*cos(x_3).^4.*cos(x_6).*sin(x_5).^2.*sin(x_6).*2.19560928610309e-18)./(cos(x_3).^4.*1.5163227196875e-5+sin(x_3).^4.*1.5163227196875e-5+cos(x_3).^4.*cos(x_4).^2.*2.702824874801215e-10+cos(x_3).^4.*cos(x_5).^2.*2.702824874801215e-10+cos(x_3).^4.*cos(x_6).^2.*2.702824874801215e-10+cos(x_3).^2.*sin(x_3).^2.*3.032645439375e-5+cos(x_4).^2.*sin(x_3).^4.*2.702824874801215e-10+cos(x_5).^2.*sin(x_3).^4.*2.702824874801215e-10+cos(x_6).^2.*sin(x_3).^4.*2.702824874801215e-10+cos(x_3).^2.*cos(x_4).^2.*sin(x_3).^2.*5.40564974960243e-10+cos(x_3).^2.*cos(x_5).^2.*sin(x_3).^2.*5.40564974960243e-10+cos(x_3).^2.*cos(x_6).^2.*sin(x_3).^2.*5.40564974960243e-10)+(x_7.*x_9.*cos(x_4).*sin(x_3).^5.*sin(x_4).*sin(x_5).^2.*1.470104929075305e-19)./(cos(x_3).^4.*3.79080679921875e-6+sin(x_3).^4.*3.79080679921875e-6+cos(x_3).^4.*cos(x_4).^2.*6.757062187003037e-11+cos(x_3).^4.*cos(x_5).^2.*6.757062187003037e-11+cos(x_3).^4.*cos(x_6).^2.*6.757062187003037e-11+cos(x_3).^2.*sin(x_3).^2.*7.5816135984375e-6+cos(x_4).^2.*sin(x_3).^4.*6.757062187003037e-11+cos(x_5).^2.*sin(x_3).^4.*6.757062187003037e-11+cos(x_6).^2.*sin(x_3).^4.*6.757062187003037e-11+cos(x_3).^2.*cos(x_4).^2.*sin(x_3).^2.*1.351412437400607e-10+cos(x_3).^2.*cos(x_5).^2.*sin(x_3).^2.*1.351412437400607e-10+cos(x_3).^2.*cos(x_6).^2.*sin(x_3).^2.*1.351412437400607e-10)+(x_7.*x_9.*cos(x_4).*sin(x_3).^5.*sin(x_4).*sin(x_6).^2.*1.470104929075305e-19)./(cos(x_3).^4.*3.79080679921875e-6+sin(x_3).^4.*3.79080679921875e-6+cos(x_3).^4.*cos(x_4).^2.*6.757062187003037e-11+cos(x_3).^4.*cos(x_5).^2.*6.757062187003037e-11+cos(x_3).^4.*cos(x_6).^2.*6.757062187003037e-11+cos(x_3).^2.*sin(x_3).^2.*7.5816135984375e-6+cos(x_4).^2.*sin(x_3).^4.*6.757062187003037e-11+cos(x_5).^2.*sin(x_3).^4.*6.757062187003037e-11+cos(x_6).^2.*sin(x_3).^4.*6.757062187003037e-11+cos(x_3).^2.*cos(x_4).^2.*sin(x_3).^2.*1.351412437400607e-10+cos(x_3).^2.*cos(x_5).^2.*sin(x_3).^2.*1.351412437400607e-10+cos(x_3).^2.*cos(x_6).^2.*sin(x_3).^2.*1.351412437400607e-10)-(x_7.*x_9.*cos(x_5).*sin(x_3).^5.*sin(x_4).^2.*sin(x_5).*7.350524645376524e-20)./(cos(x_3).^4.*3.79080679921875e-6+sin(x_3).^4.*3.79080679921875e-6+cos(x_3).^4.*cos(x_4).^2.*6.757062187003037e-11+cos(x_3).^4.*cos(x_5).^2.*6.757062187003037e-11+cos(x_3).^4.*cos(x_6).^2.*6.757062187003037e-11+cos(x_3).^2.*sin(x_3).^2.*7.5816135984375e-6+cos(x_4).^2.*sin(x_3).^4.*6.757062187003037e-11+cos(x_5).^2.*sin(x_3).^4.*6.757062187003037e-11+cos(x_6).^2.*sin(x_3).^4.*6.757062187003037e-11+cos(x_3).^2.*cos(x_4).^2.*sin(x_3).^2.*1.351412437400607e-10+cos(x_3).^2.*cos(x_5).^2.*sin(x_3).^2.*1.351412437400607e-10+cos(x_3).^2.*cos(x_6).^2.*sin(x_3).^2.*1.351412437400607e-10)-(x_7.*x_9.*cos(x_4).*sin(x_3).^5.*sin(x_4).*sin(x_5).^4.*1.310151082203454e-24)./(cos(x_3).^4.*3.79080679921875e-6+sin(x_3).^4.*3.79080679921875e-6+cos(x_3).^4.*cos(x_4).^2.*6.757062187003037e-11+cos(x_3).^4.*cos(x_5).^2.*6.757062187003037e-11+cos(x_3).^4.*cos(x_6).^2.*6.757062187003037e-11+cos(x_3).^2.*sin(x_3).^2.*7.5816135984375e-6+cos(x_4).^2.*sin(x_3).^4.*6.757062187003037e-11+cos(x_5).^2.*sin(x_3).^4.*6.757062187003037e-11+cos(x_6).^2.*sin(x_3).^4.*6.757062187003037e-11+cos(x_3).^2.*cos(x_4).^2.*sin(x_3).^2.*1.351412437400607e-10+cos(x_3).^2.*cos(x_5).^2.*sin(x_3).^2.*1.351412437400607e-10+cos(x_3).^2.*cos(x_6).^2.*sin(x_3).^2.*1.351412437400607e-10)+(x_8.*x_9.*cos(x_5).*sin(x_3).^5.*sin(x_4).^2.*sin(x_5).*1.273148214807934e-19)./(cos(x_3).^4.*3.79080679921875e-6+sin(x_3).^4.*3.79080679921875e-6+cos(x_3).^4.*cos(x_4).^2.*6.757062187003037e-11+cos(x_3).^4.*cos(x_5).^2.*6.757062187003037e-11+cos(x_3).^4.*cos(x_6).^2.*6.757062187003037e-11+cos(x_3).^2.*sin(x_3).^2.*7.5816135984375e-6+cos(x_4).^2.*sin(x_3).^4.*6.757062187003037e-11+cos(x_5).^2.*sin(x_3).^4.*6.757062187003037e-11+cos(x_6).^2.*sin(x_3).^4.*6.757062187003037e-11+cos(x_3).^2.*cos(x_4).^2.*sin(x_3).^2.*1.351412437400607e-10+cos(x_3).^2.*cos(x_5).^2.*sin(x_3).^2.*1.351412437400607e-10+cos(x_3).^2.*cos(x_6).^2.*sin(x_3).^2.*1.351412437400607e-10)-(x_7.*x_9.*cos(x_4).*sin(x_3).^5.*sin(x_4).*sin(x_6).^4.*1.310151082203454e-24)./(cos(x_3).^4.*3.79080679921875e-6+sin(x_3).^4.*3.79080679921875e-6+cos(x_3).^4.*cos(x_4).^2.*6.757062187003037e-11+cos(x_3).^4.*cos(x_5).^2.*6.757062187003037e-11+cos(x_3).^4.*cos(x_6).^2.*6.757062187003037e-11+cos(x_3).^2.*sin(x_3).^2.*7.5816135984375e-6+cos(x_4).^2.*sin(x_3).^4.*6.757062187003037e-11+cos(x_5).^2.*sin(x_3).^4.*6.757062187003037e-11+cos(x_6).^2.*sin(x_3).^4.*6.757062187003037e-11+cos(x_3).^2.*cos(x_4).^2.*sin(x_3).^2.*1.351412437400607e-10+cos(x_3).^2.*cos(x_5).^2.*sin(x_3).^2.*1.351412437400607e-10+cos(x_3).^2.*cos(x_6).^2.*sin(x_3).^2.*1.351412437400607e-10)-(x_7.*x_9.*cos(x_5).*sin(x_3).^5.*sin(x_5).*sin(x_6).^2.*7.350524645376524e-20)./(cos(x_3).^4.*3.79080679921875e-6+sin(x_3).^4.*3.79080679921875e-6+cos(x_3).^4.*cos(x_4).^2.*6.757062187003037e-11+cos(x_3).^4.*cos(x_5).^2.*6.757062187003037e-11+cos(x_3).^4.*cos(x_6).^2.*6.757062187003037e-11+cos(x_3).^2.*sin(x_3).^2.*7.5816135984375e-6+cos(x_4).^2.*sin(x_3).^4.*6.757062187003037e-11+cos(x_5).^2.*sin(x_3).^4.*6.757062187003037e-11+cos(x_6).^2.*sin(x_3).^4.*6.757062187003037e-11+cos(x_3).^2.*cos(x_4).^2.*sin(x_3).^2.*1.351412437400607e-10+cos(x_3).^2.*cos(x_5).^2.*sin(x_3).^2.*1.351412437400607e-10+cos(x_3).^2.*cos(x_6).^2.*sin(x_3).^2.*1.351412437400607e-10)+(x_7.*x_9.*cos(x_5).*sin(x_3).^5.*sin(x_4).^4.*sin(x_5).*6.550755411017271e-25)./(cos(x_3).^4.*3.79080679921875e-6+sin(x_3).^4.*3.79080679921875e-6+cos(x_3).^4.*cos(x_4).^2.*6.757062187003037e-11+cos(x_3).^4.*cos(x_5).^2.*6.757062187003037e-11+cos(x_3).^4.*cos(x_6).^2.*6.757062187003037e-11+cos(x_3).^2.*sin(x_3).^2.*7.5816135984375e-6+cos(x_4).^2.*sin(x_3).^4.*6.757062187003037e-11+cos(x_5).^2.*sin(x_3).^4.*6.757062187003037e-11+cos(x_6).^2.*sin(x_3).^4.*6.757062187003037e-11+cos(x_3).^2.*cos(x_4).^2.*sin(x_3).^2.*1.351412437400607e-10+cos(x_3).^2.*cos(x_5).^2.*sin(x_3).^2.*1.351412437400607e-10+cos(x_3).^2.*cos(x_6).^2.*sin(x_3).^2.*1.351412437400607e-10)-(x_7.*x_9.*cos(x_6).*sin(x_3).^5.*sin(x_4).^2.*sin(x_6).*7.350524645376524e-20)./(cos(x_3).^4.*3.79080679921875e-6+sin(x_3).^4.*3.79080679921875e-6+cos(x_3).^4.*cos(x_4).^2.*6.757062187003037e-11+cos(x_3).^4.*cos(x_5).^2.*6.757062187003037e-11+cos(x_3).^4.*cos(x_6).^2.*6.757062187003037e-11+cos(x_3).^2.*sin(x_3).^2.*7.5816135984375e-6+cos(x_4).^2.*sin(x_3).^4.*6.757062187003037e-11+cos(x_5).^2.*sin(x_3).^4.*6.757062187003037e-11+cos(x_6).^2.*sin(x_3).^4.*6.757062187003037e-11+cos(x_3).^2.*cos(x_4).^2.*sin(x_3).^2.*1.351412437400607e-10+cos(x_3).^2.*cos(x_5).^2.*sin(x_3).^2.*1.351412437400607e-10+cos(x_3).^2.*cos(x_6).^2.*sin(x_3).^2.*1.351412437400607e-10)-(x_7.*x_9.*cos(x_6).*sin(x_3).^5.*sin(x_5).^2.*sin(x_6).*7.350524645376524e-20)./(cos(x_3).^4.*3.79080679921875e-6+sin(x_3).^4.*3.79080679921875e-6+cos(x_3).^4.*cos(x_4).^2.*6.757062187003037e-11+cos(x_3).^4.*cos(x_5).^2.*6.757062187003037e-11+cos(x_3).^4.*cos(x_6).^2.*6.757062187003037e-11+cos(x_3).^2.*sin(x_3).^2.*7.5816135984375e-6+cos(x_4).^2.*sin(x_3).^4.*6.757062187003037e-11+cos(x_5).^2.*sin(x_3).^4.*6.757062187003037e-11+cos(x_6).^2.*sin(x_3).^4.*6.757062187003037e-11+cos(x_3).^2.*cos(x_4).^2.*sin(x_3).^2.*1.351412437400607e-10+cos(x_3).^2.*cos(x_5).^2.*sin(x_3).^2.*1.351412437400607e-10+cos(x_3).^2.*cos(x_6).^2.*sin(x_3).^2.*1.351412437400607e-10)+(x_8.*x_9.*cos(x_5).*sin(x_3).^5.*sin(x_5).*sin(x_6).^2.*1.273148214807934e-19)./(cos(x_3).^4.*3.79080679921875e-6+sin(x_3).^4.*3.79080679921875e-6+cos(x_3).^4.*cos(x_4).^2.*6.757062187003037e-11+cos(x_3).^4.*cos(x_5).^2.*6.757062187003037e-11+cos(x_3).^4.*cos(x_6).^2.*6.757062187003037e-11+cos(x_3).^2.*sin(x_3).^2.*7.5816135984375e-6+cos(x_4).^2.*sin(x_3).^4.*6.757062187003037e-11+cos(x_5).^2.*sin(x_3).^4.*6.757062187003037e-11+cos(x_6).^2.*sin(x_3).^4.*6.757062187003037e-11+cos(x_3).^2.*cos(x_4).^2.*sin(x_3).^2.*1.351412437400607e-10+cos(x_3).^2.*cos(x_5).^2.*sin(x_3).^2.*1.351412437400607e-10+cos(x_3).^2.*cos(x_6).^2.*sin(x_3).^2.*1.351412437400607e-10)-(x_8.*x_9.*cos(x_5).*sin(x_3).^5.*sin(x_4).^4.*sin(x_5).*1.134624119983866e-24)./(cos(x_3).^4.*3.79080679921875e-6+sin(x_3).^4.*3.79080679921875e-6+cos(x_3).^4.*cos(x_4).^2.*6.757062187003037e-11+cos(x_3).^4.*cos(x_5).^2.*6.757062187003037e-11+cos(x_3).^4.*cos(x_6).^2.*6.757062187003037e-11+cos(x_3).^2.*sin(x_3).^2.*7.5816135984375e-6+cos(x_4).^2.*sin(x_3).^4.*6.757062187003037e-11+cos(x_5).^2.*sin(x_3).^4.*6.757062187003037e-11+cos(x_6).^2.*sin(x_3).^4.*6.757062187003037e-11+cos(x_3).^2.*cos(x_4).^2.*sin(x_3).^2.*1.351412437400607e-10+cos(x_3).^2.*